simulink model "COMPONENT_MDL_Lag_QUAD_and_PEND_with_Ab"  (R2020b)
(part 10 of 12)

_Psi_D-THE_Phi_D.*sin(THE_Theta))))./2.0+(cg_to_mot_L.*cos(THE_Psi).*cos(THE_Theta).*(THE_Theta_D.*cos(THE_Psi)+THE_Phi_D.*cos(THE_Theta).*sin(THE_Psi)))./2.0)+THE_Psi_D.*cg_to_mot_H.*mprop.*cos(THE_Psi).*cos(THE_Theta).*(THE_Z_D./2.0-(cg_to_mot_H.*sin(THE_Theta).*(THE_Theta_D.*cos(THE_Psi)+THE_Phi_D.*cos(THE_Theta).*sin(THE_Psi)))./2.0+(cos(THE_Theta).*sin(THE_Psi).*(cg_to_mot_L.*(THE_Theta_D.*sin(THE_Psi)-THE_Phi_D.*cos(THE_Psi).*cos(THE_Theta))-cg_to_mot_H.*(THE_Psi_D-THE_Phi_D.*sin(THE_Theta))))./2.0+(cg_to_mot_L.*cos(THE_Psi).*cos(THE_Theta).*(THE_Theta_D.*cos(THE_Psi)+THE_Phi_D.*cos(THE_Theta).*sin(THE_Psi)))./2.0)+(THE_Theta_D.*cg_to_mot_H.*mprop.*sin(THE_Psi).*sin(THE_Theta).*(-THE_Z_D+cg_to_mot_H.*sin(THE_Theta).*(THE_Theta_D.*cos(THE_Psi)+THE_Phi_D.*cos(THE_Theta).*sin(THE_Psi))+cos(THE_Theta).*sin(THE_Psi).*(cg_to_mot_L.*(THE_Theta_D.*sin(THE_Psi)-THE_Phi_D.*cos(THE_Psi).*cos(THE_Theta))+cg_to_mot_H.*(THE_Psi_D-THE_Phi_D.*sin(THE_Theta)))+cg_to_mot_L.*cos(THE_Psi).*cos(THE_Theta).*(THE_Theta_D.*cos(THE_Psi)+THE_Phi_D.*cos(THE_Theta).*sin(THE_Psi))))./2.0+THE_Theta_D.*cg_to_mot_H.*mprop.*sin(THE_Psi).*sin(THE_Theta).*(THE_Z_D.*(-1.0./2.0)+(cg_to_mot_H.*sin(THE_Theta).*(THE_Theta_D.*cos(THE_Psi)+THE_Phi_D.*cos(THE_Theta).*sin(THE_Psi)))./2.0+(cos(THE_Theta).*sin(THE_Psi).*(cg_to_mot_L.*(THE_Theta_D.*sin(THE_Psi)-THE_Phi_D.*cos(THE_Psi).*cos(THE_Theta))+cg_to_mot_H.*(THE_Psi_D-THE_Phi_D.*sin(THE_Theta))))./2.0+(cg_to_mot_L.*cos(THE_Psi).*cos(THE_Theta).*(THE_Theta_D.*cos(THE_Psi)+THE_Phi_D.*cos(THE_Theta).*sin(THE_Psi)))./2.0)-THE_Theta_D.*cg_to_mot_H.*mprop.*sin(THE_Psi).*sin(THE_Theta).*(THE_Z_D./2.0-(cg_to_mot_H.*sin(THE_Theta).*(THE_Theta_D.*cos(THE_Psi)+THE_Phi_D.*cos(THE_Theta).*sin(THE_Psi)))./2.0+(cos(THE_Theta).*sin(THE_Psi).*(cg_to_mot_L.*(THE_Theta_D.*sin(THE_Psi)-THE_Phi_D.*cos(THE_Psi).*cos(THE_Theta))-cg_to_mot_H.*(THE_Psi_D-THE_Phi_D.*sin(THE_Theta))))./2.0+(cg_to_mot_L.*cos(THE_Psi).*cos(THE_Theta).*(THE_Theta_D.*cos(THE_Psi)+THE_Phi_D.*cos(THE_Theta).*sin(THE_Psi)))./2.0);Tbz_1.*(sin(THE_Phi).*sin(THE_Psi)+cos(THE_Phi).*cos(THE_Psi).*sin(THE_Theta))+Tbz_2.*(sin(THE_Phi).*sin(THE_Psi)+cos(THE_Phi).*cos(THE_Psi).*sin(THE_Theta))+Tbz_3.*(sin(THE_Phi).*sin(THE_Psi)+cos(THE_Phi).*cos(THE_Psi).*sin(THE_Theta))+Tbz_4.*(sin(THE_Phi).*sin(THE_Psi)+cos(THE_Phi).*cos(THE_Psi).*sin(THE_Theta))+(mprop.*(cos(THE_Phi).*cos(THE_Theta).*(cg_to_mot_H.*(THE_Psi_D.*THE_Theta_D.*sin(THE_Psi)-THE_Phi_D.*THE_Psi_D.*cos(THE_Psi).*cos(THE_Theta)+THE_Phi_D.*THE_Theta_D.*sin(THE_Psi).*sin(THE_Theta))-cg_to_mot_L.*(THE_Psi_D.*THE_Theta_D.*cos(THE_Psi)+THE_Phi_D.*THE_Psi_D.*cos(THE_Theta).*sin(THE_Psi)+THE_Phi_D.*THE_Theta_D.*cos(THE_Psi).*sin(THE_Theta)))-cg_to_mot_L.*(THE_Psi_D-THE_Phi_D.*sin(THE_Theta)).*(THE_Phi_D.*cos(THE_Phi).*sin(THE_Psi)+THE_Psi_D.*cos(THE_Psi).*sin(THE_Phi)+THE_Theta_D.*cos(THE_Phi).*cos(THE_Psi).*cos(THE_Theta)-THE_Phi_D.*cos(THE_Psi).*sin(THE_Phi).*sin(THE_Theta)-THE_Psi_D.*cos(THE_Phi).*sin(THE_Psi).*sin(THE_Theta))+cg_to_mot_H.*(THE_Psi_D-THE_Phi_D.*sin(THE_Theta)).*(-THE_Phi_D.*cos(THE_Phi).*cos(THE_Psi)+THE_Psi_D.*sin(THE_Phi).*sin(THE_Psi)-THE_Phi_D.*sin(THE_Phi).*sin(THE_Psi).*sin(THE_Theta)+THE_Psi_D.*cos(THE_Phi).*cos(THE_Psi).*sin(THE_Theta)+THE_Theta_D.*cos(THE_Phi).*cos(THE_Theta).*sin(THE_Psi))+THE_Phi_D.*cos(THE_Theta).*sin(THE_Phi).*(cg_to_mot_H.*(THE_Theta_D.*cos(THE_Psi)+THE_Phi_D.*cos(THE_Theta).*sin(THE_Psi))+cg_to_mot_L.*(THE_Theta_D.*sin(THE_Psi)-THE_Phi_D.*cos(THE_Psi).*cos(THE_Theta)))+THE_Theta_D.*cos(THE_Phi).*sin(THE_Theta).*(cg_to_mot_H.*(THE_Theta_D.*cos(THE_Psi)+THE_Phi_D.*cos(THE_Theta).*sin(THE_Psi))+cg_to_mot_L.*(THE_Theta_D.*sin(THE_Psi)-THE_Phi_D.*cos(THE_Psi).*cos(THE_Theta)))+THE_Phi_D.*THE_Theta_D.*cg_to_mot_H.*cos(THE_Theta).*(cos(THE_Psi).*sin(THE_Phi)-cos(THE_Phi).*sin(THE_Psi).*sin(THE_Theta))+THE_Phi_D.*THE_Theta_D.*cg_to_mot_L.*cos(THE_Theta).*(sin(THE_Phi).*sin(THE_Psi)+cos(THE_Phi).*cos(THE_Psi).*sin(THE_Theta))))./2.0+(mprop.*(cos(THE_Phi).*cos(THE_Theta).*(cg_to_mot_H.*(THE_Psi_D.*THE_Theta_D.*sin(THE_Psi)-THE_Phi_D.*THE_Psi_D.*cos(THE_Psi).*cos(THE_Theta)+THE_Phi_D.*THE_Theta_D.*sin(THE_Psi).*sin(THE_Theta))+cg_to_mot_L.*(THE_Psi_D.*THE_Theta_D.*cos(THE_Psi)+THE_Phi_D.*THE_Psi_D.*cos(THE_Theta).*sin(THE_Psi)+THE_Phi_D.*THE_Theta_D.*cos(THE_Psi).*sin(THE_Theta)))+cg_to_mot_L.*(THE_Psi_D-THE_Phi_D.*sin(THE_Theta)).*(THE_Phi_D.*cos(THE_Phi).*sin(THE_Psi)+THE_Psi_D.*cos(THE_Psi).*sin(THE_Phi)+THE_Theta_D.*cos(THE_Phi).*cos(THE_Psi).*cos(THE_Theta)-THE_Phi_D.*cos(THE_Psi).*sin(THE_Phi).*sin(THE_Theta)-THE_Psi_D.*cos(THE_Phi).*sin(THE_Psi).*sin(THE_Theta))+cg_to_mot_H.*(THE_Psi_D-THE_Phi_D.*sin(THE_Theta)).*(-THE_Phi_D.*cos(THE_Phi).*cos(THE_Psi)+THE_Psi_D.*sin(THE_Phi).*sin(THE_Psi)-THE_Phi_D.*sin(THE_Phi).*sin(THE_Psi).*sin(THE_Theta)+THE_Psi_D.*cos(THE_Phi).*cos(THE_Psi).*sin(THE_Theta)+THE_Theta_D.*cos(THE_Phi).*cos(THE_Theta).*sin(THE_Psi))+THE_Phi_D.*cos(THE_Theta).*sin(THE_Phi).*(cg_to_mot_H.*(THE_Theta_D.*cos(THE_Psi)+THE_Phi_D.*cos(THE_Theta).*sin(THE_Psi))-cg_to_mot_L.*(THE_Theta_D.*sin(THE_Psi)-THE_Phi_D.*cos(THE_Psi).*cos(THE_Theta)))+THE_Theta_D.*cos(THE_Phi).*sin(THE_Theta).*(cg_to_mot_H.*(THE_Theta_D.*cos(THE_Psi)+THE_Phi_D.*cos(THE_Theta).*sin(THE_Psi))-cg_to_mot_L.*(THE_Theta_D.*sin(THE_Psi)-THE_Phi_D.*cos(THE_Psi).*cos(THE_Theta)))+THE_Phi_D.*THE_Theta_D.*cg_to_mot_H.*cos(THE_Theta).*(cos(THE_Psi).*sin(THE_Phi)-cos(THE_Phi).*sin(THE_Psi).*sin(THE_Theta))-THE_Phi_D.*THE_Theta_D.*cg_to_mot_L.*cos(THE_Theta).*(sin(THE_Phi).*sin(THE_Psi)+cos(THE_Phi).*cos(THE_Psi).*sin(THE_Theta))))./2.0+mprop.*((cos(THE_Phi).*cos(THE_Theta).*(cg_to_mot_H.*(THE_Psi_D.*THE_Theta_D.*sin(THE_Psi)-THE_Phi_D.*THE_Psi_D.*cos(THE_Psi).*cos(THE_Theta)+THE_Phi_D.*THE_Theta_D.*sin(THE_Psi).*sin(THE_Theta))-cg_to_mot_L.*(THE_Psi_D.*THE_Theta_D.*cos(THE_Psi)+THE_Phi_D.*THE_Psi_D.*cos(THE_Theta).*sin(THE_Psi)+THE_Phi_D.*THE_Theta_D.*cos(THE_Psi).*sin(THE_Theta))))./2.0-(cg_to_mot_L.*(THE_Psi_D-THE_Phi_D.*sin(THE_Theta)).*(THE_Phi_D.*cos(THE_Phi).*sin(THE_Psi)+THE_Psi_D.*cos(THE_Psi).*sin(THE_Phi)+THE_Theta_D.*cos(THE_Phi).*cos(THE_Psi).*cos(THE_Theta)-THE_Phi_D.*cos(THE_Psi).*sin(THE_Phi).*sin(THE_Theta)-THE_Psi_D.*cos(THE_Phi).*sin(THE_Psi).*sin(THE_Theta)))./2.0+(cg_to_mot_H.*(THE_Psi_D-THE_Phi_D.*sin(THE_Theta)).*(-THE_Phi_D.*cos(THE_Phi).*cos(THE_Psi)+THE_Psi_D.*sin(THE_Phi).*sin(THE_Psi)-THE_Phi_D.*sin(THE_Phi).*sin(THE_Psi).*sin(THE_Theta)+THE_Psi_D.*cos(THE_Phi).*cos(THE_Psi).*sin(THE_Theta)+THE_Theta_D.*cos(THE_Phi).*cos(THE_Theta).*sin(THE_Psi)))./2.0+(THE_Phi_D.*cos(THE_Theta).*sin(THE_Phi).*(cg_to_mot_H.*(THE_Theta_D.*cos(THE_Psi)+THE_Phi_D.*cos(THE_Theta).*sin(THE_Psi))+cg_to_mot_L.*(THE_Theta_D.*sin(THE_Psi)-THE_Phi_D.*cos(THE_Psi).*cos(THE_Theta))))./2.0+(THE_Theta_D.*cos(THE_Phi).*sin(THE_Theta).*(cg_to_mot_H.*(THE_Theta_D.*cos(THE_Psi)+THE_Phi_D.*cos(THE_Theta).*sin(THE_Psi))+cg_to_mot_L.*(THE_Theta_D.*sin(THE_Psi)-THE_Phi_D.*cos(THE_Psi).*cos(THE_Theta))))./2.0+(THE_Phi_D.*THE_Theta_D.*cg_to_mot_H.*cos(THE_Theta).*(cos(THE_Psi).*sin(THE_Phi)-cos(THE_Phi).*sin(THE_Psi).*sin(THE_Theta)))./2.0+(THE_Phi_D.*THE_Theta_D.*cg_to_mot_L.*cos(THE_Theta).*(sin(THE_Phi).*sin(THE_Psi)+cos(THE_Phi).*cos(THE_Psi).*sin(THE_Theta)))./2.0)+mprop.*((cos(THE_Phi).*cos(THE_Theta).*(cg_to_mot_H.*(THE_Psi_D.*THE_Theta_D.*sin(THE_Psi)-THE_Phi_D.*THE_Psi_D.*cos(THE_Psi).*cos(THE_Theta)+THE_Phi_D.*THE_Theta_D.*sin(THE_Psi).*sin(THE_Theta))+cg_to_mot_L.*(THE_Psi_D.*THE_Theta_D.*cos(THE_Psi)+THE_Phi_D.*THE_Psi_D.*cos(THE_Theta).*sin(THE_Psi)+THE_Phi_D.*THE_Theta_D.*cos(THE_Psi).*sin(THE_Theta))))./2.0+(cg_to_mot_L.*(THE_Psi_D-THE_Phi_D.*sin(THE_Theta)).*(THE_Phi_D.*cos(THE_Phi).*sin(THE_Psi)+THE_Psi_D.*cos(THE_Psi).*sin(THE_Phi)+THE_Theta_D.*cos(THE_Phi).*cos(THE_Psi).*cos(THE_Theta)-THE_Phi_D.*cos(THE_Psi).*sin(THE_Phi).*sin(THE_Theta)-THE_Psi_D.*cos(THE_Phi).*sin(THE_Psi).*sin(THE_Theta)))./2.0+(cg_to_mot_H.*(THE_Psi_D-THE_Phi_D.*sin(THE_Theta)).*(-THE_Phi_D.*cos(THE_Phi).*cos(THE_Psi)+THE_Psi_D.*sin(THE_Phi).*sin(THE_Psi)-THE_Phi_D.*sin(THE_Phi).*sin(THE_Psi).*sin(THE_Theta)+THE_Psi_D.*cos(THE_Phi).*cos(THE_Psi).*sin(THE_Theta)+THE_Theta_D.*cos(THE_Phi).*cos(THE_Theta).*sin(THE_Psi)))./2.0+(THE_Phi_D.*cos(THE_Theta).*sin(THE_Phi).*(cg_to_mot_H.*(THE_Theta_D.*cos(THE_Psi)+THE_Phi_D.*cos(THE_Theta).*sin(THE_Psi))-cg_to_mot_L.*(THE_Theta_D.*sin(THE_Psi)-THE_Phi_D.*cos(THE_Psi).*cos(THE_Theta))))./2.0+(THE_Theta_D.*cos(THE_Phi).*sin(THE_Theta).*(cg_to_mot_H.*(THE_Theta_D.*cos(THE_Psi)+THE_Phi_D.*cos(THE_Theta).*sin(THE_Psi))-cg_to_mot_L.*(THE_Theta_D.*sin(THE_Psi)-THE_Phi_D.*cos(THE_Psi).*cos(THE_Theta))))./2.0+(THE_Phi_D.*THE_Theta_D.*cg_to_mot_H.*cos(THE_Theta).*(cos(THE_Psi).*sin(THE_Phi)-cos(THE_Phi).*sin(THE_Psi).*sin(THE_Theta)))./2.0-(THE_Phi_D.*THE_Theta_D.*cg_to_mot_L.*cos(THE_Theta).*(sin(THE_Phi).*sin(THE_Psi)+cos(THE_Phi).*cos(THE_Psi).*sin(THE_Theta)))./2.0)+(mprop.*((cg_to_mot_L.*(THE_Theta_D.*sin(THE_Psi)-THE_Phi_D.*cos(THE_Psi).*cos(THE_Theta))+cg_to_mot_H.*(THE_Psi_D-THE_Phi_D.*sin(THE_Theta))).*(-THE_Phi_D.*cos(THE_Phi).*cos(THE_Psi)+THE_Psi_D.*sin(THE_Phi).*sin(THE_Psi)-THE_Phi_D.*sin(THE_Phi).*sin(THE_Psi).*sin(THE_Theta)+THE_Psi_D.*cos(THE_Phi).*cos(THE_Psi).*sin(THE_Theta)+THE_Theta_D.*cos(THE_Phi).*cos(THE_Theta).*sin(THE_Psi))-(cg_to_mot_L.*(THE_Psi_D.*THE_Theta_D.*cos(THE_Psi)+THE_Phi_D.*THE_Psi_D.*cos(THE_Theta).*sin(THE_Psi)+THE_Phi_D.*THE_Theta_D.*cos(THE_Psi).*sin(THE_Theta))-THE_Phi_D.*THE_Theta_D.*cg_to_mot_H.*cos(THE_Theta)).*(cos(THE_Psi).*sin(THE_Phi)-cos(THE_Phi).*sin(THE_Psi).*sin(THE_Theta))+cg_to_mot_L.*(THE_Theta_D.*cos(THE_Psi)+THE_Phi_D.*cos(THE_Theta).*sin(THE_Psi)).*(THE_Phi_D.*cos(THE_Phi).*sin(THE_Psi)+THE_Psi_D.*cos(THE_Psi).*sin(THE_Phi)+THE_Theta_D.*cos(THE_Phi).*cos(THE_Psi).*cos(THE_Theta)-THE_Phi_D.*cos(THE_Psi).*sin(THE_Phi).*sin(THE_Theta)-THE_Psi_D.*cos(THE_Phi).*sin(THE_Psi).*sin(THE_Theta))-cg_to_mot_L.*(sin(THE_Phi).*sin(THE_Psi)+cos(THE_Phi).*cos(THE_Psi).*sin(THE_Theta)).*(THE_Psi_D.*THE_Theta_D.*sin(THE_Psi)-THE_Phi_D.*THE_Psi_D.*cos(THE_Psi).*cos(THE_Theta)+THE_Phi_D.*THE_Theta_D.*sin(THE_Psi).*sin(THE_Theta))+cg_to_mot_H.*cos(THE_Phi).*cos(THE_Theta).*(THE_Psi_D.*THE_Theta_D.*sin(THE_Psi)-THE_Phi_D.*THE_Psi_D.*cos(THE_Psi).*cos(THE_Theta)+THE_Phi_D.*THE_Theta_D.*sin(THE_Psi).*sin(THE_Theta))+THE_Phi_D.*cg_to_mot_H.*cos(THE_Theta).*sin(THE_Phi).*(THE_Theta_D.*cos(THE_Psi)+THE_Phi_D.*cos(THE_Theta).*sin(THE_Psi))+THE_Theta_D.*cg_to_mot_H.*cos(THE_Phi).*sin(THE_Theta).*(THE_Theta_D.*cos(THE_Psi)+THE_Phi_D.*cos(THE_Theta).*sin(THE_Psi))))./2.0+(mprop.*(-(cg_to_mot_L.*(THE_Theta_D.*sin(THE_Psi)-THE_Phi_D.*cos(THE_Psi).*cos(THE_Theta))-cg_to_mot_H.*(THE_Psi_D-THE_Phi_D.*sin(THE_Theta))).*(-THE_Phi_D.*cos(THE_Phi).*cos(THE_Psi)+THE_Psi_D.*sin(THE_Phi).*sin(THE_Psi)-THE_Phi_D.*sin(THE_Phi).*sin(THE_Psi).*sin(THE_Theta)+THE_Psi_D.*cos(THE_Phi).*cos(THE_Psi).*sin(THE_Theta)+THE_Theta_D.*cos(THE_Phi).*cos(THE_Theta).*sin(THE_Psi))+(cg_to_mot_L.*(THE_Psi_D.*THE_Theta_D.*cos(THE_Psi)+THE_Phi_D.*THE_Psi_D.*cos(THE_Theta).*sin(THE_Psi)+THE_Phi_D.*THE_Theta_D.*cos(THE_Psi).*sin(THE_Theta))+THE_Phi_D.*THE_Theta_D.*cg_to_mot_H.*cos(THE_Theta)).*(cos(THE_Psi).*sin(THE_Phi)-cos(THE_Phi).*sin(THE_Psi).*sin(THE_Theta))-cg_to_mot_L.*(THE_Theta_D.*cos(THE_Psi)+THE_Phi_D.*cos(THE_Theta).*sin(THE_Psi)).*(THE_Phi_D.*cos(THE_Phi).*sin(THE_Psi)+THE_Psi_D.*cos(THE_Psi).*sin(THE_Phi)+THE_Theta_D.*cos(THE_Phi).*cos(THE_Psi).*cos(THE_Theta)-THE_Phi_D.*cos(THE_Psi).*sin(THE_Phi).*sin(THE_Theta)-THE_Psi_D.*cos(THE_Phi).*sin(THE_Psi).*sin(THE_Theta))+cg_to_mot_L.*(sin(THE_Phi).*sin(THE_Psi)+cos(THE_Phi).*cos(THE_Psi).*sin(THE_Theta)).*(THE_Psi_D.*THE_Theta_D.*sin(THE_Psi)-THE_Phi_D.*THE_Psi_D.*cos(THE_Psi).*cos(THE_Theta)+THE_Phi_D.*THE_Theta_D.*sin(THE_Psi).*sin(THE_Theta))+cg_to_mot_H.*cos(THE_Phi).*cos(THE_Theta).*(THE_Psi_D.*THE_Theta_D.*sin(THE_Psi)-THE_Phi_D.*THE_Psi_D.*cos(THE_Psi).*cos(THE_Theta)+THE_Phi_D.*THE_Theta_D.*sin(THE_Psi).*sin(THE_Theta))+THE_Phi_D.*cg_to_mot_H.*cos(THE_Theta).*sin(THE_Phi).*(THE_Theta_D.*cos(THE_Psi)+THE_Phi_D.*cos(THE_Theta).*sin(THE_Psi))+THE_Theta_D.*cg_to_mot_H.*cos(THE_Phi).*sin(THE_Theta).*(THE_Theta_D.*cos(THE_Psi)+THE_Phi_D.*cos(THE_Theta).*sin(THE_Psi))))./2.0+mprop.*(((cg_to_mot_L.*(THE_Theta_D.*sin(THE_Psi)-THE_Phi_D.*cos(THE_Psi).*cos(THE_Theta))+cg_to_mot_H.*(THE_Psi_D-THE_Phi_D.*sin(THE_Theta))).*(-THE_Phi_D.*cos(THE_Phi).*cos(THE_Psi)+THE_Psi_D.*sin(THE_Phi).*sin(THE_Psi)-THE_Phi_D.*sin(THE_Phi).*sin(THE_Psi).*sin(THE_Theta)+THE_Psi_D.*cos(THE_Phi).*cos(THE_Psi).*sin(THE_Theta)+THE_Theta_D.*cos(THE_Phi).*cos(THE_Theta).*sin(THE_Psi)))./2.0-((cg_to_mot_L.*(THE_Psi_D.*THE_Theta_D.*cos(THE_Psi)+THE_Phi_D.*THE_Psi_D.*cos(THE_Theta).*sin(THE_Psi)+THE_Phi_D.*THE_Theta_D.*cos(THE_Psi).*sin(THE_Theta))-THE_Phi_D.*THE_Theta_D.*cg_to_mot_H.*cos(THE_Theta)).*(cos(THE_Psi).*sin(THE_Phi)-cos(THE_Phi).*sin(THE_Psi).*sin(THE_Theta)))./2.0+(cg_to_mot_L.*(THE_Theta_D.*cos(THE_Psi)+THE_Phi_D.*cos(THE_Theta).*sin(THE_Psi)).*(THE_Phi_D.*cos(THE_Phi).*sin(THE_Psi)+THE_Psi_D.*cos(THE_Psi).*sin(THE_Phi)+THE_Theta_D.*cos(THE_Phi).*cos(THE_Psi).*cos(THE_Theta)-THE_Phi_D.*cos(THE_Psi).*sin(THE_Phi).*sin(THE_Theta)-THE_Psi_D.*cos(THE_Phi).*sin(THE_Psi).*sin(THE_Theta)))./2.0-(cg_to_mot_L.*(sin(THE_Phi).*sin(THE_Psi)+cos(THE_Phi).*cos(THE_Psi).*sin(THE_Theta)).*(THE_Psi_D.*THE_Theta_D.*sin(THE_Psi)-THE_Phi_D.*THE_Psi_D.*cos(THE_Psi).*cos(THE_Theta)+THE_Phi_D.*THE_Theta_D.*sin(THE_Psi).*sin(THE_Theta)))./2.0+(cg_to_mot_H.*cos(THE_Phi).*cos(THE_Theta).*(THE_Psi_D.*THE_Theta_D.*sin(THE_Psi)-THE_Phi_D.*THE_Psi_D.*cos(THE_Psi).*cos(THE_Theta)+THE_Phi_D.*THE_Theta_D.*sin(THE_Psi).*sin(THE_Theta)))./2.0+(THE_Phi_D.*cg_to_mot_H.*cos(THE_Theta).*sin(THE_Phi).*(THE_Theta_D.*cos(THE_Psi)+THE_Phi_D.*cos(THE_Theta).*sin(THE_Psi)))./2.0+(THE_Theta_D.*cg_to_mot_H.*cos(THE_Phi).*sin(THE_Theta).*(THE_Theta_D.*cos(THE_Psi)+THE_Phi_D.*cos(THE_Theta).*sin(THE_Psi)))./2.0)+mprop.*((cg_to_mot_L.*(THE_Theta_D.*sin(THE_Psi)-THE_Phi_D.*cos(THE_Psi).*cos(THE_Theta))-cg_to_mot_H.*(THE_Psi_D-THE_Phi_D.*sin(THE_Theta))).*(-THE_Phi_D.*cos(THE_Phi).*cos(THE_Psi)+THE_Psi_D.*sin(THE_Phi).*sin(THE_Psi)-THE_Phi_D.*sin(THE_Phi).*sin(THE_Psi).*sin(THE_Theta)+THE_Psi_D.*cos(THE_Phi).*cos(THE_Psi).*sin(THE_Theta)+THE_Theta_D.*cos(THE_Phi).*cos(THE_Theta).*sin(THE_Psi)).*(-1.0./2.0)+((cg_to_mot_L.*(THE_Psi_D.*THE_Theta_D.*cos(THE_Psi)+THE_Phi_D.*THE_Psi_D.*cos(THE_Theta).*sin(THE_Psi)+THE_Phi_D.*THE_Theta_D.*cos(THE_Psi).*sin(THE_Theta))+THE_Phi_D.*THE_Theta_D.*cg_to_mot_H.*cos(THE_Theta)).*(cos(THE_Psi).*sin(THE_Phi)-cos(THE_Phi).*sin(THE_Psi).*sin(THE_Theta)))./2.0-(cg_to_mot_L.*(THE_Theta_D.*cos(THE_Psi)+THE_Phi_D.*cos(THE_Theta).*sin(THE_Psi)).*(THE_Phi_D.*cos(THE_Phi).*sin(THE_Psi)+THE_Psi_D.*cos(THE_Psi).*sin(THE_Phi)+THE_Theta_D.*cos(THE_Phi).*cos(THE_Psi).*cos(THE_Theta)-THE_Phi_D.*cos(THE_Psi).*sin(THE_Phi).*sin(THE_Theta)-THE_Psi_D.*cos(THE_Phi).*sin(THE_Psi).*sin(THE_Theta)))./2.0+(cg_to_mot_L.*(sin(THE_Phi).*sin(THE_Psi)+cos(THE_Phi).*cos(THE_Psi).*sin(THE_Theta)).*(THE_Psi_D.*THE_Theta_D.*sin(THE_Psi)-THE_Phi_D.*THE_Psi_D.*cos(THE_Psi).*cos(THE_Theta)+THE_Phi_D.*THE_Theta_D.*sin(THE_Psi).*sin(THE_Theta)))./2.0+(cg_to_mot_H.*cos(THE_Phi).*cos(THE_Theta).*(THE_Psi_D.*THE_Theta_D.*sin(THE_Psi)-THE_Phi_D.*THE_Psi_D.*cos(THE_Psi).*cos(THE_Theta)+THE_Phi_D.*THE_Theta_D.*sin(THE_Psi).*sin(THE_Theta)))./2.0+(THE_Phi_D.*cg_to_mot_H.*cos(THE_Theta).*sin(THE_Phi).*(THE_Theta_D.*cos(THE_Psi)+THE_Phi_D.*cos(THE_Theta).*sin(THE_Psi)))./2.0+(THE_Theta_D.*cg_to_mot_H.*cos(THE_Phi).*sin(THE_Theta).*(THE_Theta_D.*cos(THE_Psi)+THE_Phi_D.*cos(THE_Theta).*sin(THE_Psi)))./2.0)+(m_pend.*((Tv_Z_pend+(Lz_pend.*cos(THE_Psi_pend).*cos(THE_Theta_pend))./2.0).*(THE_Phi_D.^2.*sin(THE_Phi).*sin(THE_Psi)+THE_Psi_D.^2.*sin(THE_Phi).*sin(THE_Psi)+THE_Phi_D.^2.*cos(THE_Phi).*cos(THE_Psi).*sin(THE_Theta)+THE_Psi_D.^2.*cos(THE_Phi).*cos(THE_Psi).*sin(THE_Theta)+THE_Theta_D.^2.*cos(THE_Phi).*cos(THE_Psi).*sin(THE_Theta)-THE_Phi_D.*THE_Psi_D.*cos(THE_Phi).*cos(THE_Psi).*2.0+THE_Phi_D.*THE_Theta_D.*cos(THE_Psi).*cos(THE_Theta).*sin(THE_Phi).*2.0+THE_Psi_D.*THE_Theta_D.*cos(THE_Phi).*cos(THE_Theta).*sin(THE_Psi).*2.0-THE_Phi_D.*THE_Psi_D.*sin(THE_Phi).*sin(THE_Psi).*sin(THE_Theta).*2.0)+(sin(THE_Phi).*sin(THE_Psi)+cos(THE_Phi).*cos(THE_Psi).*sin(THE_Theta)).*((Lz_pend.*THE_Psi_pend_D.^2.*cos(THE_Psi_pend).*cos(THE_Theta_pend))./2.0+(Lz_pend.*THE_Theta_pend_D.^2.*cos(THE_Psi_pend).*cos(THE_Theta_pend))./2.0-Lz_pend.*THE_Psi_pend_D.*THE_Theta_pend_D.*sin(THE_Psi_pend).*sin(THE_Theta_pend))+((Lz_pend.*THE_Psi_pend_D.*cos(THE_Theta_pend).*sin(THE_Psi_pend))./2.0+(Lz_pend.*THE_Theta_pend_D.*cos(THE_Psi_pend).*sin(THE_Theta_pend))./2.0).*(THE_Phi_D.*cos(THE_Phi).*sin(THE_Psi)+THE_Psi_D.*cos(THE_Psi).*sin(THE_Phi)+THE_Theta_D.*cos(THE_Phi).*cos(THE_Psi).*cos(THE_Theta)-THE_Phi_D.*cos(THE_Psi).*sin(THE_Phi).*sin(THE_Theta)-THE_Psi_D.*cos(THE_Phi).*sin(THE_Psi).*sin(THE_Theta)).*2.0-(Lz_pend.*(cos(THE_Phi_pend).*sin(THE_Psi_pend)-cos(THE_Psi_pend).*sin(THE_Phi_pend).*sin(THE_Theta_pend)).*(-THE_Phi_D.^2.*cos(THE_Psi).*sin(THE_Phi)-THE_Psi_D.^2.*cos(THE_Psi).*sin(THE_Phi)+THE_Phi_D.^2.*cos(THE_Phi).*sin(THE_Psi).*sin(THE_Theta)+THE_Psi_D.^2.*cos(THE_Phi).*sin(THE_Psi).*sin(THE_Theta)+THE_Theta_D.^2.*cos(THE_Phi).*sin(THE_Psi).*sin(THE_Theta)-THE_Phi_D.*THE_Psi_D.*cos(THE_Phi).*sin(THE_Psi).*2.0-THE_Psi_D.*THE_Theta_D.*cos(THE_Phi).*cos(THE_Psi).*cos(THE_Theta).*2.0+THE_Phi_D.*THE_Psi_D.*cos(THE_Psi).*sin(THE_Phi).*sin(THE_Theta).*2.0+THE_Phi_D.*THE_Theta_D.*cos(THE_Theta).*sin(THE_Phi).*sin(THE_Psi).*2.0))./2.0-(Lz_pend.*(cos(THE_Psi).*sin(THE_Phi)-cos(THE_Phi).*sin(THE_Psi).*sin(THE_Theta)).*(-THE_Phi_pend_D.^2.*cos(THE_Phi_pend).*sin(THE_Psi_pend)-THE_Psi_pend_D.^2.*cos(THE_Phi_pend).*sin(THE_Psi_pend)+THE_Phi_pend_D.^2.*cos(THE_Psi_pend).*sin(THE_Phi_pend).*sin(THE_Theta_pend)+THE_Psi_pend_D.^2.*cos(THE_Psi_pend).*sin(THE_Phi_pend).*sin(THE_Theta_pend)+THE_Theta_pend_D.^2.*cos(THE_Psi_pend).*sin(THE_Phi_pend).*sin(THE_Theta_pend)-THE_Phi_pend_D.*THE_Psi_pend_D.*cos(THE_Psi_pend).*sin(THE_Phi_pend).*2.0-THE_Phi_pend_D.*THE_Theta_pend_D.*cos(THE_Phi_pend).*cos(THE_Psi_pend).*cos(THE_Theta_pend).*2.0+THE_Phi_pend_D.*THE_Psi_pend_D.*cos(THE_Phi_pend).*sin(THE_Psi_pend).*sin(THE_Theta_pend).*2.0+THE_Psi_pend_D.*THE_Theta_pend_D.*cos(THE_Theta_pend).*sin(THE_Phi_pend).*sin(THE_Psi_pend).*2.0))./2.0-Lz_pend.*(-THE_Phi_D.*cos(THE_Phi).*cos(THE_Psi)+THE_Psi_D.*sin(THE_Phi).*sin(THE_Psi)-THE_Phi_D.*sin(THE_Phi).*sin(THE_Psi).*sin(THE_Theta)+THE_Psi_D.*cos(THE_Phi).*cos(THE_Psi).*sin(THE_Theta)+THE_Theta_D.*cos(THE_Phi).*cos(THE_Theta).*sin(THE_Psi)).*(-THE_Psi_pend_D.*cos(THE_Phi_pend).*cos(THE_Psi_pend)+THE_Phi_pend_D.*sin(THE_Phi_pend).*sin(THE_Psi_pend)-THE_Psi_pend_D.*sin(THE_Phi_pend).*sin(THE_Psi_pend).*sin(THE_Theta_pend)+THE_Phi_pend_D.*cos(THE_Phi_pend).*cos(THE_Psi_pend).*sin(THE_Theta_pend)+THE_Theta_pend_D.*cos(THE_Psi_pend).*cos(THE_Theta_pend).*sin(THE_Phi_pend))+(Lz_pend.*cos(THE_Phi).*cos(THE_Theta).*(THE_Phi_pend_D.^2.*sin(THE_Phi_pend).*sin(THE_Psi_pend)+THE_Psi_pend_D.^2.*sin(THE_Phi_pend).*sin(THE_Psi_pend)+THE_Phi_pend_D.^2.*cos(THE_Phi_pend).*cos(THE_Psi_pend).*sin(THE_Theta_pend)+THE_Psi_pend_D.^2.*cos(THE_Phi_pend).*cos(THE_Psi_pend).*sin(THE_Theta_pend)+THE_Theta_pend_D.^2.*cos(THE_Phi_pend).*cos(THE_Psi_pend).*sin(THE_Theta_pend)-THE_Phi_pend_D.*THE_Psi_pend_D.*cos(THE_Phi_pend).*cos(THE_Psi_pend).*2.0+THE_Phi_pend_D.*THE_Theta_pend_D.*cos(THE_Psi_pend).*cos(THE_Theta_pend).*sin(THE_Phi_pend).*2.0+THE_Psi_pend_D.*THE_Theta_pend_D.*cos(THE_Phi_pend).*cos(THE_Theta_pend).*sin(THE_Psi_pend).*2.0-THE_Phi_pend_D.*THE_Psi_pend_D.*sin(THE_Phi_pend).*sin(THE_Psi_pend).*sin(THE_Theta_pend).*2.0))./2.0+Lz_pend.*THE_Phi_D.*cos(THE_Theta).*sin(THE_Phi).*(THE_Phi_pend_D.*cos(THE_Phi_pend).*sin(THE_Psi_pend)+THE_Psi_pend_D.*cos(THE_Psi_pend).*sin(THE_Phi_pend)+THE_Theta_pend_D.*cos(THE_Phi_pend).*cos(THE_Psi_pend).*cos(THE_Theta_pend)-THE_Phi_pend_D.*cos(THE_Psi_pend).*sin(THE_Phi_pend).*sin(THE_Theta_pend)-THE_Psi_pend_D.*cos(THE_Phi_pend).*sin(THE_Psi_pend).*sin(THE_Theta_pend))+Lz_pend.*THE_Theta_D.*cos(THE_Phi).*sin(THE_Theta).*(THE_Phi_pend_D.*cos(THE_Phi_pend).*sin(THE_Psi_pend)+THE_Psi_pend_D.*cos(THE_Psi_pend).*sin(THE_Phi_pend)+THE_Theta_pend_D.*cos(THE_Phi_pend).*cos(THE_Psi_pend).*cos(THE_Theta_pend)-THE_Phi_pend_D.*cos(THE_Psi_pend).*sin(THE_Phi_pend).*sin(THE_Theta_pend)-THE_Psi_pend_D.*cos(THE_Phi_pend).*sin(THE_Psi_pend).*sin(THE_Theta_pend))+(Lz_pend.*THE_Phi_D.^2.*cos(THE_Phi).*cos(THE_Theta).*(sin(THE_Phi_pend).*sin(THE_Psi_pend)+cos(THE_Phi_pend).*cos(THE_Psi_pend).*sin(THE_Theta_pend)))./2.0+(Lz_pend.*THE_Theta_D.^2.*cos(THE_Phi).*cos(THE_Theta).*(sin(THE_Phi_pend).*sin(THE_Psi_pend)+cos(THE_Phi_pend).*cos(THE_Psi_pend).*sin(THE_Theta_pend)))./2.0-Lz_pend.*THE_Phi_D.*THE_Theta_D.*sin(THE_Phi).*sin(THE_Theta).*(sin(THE_Phi_pend).*sin(THE_Psi_pend)+cos(THE_Phi_pend).*cos(THE_Psi_pend).*sin(THE_Theta_pend))))./2.0+m_pend.*(((Tv_Z_pend+(Lz_pend.*cos(THE_Psi_pend).*cos(THE_Theta_pend))./2.0).*(THE_Phi_D.^2.*sin(THE_Phi).*sin(THE_Psi)+THE_Psi_D.^2.*sin(THE_Phi).*sin(THE_Psi)+THE_Phi_D.^2.*cos(THE_Phi).*cos(THE_Psi).*sin(THE_Theta)+THE_Psi_D.^2.*cos(THE_Phi).*cos(THE_Psi).*sin(THE_Theta)+THE_Theta_D.^2.*cos(THE_Phi).*cos(THE_Psi).*sin(THE_Theta)-THE_Phi_D.*THE_Psi_D.*cos(THE_Phi).*cos(THE_Psi).*2.0+THE_Phi_D.*THE_Theta_D.*cos(THE_Psi).*cos(THE_Theta).*sin(THE_Phi).*2.0+THE_Psi_D.*THE_Theta_D.*cos(THE_Phi).*cos(THE_Theta).*sin(THE_Psi).*2.0-THE_Phi_D.*THE_Psi_D.*sin(THE_Phi).*sin(THE_Psi).*sin(THE_Theta).*2.0))./2.0+((sin(THE_Phi).*sin(THE_Psi)+cos(THE_Phi).*cos(THE_Psi).*sin(THE_Theta)).*((Lz_pend.*THE_Psi_pend_D.^2.*cos(THE_Psi_pend).*cos(THE_Theta_pend))./2.0+(Lz_pend.*THE_Theta_pend_D.^2.*cos(THE_Psi_pend).*cos(THE_Theta_pend))./2.0-Lz_pend.*THE_Psi_pend_D.*THE_Theta_pend_D.*sin(THE_Psi_pend).*sin(THE_Theta_pend)))./2.0+((Lz_pend.*THE_Psi_pend_D.*cos(THE_Theta_pend).*sin(THE_Psi_pend))./2.0+(Lz_pend.*THE_Theta_pend_D.*cos(THE_Psi_pend).*sin(THE_Theta_pend))./2.0).*(THE_Phi_D.*cos(THE_Phi).*sin(THE_Psi)+THE_Psi_D.*cos(THE_Psi).*sin(THE_Phi)+THE_Theta_D.*cos(THE_Phi).*cos(THE_Psi).*cos(THE_Theta)-THE_Phi_D.*cos(THE_Psi).*sin(THE_Phi).*sin(THE_Theta)-THE_Psi_D.*cos(THE_Phi).*sin(THE_Psi).*sin(THE_Theta))-(Lz_pend.*(cos(THE_Phi_pend).*sin(THE_Psi_pend)-cos(THE_Psi_pend).*sin(THE_Phi_pend).*sin(THE_Theta_pend)).*(-THE_Phi_D.^2.*cos(THE_Psi).*sin(THE_Phi)-THE_Psi_D.^2.*cos(THE_Psi).*sin(THE_Phi)+THE_Phi_D.^2.*cos(THE_Phi).*sin(THE_Psi).*sin(THE_Theta)+THE_Psi_D.^2.*cos(THE_Phi).*sin(THE_Psi).*sin(THE_Theta)+THE_Theta_D.^2.*cos(THE_Phi).*sin(THE_Psi).*sin(THE_Theta)-THE_Phi_D.*THE_Psi_D.*cos(THE_Phi).*sin(THE_Psi).*2.0-THE_Psi_D.*THE_Theta_D.*cos(THE_Phi).*cos(THE_Psi).*cos(THE_Theta).*2.0+THE_Phi_D.*THE_Psi_D.*cos(THE_Psi).*sin(THE_Phi).*sin(THE_Theta).*2.0+THE_Phi_D.*THE_Theta_D.*cos(THE_Theta).*sin(THE_Phi).*sin(THE_Psi).*2.0))./4.0-(Lz_pend.*(cos(THE_Psi).*sin(THE_Phi)-cos(THE_Phi).*sin(THE_Psi).*sin(THE_Theta)).*(-THE_Phi_pend_D.^2.*cos(THE_Phi_pend).*sin(THE_Psi_pend)-THE_Psi_pend_D.^2.*cos(THE_Phi_pend).*sin(THE_Psi_pend)+THE_Phi_pend_D.^2.*cos(THE_Psi_pend).*sin(THE_Phi_pend).*sin(THE_Theta_pend)+THE_Psi_pend_D.^2.*cos(THE_Psi_pend).*sin(THE_Phi_pend).*sin(THE_Theta_pend)+THE_Theta_pend_D.^2.*cos(THE_Psi_pend).*sin(THE_Phi_pend).*sin(THE_Theta_pend)-THE_Phi_pend_D.*THE_Psi_pend_D.*cos(THE_Psi_pend).*sin(THE_Phi_pend).*2.0-THE_Phi_pend_D.*THE_Theta_pend_D.*cos(THE_Phi_pend).*cos(THE_Psi_pend).*cos(THE_Theta_pend).*2.0+THE_Phi_pend_D.*THE_Psi_pend_D.*cos(THE_Phi_pend).*sin(THE_Psi_pend).*sin(THE_Theta_pend).*2.0+THE_Psi_pend_D.*THE_Theta_pend_D.*cos(THE_Theta_pend).*sin(THE_Phi_pend).*sin(THE_Psi_pend).*2.0))./4.0-(Lz_pend.*(-THE_Phi_D.*cos(THE_Phi).*cos(THE_Psi)+THE_Psi_D.*sin(THE_Phi).*sin(THE_Psi)-THE_Phi_D.*sin(THE_Phi).*sin(THE_Psi).*sin(THE_Theta)+THE_Psi_D.*cos(THE_Phi).*cos(THE_Psi).*sin(THE_Theta)+THE_Theta_D.*cos(THE_Phi).*cos(THE_Theta).*sin(THE_Psi)).*(-THE_Psi_pend_D.*cos(THE_Phi_pend).*cos(THE_Psi_pend)+THE_Phi_pend_D.*sin(THE_Phi_pend).*sin(THE_Psi_pend)-THE_Psi_pend_D.*sin(THE_Phi_pend).*sin(THE_Psi_pend).*sin(THE_Theta_pend)+THE_Phi_pend_D.*cos(THE_Phi_pend).*cos(THE_Psi_pend).*sin(THE_Theta_pend)+THE_Theta_pend_D.*cos(THE_Psi_pend).*cos(THE_Theta_pend).*sin(THE_Phi_pend)))./2.0+(Lz_pend.*cos(THE_Phi).*cos(THE_Theta).*(THE_Phi_pend_D.^2.*sin(THE_Phi_pend).*sin(THE_Psi_pend)+THE_Psi_pend_D.^2.*sin(THE_Phi_pend).*sin(THE_Psi_pend)+THE_Phi_pend_D.^2.*cos(THE_Phi_pend).*cos(THE_Psi_pend).*sin(THE_Theta_pend)+THE_Psi_pend_D.^2.*cos(THE_Phi_pend).*cos(THE_Psi_pend).*sin(THE_Theta_pend)+THE_Theta_pend_D.^2.*cos(THE_Phi_pend).*cos(THE_Psi_pend).*sin(THE_Theta_pend)-THE_Phi_pend_D.*THE_Psi_pend_D.*cos(THE_Phi_pend).*cos(THE_Psi_pend).*2.0+THE_Phi_pend_D.*THE_Theta_pend_D.*cos(THE_Psi_pend).*cos(THE_Theta_pend).*sin(THE_Phi_pend).*2.0+THE_Psi_pend_D.*THE_Theta_pend_D.*cos(THE_Phi_pend).*cos(THE_Theta_pend).*sin(THE_Psi_pend).*2.0-THE_Phi_pend_D.*THE_Psi_pend_D.*sin(THE_Phi_pend).*sin(THE_Psi_pend).*sin(THE_Theta_pend).*2.0))./4.0+(Lz_pend.*THE_Phi_D.*cos(THE_Theta).*sin(THE_Phi).*(THE_Phi_pend_D.*cos(THE_Phi_pend).*sin(THE_Psi_pend)+THE_Psi_pend_D.*cos(THE_Psi_pend).*sin(THE_Phi_pend)+THE_Theta_pend_D.*cos(THE_Phi_pend).*cos(THE_Psi_pend).*cos(THE_Theta_pend)-THE_Phi_pend_D.*cos(THE_Psi_pend).*sin(THE_Phi_pend).*sin(THE_Theta_pend)-THE_Psi_pend_D.*cos(THE_Phi_pend).*sin(THE_Psi_pend).*sin(THE_Theta_pend)))./2.0+(Lz_pend.*THE_Theta_D.*cos(THE_Phi).*sin(THE_Theta).*(THE_Phi_pend_D.*cos(THE_Phi_pend).*sin(THE_Psi_pend)+THE_Psi_pend_D.*cos(THE_Psi_pend).*sin(THE_Phi_pend)+THE_Theta_pend_D.*cos(THE_Phi_pend).*cos(THE_Psi_pend).*cos(THE_Theta_pend)-THE_Phi_pend_D.*cos(THE_Psi_pend).*sin(THE_Phi_pend).*sin(THE_Theta_pend)-THE_Psi_pend_D.*cos(THE_Phi_pend).*sin(THE_Psi_pend).*sin(THE_Theta_pend)))./2.0+(Lz_pend.*THE_Phi_D.^2.*cos(THE_Phi).*cos(THE_Theta).*(sin(THE_Phi_pend).*sin(THE_Psi_pend)+cos(THE_Phi_pend).*cos(THE_Psi_pend).*sin(THE_Theta_pend)))./4.0+(Lz_pend.*THE_Theta_D.^2.*cos(THE_Phi).*cos(THE_Theta).*(sin(THE_Phi_pend).*sin(THE_Psi_pend)+cos(THE_Phi_pend).*cos(THE_Psi_pend).*sin(THE_Theta_pend)))./4.0-(Lz_pend.*THE_Phi_D.*THE_Theta_D.*sin(THE_Phi).*sin(THE_Theta).*(sin(THE_Phi_pend).*sin(THE_Psi_pend)+cos(THE_Phi_pend).*cos(THE_Psi_pend).*sin(THE_Theta_pend)))./2.0);(mprop.*((cg_to_mot_L.*(THE_Theta_D.*sin(THE_Psi)-THE_Phi_D.*cos(THE_Psi).*cos(THE_Theta))+cg_to_mot_H.*(THE_Psi_D-THE_Phi_D.*sin(THE_Theta))).*(-THE_Phi_D.*cos(THE_Psi).*sin(THE_Phi)-THE_Psi_D.*cos(THE_Phi).*sin(THE_Psi)+THE_Phi_D.*cos(THE_Phi).*sin(THE_Psi).*sin(THE_Theta)+THE_Psi_D.*cos(THE_Psi).*sin(THE_Phi).*sin(THE_Theta)+THE_Theta_D.*cos(THE_Theta).*sin(THE_Phi).*sin(THE_Psi))+(cg_to_mot_L.*(THE_Psi_D.*THE_Theta_D.*cos(THE_Psi)+THE_Phi_D.*THE_Psi_D.*cos(THE_Theta).*sin(THE_Psi)+THE_Phi_D.*THE_Theta_D.*cos(THE_Psi).*sin(THE_Theta))-THE_Phi_D.*THE_Theta_D.*cg_to_mot_H.*cos(THE_Theta)).*(cos(THE_Phi).*cos(THE_Psi)+sin(THE_Phi).*sin(THE_Psi).*sin(THE_Theta))+cg_to_mot_L.*(THE_Theta_D.*cos(THE_Psi)+THE_Phi_D.*cos(THE_Theta).*sin(THE_Psi)).*(-THE_Psi_D.*cos(THE_Phi).*cos(THE_Psi)+THE_Phi_D.*sin(THE_Phi).*sin(THE_Psi)-THE_Psi_D.*sin(THE_Phi).*sin(THE_Psi).*sin(THE_Theta)+THE_Phi_D.*cos(THE_Phi).*cos(THE_Psi).*sin(THE_Theta)+THE_Theta_D.*cos(THE_Psi).*cos(THE_Theta).*sin(THE_Phi))+cg_to_mot_L.*(cos(THE_Phi).*sin(THE_Psi)-cos(THE_Psi).*sin(THE_Phi).*sin(THE_Theta)).*(THE_Psi_D.*THE_Theta_D.*sin(THE_Psi)-THE_Phi_D.*THE_Psi_D.*cos(THE_Psi).*cos(THE_Theta)+THE_Phi_D.*THE_Theta_D.*sin(THE_Psi).*sin(THE_Theta))+cg_to_mot_H.*cos(THE_Theta).*sin(THE_Phi).*(THE_Psi_D.*THE_Theta_D.*sin(THE_Psi)-THE_Phi_D.*THE_Psi_D.*cos(THE_Psi).*cos(THE_Theta)+THE_Phi_D.*THE_Theta_D.*sin(THE_Psi).*sin(THE_Theta))-THE_Phi_D.*cg_to_mot_H.*cos(THE_Phi).*cos(THE_Theta).*(THE_Theta_D.*cos(THE_Psi)+THE_Phi_D.*cos(THE_Theta).*sin(THE_Psi))+THE_Theta_D.*cg_to_mot_H.*sin(THE_Phi).*sin(THE_Theta).*(THE_Theta_D.*cos(THE_Psi)+THE_Phi_D.*cos(THE_Theta).*sin(THE_Psi))))./2.0-(mprop.*((cg_to_mot_L.*(THE_Theta_D.*sin(THE_Psi)-THE_Phi_D.*cos(THE_Psi).*cos(THE_Theta))-cg_to_mot_H.*(THE_Psi_D-THE_Phi_D.*sin(THE_Theta))).*(-THE_Phi_D.*cos(THE_Psi).*sin(THE_Phi)-THE_Psi_D.*cos(THE_Phi).*sin(THE_Psi)+THE_Phi_D.*cos(THE_Phi).*sin(THE_Psi).*sin(THE_Theta)+THE_Psi_D.*cos(THE_Psi).*sin(THE_Phi).*sin(THE_Theta)+THE_Theta_D.*cos(THE_Theta).*sin(THE_Phi).*sin(THE_Psi))+(cg_to_mot_L.*(THE_Psi_D.*THE_Theta_D.*cos(THE_Psi)+THE_Phi_D.*THE_Psi_D.*cos(THE_Theta).*sin(THE_Psi)+THE_Phi_D.*THE_Theta_D.*cos(THE_Psi).*sin(THE_Theta))+THE_Phi_D.*THE_Theta_D.*cg_to_mot_H.*cos(THE_Theta)).*(cos(THE_Phi).*cos(THE_Psi)+sin(THE_Phi).*sin(THE_Psi).*sin(THE_Theta))+cg_to_mot_L.*(THE_Theta_D.*cos(THE_Psi)+THE_Phi_D.*cos(THE_Theta).*sin(THE_Psi)).*(-THE_Psi_D.*cos(THE_Phi).*cos(THE_Psi)+THE_Phi_D.*sin(THE_Phi).*sin(THE_Psi)-THE_Psi_D.*sin(THE_Phi).*sin(THE_Psi).*sin(THE_Theta)+THE_Phi_D.*cos(THE_Phi).*cos(THE_Psi).*sin(THE_Theta)+THE_Theta_D.*cos(THE_Psi).*cos(THE_Theta).*sin(THE_Phi))+cg_to_mot_L.*(cos(THE_Phi).*sin(THE_Psi)-cos(THE_Psi).*sin(THE_Phi).*sin(THE_Theta)).*(THE_Psi_D.*THE_Theta_D.*sin(THE_Psi)-THE_Phi_D.*THE_Psi_D.*cos(THE_Psi).*cos(THE_Theta)+THE_Phi_D.*THE_Theta_D.*sin(THE_Psi).*sin(THE_Theta))-cg_to_mot_H.*cos(THE_Theta).*sin(THE_Phi).*(THE_Psi_D.*THE_Theta_D.*sin(THE_Psi)-THE_Phi_D.*THE_Psi_D.*cos(THE_Psi).*cos(THE_Theta)+THE_Phi_D.*THE_Theta_D.*sin(THE_Psi).*sin(THE_Theta))+THE_Phi_D.*cg_to_mot_H.*cos(THE_Phi).*cos(THE_Theta).*(THE_Theta_D.*cos(THE_Psi)+THE_Phi_D.*cos(THE_Theta).*sin(THE_Psi))-THE_Theta_D.*cg_to_mot_H.*sin(THE_Phi).*sin(THE_Theta).*(THE_Theta_D.*cos(THE_Psi)+THE_Phi_D.*cos(THE_Theta).*sin(THE_Psi))))./2.0+mprop.*(((cg_to_mot_L.*(THE_Theta_D.*sin(THE_Psi)-THE_Phi_D.*cos(THE_Psi).*cos(THE_Theta))+cg_to_mot_H.*(THE_Psi_D-THE_Phi_D.*sin(THE_Theta))).*(-THE_Phi_D.*cos(THE_Psi).*sin(THE_Phi)-THE_Psi_D.*cos(THE_Phi).*sin(THE_Psi)+THE_Phi_D.*cos(THE_Phi).*sin(THE_Psi).*sin(THE_Theta)+THE_Psi_D.*cos(THE_Psi).*sin(THE_Phi).*sin(THE_Theta)+THE_Theta_D.*cos(THE_Theta).*sin(THE_Phi).*sin(THE_Psi)))./2.0+((cg_to_mot_L.*(THE_Psi_D.*THE_Theta_D.*cos(THE_Psi)+THE_Phi_D.*THE_Psi_D.*cos(THE_Theta).*sin(THE_Psi)+THE_Phi_D.*THE_Theta_D.*cos(THE_Psi).*sin(THE_Theta))-THE_Phi_D.*THE_Theta_D.*cg_to_mot_H.*cos(THE_Theta)).*(cos(THE_Phi).*cos(THE_Psi)+sin(THE_Phi).*sin(THE_Psi).*sin(THE_Theta)))./2.0+(cg_to_mot_L.*(THE_Theta_D.*cos(THE_Psi)+THE_Phi_D.*cos(THE_Theta).*sin(THE_Psi)).*(-THE_Psi_D.*cos(THE_Phi).*cos(THE_Psi)+THE_Phi_D.*sin(THE_Phi).*sin(THE_Psi)-THE_Psi_D.*sin(THE_Phi).*sin(THE_Psi).*sin(THE_Theta)+THE_Phi_D.*cos(THE_Phi).*cos(THE_Psi).*sin(THE_Theta)+THE_Theta_D.*cos(THE_Psi).*cos(THE_Theta).*sin(THE_Phi)))./2.0+(cg_to_mot_L.*(cos(THE_Phi).*sin(THE_Psi)-cos(THE_Psi).*sin(THE_Phi).*sin(THE_Theta)).*(THE_Psi_D.*THE_Theta_D.*sin(THE_Psi)-THE_Phi_D.*THE_Psi_D.*cos(THE_Psi).*cos(THE_Theta)+THE_Phi_D.*THE_Theta_D.*sin(THE_Psi).*sin(THE_Theta)))./2.0+(cg_to_mot_H.*cos(THE_Theta).*sin(THE_Phi).*(THE_Psi_D.*THE_Theta_D.*sin(THE_Psi)-THE_Phi_D.*THE_Psi_D.*cos(THE_Psi).*cos(THE_Theta)+THE_Phi_D.*THE_Theta_D.*sin(THE_Psi).*sin(THE_Theta)))./2.0-(THE_Phi_D.*cg_to_mot_H.*cos(THE_Phi).*cos(THE_Theta).*(THE_Theta_D.*cos(THE_Psi)+THE_Phi_D.*cos(THE_Theta).*sin(THE_Psi)))./2.0+(THE_Theta_D.*cg_to_mot_H.*sin(THE_Phi).*sin(THE_Theta).*(THE_Theta_D.*cos(THE_Psi)+THE_Phi_D.*cos(THE_Theta).*sin(THE_Psi)))./2.0)-mprop.*(((cg_to_mot_L.*(THE_Theta_D.*sin(THE_Psi)-THE_Phi_D.*cos(THE_Psi).*cos(THE_Theta))-cg_to_mot_H.*(THE_Psi_D-THE_Phi_D.*sin(THE_Theta))).*(-THE_Phi_D.*cos(THE_Psi).*sin(THE_Phi)-THE_Psi_D.*cos(THE_Phi).*sin(THE_Psi)+THE_Phi_D.*cos(THE_Phi).*sin(THE_Psi).*sin(THE_Theta)+THE_Psi_D.*cos(THE_Psi).*sin(THE_Phi).*sin(THE_Theta)+THE_Theta_D.*cos(THE_Theta).*sin(THE_Phi).*sin(THE_Psi)))./2.0+((cg_to_mot_L.*(THE_Psi_D.*THE_Theta_D.*cos(THE_Psi)+THE_Phi_D.*THE_Psi_D.*cos(THE_Theta).*sin(THE_Psi)+THE_Phi_D.*THE_Theta_D.*cos(THE_Psi).*sin(THE_Theta))+THE_Phi_D.*THE_Theta_D.*cg_to_mot_H.*cos(THE_Theta)).*(cos(THE_Phi).*cos(THE_Psi)+sin(THE_Phi).*sin(THE_Psi).*sin(THE_Theta)))./2.0+(cg_to_mot_L.*(THE_Theta_D.*cos(THE_Psi)+THE_Phi_D.*cos(THE_Theta).*sin(THE_Psi)).*(-THE_Psi_D.*cos(THE_Phi).*cos(THE_Psi)+THE_Phi_D.*sin(THE_Phi).*sin(THE_Psi)-THE_Psi_D.*sin(THE_Phi).*sin(THE_Psi).*sin(THE_Theta)+THE_Phi_D.*cos(THE_Phi).*cos(THE_Psi).*sin(THE_Theta)+THE_Theta_D.*cos(THE_Psi).*cos(THE_Theta).*sin(THE_Phi)))./2.0+(cg_to_mot_L.*(cos(THE_Phi).*sin(THE_Psi)-cos(THE_Psi).*sin(THE_Phi).*sin(THE_Theta)).*(THE_Psi_D.*THE_Theta_D.*sin(THE_Psi)-THE_Phi_D.*THE_Psi_D.*cos(THE_Psi).*cos(THE_Theta)+THE_Phi_D.*THE_Theta_D.*sin(THE_Psi).*sin(THE_Theta)))./2.0-(cg_to_mot_H.*cos(THE_Theta).*sin(THE_Phi).*(THE_Psi_D.*THE_Theta_D.*sin(THE_Psi)-THE_Phi_D.*THE_Psi_D.*cos(THE_Psi).*cos(THE_Theta)+THE_Phi_D.*THE_Theta_D.*sin(THE_Psi).*sin(THE_Theta)))./2.0+(THE_Phi_D.*cg_to_mot_H.*cos(THE_Phi).*cos(THE_Theta).*(THE_Theta_D.*cos(THE_Psi)+THE_Phi_D.*cos(THE_Theta).*sin(THE_Psi)))./2.0-(THE_Theta_D.*cg_to_mot_H.*sin(THE_Phi).*sin(THE_Theta).*(THE_Theta_D.*cos(THE_Psi)+THE_Phi_D.*cos(THE_Theta).*sin(THE_Psi)))./2.0)+(m_pend.*((Tv_Z_pend+(Lz_pend.*cos(THE_Psi_pend).*cos(THE_Theta_pend))./2.0).*(-THE_Phi_D.^2.*cos(THE_Phi).*sin(THE_Psi)-THE_Psi_D.^2.*cos(THE_Phi).*sin(THE_Psi)+THE_Phi_D.^2.*cos(THE_Psi).*sin(THE_Phi).*sin(THE_Theta)+THE_Psi_D.^2.*cos(THE_Psi).*sin(THE_Phi).*sin(THE_Theta)+THE_Theta_D.^2.*cos(THE_Psi).*sin(THE_Phi).*sin(THE_Theta)-THE_Phi_D.*THE_Psi_D.*cos(THE_Psi).*sin(THE_Phi).*2.0-THE_Phi_D.*THE_Theta_D.*cos(THE_Phi).*cos(THE_Psi).*cos(THE_Theta).*2.0+THE_Phi_D.*THE_Psi_D.*cos(THE_Phi).*sin(THE_Psi).*sin(THE_Theta).*2.0+THE_Psi_D.*THE_Theta_D.*cos(THE_Theta).*sin(THE_Phi).*sin(THE_Psi).*2.0)-(cos(THE_Phi).*sin(THE_Psi)-cos(THE_Psi).*sin(THE_Phi).*sin(THE_Theta)).*((Lz_pend.*THE_Psi_pend_D.^2.*cos(THE_Psi_pend).*cos(THE_Theta_pend))./2.0+(Lz_pend.*THE_Theta_pend_D.^2.*cos(THE_Psi_pend).*cos(THE_Theta_pend))./2.0-Lz_pend.*THE_Psi_pend_D.*THE_Theta_pend_D.*sin(THE_Psi_pend).*sin(THE_Theta_pend))+((Lz_pend.*THE_Psi_pend_D.*cos(THE_Theta_pend).*sin(THE_Psi_pend))./2.0+(Lz_pend.*THE_Theta_pend_D.*cos(THE_Psi_pend).*sin(THE_Theta_pend))./2.0).*(-THE_Psi_D.*cos(THE_Phi).*cos(THE_Psi)+THE_Phi_D.*sin(THE_Phi).*sin(THE_Psi)-THE_Psi_D.*sin(THE_Phi).*sin(THE_Psi).*sin(THE_Theta)+THE_Phi_D.*cos(THE_Phi).*cos(THE_Psi).*sin(THE_Theta)+THE_Theta_D.*cos(THE_Psi).*cos(THE_Theta).*sin(THE_Phi)).*2.0-Lz_pend.*(-THE_Psi_pend_D.*cos(THE_Phi_pend).*cos(THE_Psi_pend)+THE_Phi_pend_D.*sin(THE_Phi_pend).*sin(THE_Psi_pend)-THE_Psi_pend_D.*sin(THE_Phi_pend).*sin(THE_Psi_pend).*sin(THE_Theta_pend)+THE_Phi_pend_D.*cos(THE_Phi_pend).*cos(THE_Psi_pend).*sin(THE_Theta_pend)+THE_Theta_pend_D.*cos(THE_Psi_pend).*cos(THE_Theta_pend).*sin(THE_Phi_pend)).*(-THE_Phi_D.*cos(THE_Psi).*sin(THE_Phi)-THE_Psi_D.*cos(THE_Phi).*sin(THE_Psi)+THE_Phi_D.*cos(THE_Phi).*sin(THE_Psi).*sin(THE_Theta)+THE_Psi_D.*cos(THE_Psi).*sin(THE_Phi).*sin(THE_Theta)+THE_Theta_D.*cos(THE_Theta).*sin(THE_Phi).*sin(THE_Psi))+(Lz_pend.*(cos(THE_Phi).*cos(THE_Psi)+sin(THE_Phi).*sin(THE_Psi).*sin(THE_Theta)).*(-THE_Phi_pend_D.^2.*cos(THE_Phi_pend).*sin(THE_Psi_pend)-THE_Psi_pend_D.^2.*cos(THE_Phi_pend).*sin(THE_Psi_pend)+THE_Phi_pend_D.^2.*cos(THE_Psi_pend).*sin(THE_Phi_pend).*sin(THE_Theta_pend)+THE_Psi_pend_D.^2.*cos(THE_Psi_pend).*sin(THE_Phi_pend).*sin(THE_Theta_pend)+THE_Theta_pend_D.^2.*cos(THE_Psi_pend).*sin(THE_Phi_pend).*sin(THE_Theta_pend)-THE_Phi_pend_D.*THE_Psi_pend_D.*cos(THE_Psi_pend).*sin(THE_Phi_pend).*2.0-THE_Phi_pend_D.*THE_Theta_pend_D.*cos(THE_Phi_pend).*cos(THE_Psi_pend).*cos(THE_Theta_pend).*2.0+THE_Phi_pend_D.*THE_Psi_pend_D.*cos(THE_Phi_pend).*sin(THE_Psi_pend).*sin(THE_Theta_pend).*2.0+THE_Psi_pend_D.*THE_Theta_pend_D.*cos(THE_Theta_pend).*sin(THE_Phi_pend).*sin(THE_Psi_pend).*2.0))./2.0-(Lz_pend.*(cos(THE_Phi_pend).*sin(THE_Psi_pend)-cos(THE_Psi_pend).*sin(THE_Phi_pend).*sin(THE_Theta_pend)).*(THE_Phi_D.^2.*cos(THE_Phi).*cos(THE_Psi)+THE_Psi_D.^2.*cos(THE_Phi).*cos(THE_Psi)+THE_Phi_D.^2.*sin(THE_Phi).*sin(THE_Psi).*sin(THE_Theta)+THE_Psi_D.^2.*sin(THE_Phi).*sin(THE_Psi).*sin(THE_Theta)+THE_Theta_D.^2.*sin(THE_Phi).*sin(THE_Psi).*sin(THE_Theta)-THE_Phi_D.*THE_Psi_D.*sin(THE_Phi).*sin(THE_Psi).*2.0-THE_Phi_D.*THE_Psi_D.*cos(THE_Phi).*cos(THE_Psi).*sin(THE_Theta).*2.0-THE_Phi_D.*THE_Theta_D.*cos(THE_Phi).*cos(THE_Theta).*sin(THE_Psi).*2.0-THE_Psi_D.*THE_Theta_D.*cos(THE_Psi).*cos(THE_Theta).*sin(THE_Phi).*2.0))./2.0+(Lz_pend.*cos(THE_Theta).*sin(THE_Phi).*(THE_Phi_pend_D.^2.*sin(THE_Phi_pend).*sin(THE_Psi_pend)+THE_Psi_pend_D.^2.*sin(THE_Phi_pend).*sin(THE_Psi_pend)+THE_Phi_pend_D.^2.*cos(THE_Phi_pend).*cos(THE_Psi_pend).*sin(THE_Theta_pend)+THE_Psi_pend_D.^2.*cos(THE_Phi_pend).*cos(THE_Psi_pend).*sin(THE_Theta_pend)+THE_Theta_pend_D.^2.*cos(THE_Phi_pend).*cos(THE_Psi_pend).*sin(THE_Theta_pend)-THE_Phi_pend_D.*THE_Psi_pend_D.*cos(THE_Phi_pend).*cos(THE_Psi_pend).*2.0+THE_Phi_pend_D.*THE_Theta_pend_D.*cos(THE_Psi_pend).*cos(THE_Theta_pend).*sin(THE_Phi_pend).*2.0+THE_Psi_pend_D.*THE_Theta_pend_D.*cos(THE_Phi_pend).*cos(THE_Theta_pend).*sin(THE_Psi_pend).*2.0-THE_Phi_pend_D.*THE_Psi_pend_D.*sin(THE_Phi_pend).*sin(THE_Psi_pend).*sin(THE_Theta_pend).*2.0))./2.0-Lz_pend.*THE_Phi_D.*cos(THE_Phi).*cos(THE_Theta).*(THE_Phi_pend_D.*cos(THE_Phi_pend).*sin(THE_Psi_pend)+THE_Psi_pend_D.*cos(THE_Psi_pend).*sin(THE_Phi_pend)+THE_Theta_pend_D.*cos(THE_Phi_pend).*cos(THE_Psi_pend).*cos(THE_Theta_pend)-THE_Phi_pend_D.*cos(THE_Psi_pend).*sin(THE_Phi_pend).*sin(THE_Theta_pend)-THE_Psi_pend_D.*cos(THE_Phi_pend).*sin(THE_Psi_pend).*sin(THE_Theta_pend))+Lz_pend.*THE_Theta_D.*sin(THE_Phi).*sin(THE_Theta).*(THE_Phi_pend_D.*cos(THE_Phi_pend).*sin(THE_Psi_pend)+THE_Psi_pend_D.*cos(THE_Psi_pend).*sin(THE_Phi_pend)+THE_Theta_pend_D.*cos(THE_Phi_pend).*cos(THE_Psi_pend).*cos(THE_Theta_pend)-THE_Phi_pend_D.*cos(THE_Psi_pend).*sin(THE_Phi_pend).*sin(THE_Theta_pend)-THE_Psi_pend_D.*cos(THE_Phi_pend).*sin(THE_Psi_pend).*sin(THE_Theta_pend))+(Lz_pend.*THE_Phi_D.^2.*cos(THE_Theta).*sin(THE_Phi).*(sin(THE_Phi_pend).*sin(THE_Psi_pend)+cos(THE_Phi_pend).*cos(THE_Psi_pend).*sin(THE_Theta_pend)))./2.0+(Lz_pend.*THE_Theta_D.^2.*cos(THE_Theta).*sin(THE_Phi).*(sin(THE_Phi_pend).*sin(THE_Psi_pend)+cos(THE_Phi_pend).*cos(THE_Psi_pend).*sin(THE_Theta_pend)))./2.0+Lz_pend.*THE_Phi_D.*THE_Theta_D.*cos(THE_Phi).*sin(THE_Theta).*(sin(THE_Phi_pend).*sin(THE_Psi_pend)+cos(THE_Phi_pend).*cos(THE_Psi_pend).*sin(THE_Theta_pend))))./2.0+m_pend.*(((Tv_Z_pend+(Lz_pend.*cos(THE_Psi_pend).*cos(THE_Theta_pend))./2.0).*(-THE_Phi_D.^2.*cos(THE_Phi).*sin(THE_Psi)-THE_Psi_D.^2.*cos(THE_Phi).*sin(THE_Psi)+THE_Phi_D.^2.*cos(THE_Psi).*sin(THE_Phi).*sin(THE_Theta)+THE_Psi_D.^2.*cos(THE_Psi).*sin(THE_Phi).*sin(THE_Theta)+THE_Theta_D.^2.*cos(THE_Psi).*sin(THE_Phi).*sin(THE_Theta)-THE_Phi_D.*THE_Psi_D.*cos(THE_Psi).*sin(THE_Phi).*2.0-THE_Phi_D.*THE_Theta_D.*cos(THE_Phi).*cos(THE_Psi).*cos(THE_Theta).*2.0+THE_Phi_D.*THE_Psi_D.*cos(THE_Phi).*sin(THE_Psi).*sin(THE_Theta).*2.0+THE_Psi_D.*THE_Theta_D.*cos(THE_Theta).*sin(THE_Phi).*sin(THE_Psi).*2.0))./2.0-((cos(THE_Phi).*sin(THE_Psi)-cos(THE_Psi).*sin(THE_Phi).*sin(THE_Theta)).*((Lz_pend.*THE_Psi_pend_D.^2.*cos(THE_Psi_pend).*cos(THE_Theta_pend))./2.0+(Lz_pend.*THE_Theta_pend_D.^2.*cos(THE_Psi_pend).*cos(THE_Theta_pend))./2.0-Lz_pend.*THE_Psi_pend_D.*THE_Theta_pend_D.*sin(THE_Psi_pend).*sin(THE_Theta_pend)))./2.0+((Lz_pend.*THE_Psi_pend_D.*cos(THE_Theta_pend).*sin(THE_Psi_pend))./2.0+(Lz_pend.*THE_Theta_pend_D.*cos(THE_Psi_pend).*sin(THE_Theta_pend))./2.0).*(-THE_Psi_D.*cos(THE_Phi).*cos(THE_Psi)+THE_Phi_D.*sin(THE_Phi).*sin(THE_Psi)-THE_Psi_D.*sin(THE_Phi).*sin(THE_Psi).*sin(THE_Theta)+THE_Phi_D.*cos(THE_Phi).*cos(THE_Psi).*sin(THE_Theta)+THE_Theta_D.*cos(THE_Psi).*cos(THE_Theta).*sin(THE_Phi))-(Lz_pend.*(-THE_Psi_pend_D.*cos(THE_Phi_pend).*cos(THE_Psi_pend)+THE_Phi_pend_D.*sin(THE_Phi_pend).*sin(THE_Psi_pend)-THE_Psi_pend_D.*sin(THE_Phi_pend).*sin(THE_Psi_pend).*sin(THE_Theta_pend)+THE_Phi_pend_D.*cos(THE_Phi_pend).*cos(THE_Psi_pend).*sin(THE_Theta_pend)+THE_Theta_pend_D.*cos(THE_Psi_pend).*cos(THE_Theta_pend).*sin(THE_Phi_pend)).*(-THE_Phi_D.*cos(THE_Psi).*sin(THE_Phi)-THE_Psi_D.*cos(THE_Phi).*sin(THE_Psi)+THE_Phi_D.*cos(THE_Phi).*sin(THE_Psi).*sin(THE_Theta)+THE_Psi_D.*cos(THE_Psi).*sin(THE_Phi).*sin(THE_Theta)+THE_Theta_D.*cos(THE_Theta).*sin(THE_Phi).*sin(THE_Psi)))./2.0+(Lz_pend.*(cos(THE_Phi).*cos(THE_Psi)+sin(THE_Phi).*sin(THE_Psi).*sin(THE_Theta)).*(-THE_Phi_pend_D.^2.*cos(THE_Phi_pend).*sin(THE_Psi_pend)-THE_Psi_pend_D.^2.*cos(THE_Phi_pend).*sin(THE_Psi_pend)+THE_Phi_pend_D.^2.*cos(THE_Psi_pend).*sin(THE_Phi_pend).*sin(THE_Theta_pend)+THE_Psi_pend_D.^2.*cos(THE_Psi_pend).*sin(THE_Phi_pend).*sin(THE_Theta_pend)+THE_Theta_pend_D.^2.*cos(THE_Psi_pend).*sin(THE_Phi_pend).*sin(THE_Theta_pend)-THE_Phi_pend_D.*THE_Psi_pend_D.*cos(THE_Psi_pend).*sin(THE_Phi_pend).*2.0-THE_Phi_pend_D.*THE_Theta_pend_D.*cos(THE_Phi_pend).*cos(THE_Psi_pend).*cos(THE_Theta_pend).*2.0+THE_Phi_pend_D.*THE_Psi_pend_D.*cos(THE_Phi_pend).*sin(THE_Psi_pend).*sin(THE_Theta_pend).*2.0+THE_Psi_pend_D.*THE_Theta_pend_D.*cos(THE_Theta_pend).*sin(THE_Phi_pend).*sin(THE_Psi_pend).*2.0))./4.0-(Lz_pend.*(cos(THE_Phi_pend).*sin(THE_Psi_pend)-cos(THE_Psi_pend).*sin(THE_Phi_pend).*sin(THE_Theta_pend)).*(THE_Phi_D.^2.*cos(THE_Phi).*cos(THE_Psi)+THE_Psi_D.^2.*cos(THE_Phi).*cos(THE_Psi)+THE_Phi_D.^2.*sin(THE_Phi).*sin(THE_Psi).*sin(THE_Theta)+THE_Psi_D.^2.*sin(THE_Phi).*sin(THE_Psi).*sin(THE_Theta)+THE_Theta_D.^2.*sin(THE_Phi).*sin(THE_Psi).*sin(THE_Theta)-THE_Phi_D.*THE_Psi_D.*sin(THE_Phi).*sin(THE_Psi).*2.0-THE_Phi_D.*THE_Psi_D.*cos(THE_Phi).*cos(THE_Psi).*sin(THE_Theta).*2.0-THE_Phi_D.*THE_Theta_D.*cos(THE_Phi).*cos(THE_Theta).*sin(THE_Psi).*2.0-THE_Psi_D.*THE_Theta_D.*cos(THE_Psi).*cos(THE_Theta).*sin(THE_Phi).*2.0))./4.0+(Lz_pend.*cos(THE_Theta).*sin(THE_Phi).*(THE_Phi_pend_D.^2.*sin(THE_Phi_pend).*sin(THE_Psi_pend)+THE_Psi_pend_D.^2.*sin(THE_Phi_pend).*sin(THE_Psi_pend)+THE_Phi_pend_D.^2.*cos(THE_Phi_pend).*cos(THE_Psi_pend).*sin(THE_Theta_pend)+THE_Psi_pend_D.^2.*cos(THE_Phi_pend).*cos(THE_Psi_pend).*sin(THE_Theta_pend)+THE_Theta_pend_D.^2.*cos(THE_Phi_pend).*cos(THE_Psi_pend).*sin(THE_Theta_pend)-THE_Phi_pend_D.*THE_Psi_pend_D.*cos(THE_Phi_pend).*cos(THE_Psi_pend).*2.0+THE_Phi_pend_D.*THE_Theta_pend_D.*cos(THE_Psi_pend).*cos(THE_Theta_pend).*sin(THE_Phi_pend).*2.0+THE_Psi_pend_D.*THE_Theta_pend_D.*cos(THE_Phi_pend).*cos(THE_Theta_pend).*sin(THE_Psi_pend).*2.0-THE_Phi_pend_D.*THE_Psi_pend_D.*sin(THE_Phi_pend).*sin(THE_Psi_pend).*sin(THE_Theta_pend).*2.0))./4.0-(Lz_pend.*THE_Phi_D.*cos(THE_Phi).*cos(THE_Theta).*(THE_Phi_pend_D.*cos(THE_Phi_pend).*sin(THE_Psi_pend)+THE_Psi_pend_D.*cos(THE_Psi_pend).*sin(THE_Phi_pend)+THE_Theta_pend_D.*cos(THE_Phi_pend).*cos(THE_Psi_pend).*cos(THE_Theta_pend)-THE_Phi_pend_D.*cos(THE_Psi_pend).*sin(THE_Phi_pend).*sin(THE_Theta_pend)-THE_Psi_pend_D.*cos(THE_Phi_pend).*sin(THE_Psi_pend).*sin(THE_Theta_pend)))./2.0+(Lz_pend.*THE_Theta_D.*sin(THE_Phi).*sin(THE_Theta).*(THE_Phi_pend_D.*cos(THE_Phi_pend).*sin(THE_Psi_pend)+THE_Psi_pend_D.*cos(THE_Psi_pend).*sin(THE_Phi_pend)+THE_Theta_pend_D.*cos(THE_Phi_pend).*cos(THE_Psi_pend).*cos(THE_Theta_pend)-THE_Phi_pend_D.*cos(THE_Psi_pend).*sin(THE_Phi_pend).*sin(THE_Theta_pend)-THE_Psi_pend_D.*cos(THE_Phi_pend).*sin(THE_Psi_pend).*sin(THE_Theta_pend)))./2.0+(Lz_pend.*THE_Phi_D.^2.*cos(THE_Theta).*sin(THE_Phi).*(sin(THE_Phi_pend).*sin(THE_Psi_pend)+cos(THE_Phi_pend).*cos(THE_Psi_pend).*sin(THE_Theta_pend)))./4.0+(Lz_pend.*THE_Theta_D.^2.*cos(THE_Theta).*sin(THE_Phi).*(sin(THE_Phi_pend).*sin(THE_Psi_pend)+cos(THE_Phi_pend).*cos(THE_Psi_pend).*sin(THE_Theta_pend)))./4.0+(Lz_pend.*THE_Phi_D.*THE_Theta_D.*cos(THE_Phi).*sin(THE_Theta).*(sin(THE_Phi_pend).*sin(THE_Psi_pend)+cos(THE_Phi_pend).*cos(THE_Psi_pend).*sin(THE_Theta_pend)))./2.0)-Tbz_1.*(cos(THE_Phi).*sin(THE_Psi)-cos(THE_Psi).*sin(THE_Phi).*sin(THE_Theta))-Tbz_2.*(cos(THE_Phi).*sin(THE_Psi)-cos(THE_Psi).*sin(THE_Phi).*sin(THE_Theta))-Tbz_3.*(cos(THE_Phi).*sin(THE_Psi)-cos(THE_Psi).*sin(THE_Phi).*sin(THE_Theta))-Tbz_4.*(cos(THE_Phi).*sin(THE_Psi)-cos(THE_Psi).*sin(THE_Phi).*sin(THE_Theta))+(mprop.*(cos(THE_Theta).*sin(THE_Phi).*(cg_to_mot_H.*(THE_Psi_D.*THE_Theta_D.*sin(THE_Psi)-THE_Phi_D.*THE_Psi_D.*cos(THE_Psi).*cos(THE_Theta)+THE_Phi_D.*THE_Theta_D.*sin(THE_Psi).*sin(THE_Theta))+cg_to_mot_L.*(THE_Psi_D.*THE_Theta_D.*cos(THE_Psi)+THE_Phi_D.*THE_Psi_D.*cos(THE_Theta).*sin(THE_Psi)+THE_Phi_D.*THE_Theta_D.*cos(THE_Psi).*sin(THE_Theta)))+cg_to_mot_L.*(THE_Psi_D-THE_Phi_D.*sin(THE_Theta)).*(-THE_Psi_D.*cos(THE_Phi).*cos(THE_Psi)+THE_Phi_D.*sin(THE_Phi).*sin(THE_Psi)-THE_Psi_D.*sin(THE_Phi).*sin(THE_Psi).*sin(THE_Theta)+THE_Phi_D.*cos(THE_Phi).*cos(THE_Psi).*sin(THE_Theta)+THE_Theta_D.*cos(THE_Psi).*cos(THE_Theta).*sin(THE_Phi))+cg_to_mot_H.*(THE_Psi_D-THE_Phi_D.*sin(THE_Theta)).*(-THE_Phi_D.*cos(THE_Psi).*sin(THE_Phi)-THE_Psi_D.*cos(THE_Phi).*sin(THE_Psi)+THE_Phi_D.*cos(THE_Phi).*sin(THE_Psi).*sin(THE_Theta)+THE_Psi_D.*cos(THE_Psi).*sin(THE_Phi).*sin(THE_Theta)+THE_Theta_D.*cos(THE_Theta).*sin(THE_Phi).*sin(THE_Psi))-THE_Phi_D.*cos(THE_Phi).*cos(THE_Theta).*(cg_to_mot_H.*(THE_Theta_D.*cos(THE_Psi)+THE_Phi_D.*cos(THE_Theta).*sin(THE_Psi))-cg_to_mot_L.*(THE_Theta_D.*sin(THE_Psi)-THE_Phi_D.*cos(THE_Psi).*cos(THE_Theta)))+THE_Theta_D.*sin(THE_Phi).*sin(THE_Theta).*(cg_to_mot_H.*(THE_Theta_D.*cos(THE_Psi)+THE_Phi_D.*cos(THE_Theta).*sin(THE_Psi))-cg_to_mot_L.*(THE_Theta_D.*sin(THE_Psi)-THE_Phi_D.*cos(THE_Psi).*cos(THE_Theta)))-THE_Phi_D.*THE_Theta_D.*cg_to_mot_H.*cos(THE_Theta).*(cos(THE_Phi).*cos(THE_Psi)+sin(THE_Phi).*sin(THE_Psi).*sin(THE_Theta))+THE_Phi_D.*THE_Theta_D.*cg_to_mot_L.*cos(THE_Theta).*(cos(THE_Phi).*sin(THE_Psi)-cos(THE_Psi).*sin(THE_Phi).*sin(THE_Theta))))./2.0-(mprop.*(-cos(THE_Theta).*sin(THE_Phi).*(cg_to_mot_H.*(THE_Psi_D.*THE_Theta_D.*sin(THE_Psi)-THE_Phi_D.*THE_Psi_D.*cos(THE_Psi).*cos(THE_Theta)+THE_Phi_D.*THE_Theta_D.*sin(THE_Psi).*sin(THE_Theta))-cg_to_mot_L.*(THE_Psi_D.*THE_Theta_D.*cos(THE_Psi)+THE_Phi_D.*THE_Psi_D.*cos(THE_Theta).*sin(THE_Psi)+THE_Phi_D.*THE_Theta_D.*cos(THE_Psi).*sin(THE_Theta)))+cg_to_mot_L.*(THE_Psi_D-THE_Phi_D.*sin(THE_Theta)).*(-THE_Psi_D.*cos(THE_Phi).*cos(THE_Psi)+THE_Phi_D.*sin(THE_Phi).*sin(THE_Psi)-THE_Psi_D.*sin(THE_Phi).*sin(THE_Psi).*sin(THE_Theta)+THE_Phi_D.*cos(THE_Phi).*cos(THE_Psi).*sin(THE_Theta)+THE_Theta_D.*cos(THE_Psi).*cos(THE_Theta).*sin(THE_Phi))-cg_to_mot_H.*(THE_Psi_D-THE_Phi_D.*sin(THE_Theta)).*(-THE_Phi_D.*cos(THE_Psi).*sin(THE_Phi)-THE_Psi_D.*cos(THE_Phi).*sin(THE_Psi)+THE_Phi_D.*cos(THE_Phi).*sin(THE_Psi).*sin(THE_Theta)+THE_Psi_D.*cos(THE_Psi).*sin(THE_Phi).*sin(THE_Theta)+THE_Theta_D.*cos(THE_Theta).*sin(THE_Phi).*sin(THE_Psi))+THE_Phi_D.*cos(THE_Phi).*cos(THE_Theta).*(cg_to_mot_H.*(THE_Theta_D.*cos(THE_Psi)+THE_Phi_D.*cos(THE_Theta).*sin(THE_Psi))+cg_to_mot_L.*(THE_Theta_D.*sin(THE_Psi)-THE_Phi_D.*cos(THE_Psi).*cos(THE_Theta)))-THE_Theta_D.*sin(THE_Phi).*sin(THE_Theta).*(cg_to_mot_H.*(THE_Theta_D.*cos(THE_Psi)+THE_Phi_D.*cos(THE_Theta).*sin(THE_Psi))+cg_to_mot_L.*(THE_Theta_D.*sin(THE_Psi)-THE_Phi_D.*cos(THE_Psi).*cos(THE_Theta)))+THE_Phi_D.*THE_Theta_D.*cg_to_mot_H.*cos(THE_Theta).*(cos(THE_Phi).*cos(THE_Psi)+sin(THE_Phi).*sin(THE_Psi).*sin(THE_Theta))+THE_Phi_D.*THE_Theta_D.*cg_to_mot_L.*cos(THE_Theta).*(cos(THE_Phi).*sin(THE_Psi)-cos(THE_Psi).*sin(THE_Phi).*sin(THE_Theta))))./2.0-mprop.*(cos(THE_Theta).*sin(THE_Phi).*(cg_to_mot_H.*(THE_Psi_D.*THE_Theta_D.*sin(THE_Psi)-THE_Phi_D.*THE_Psi_D.*cos(THE_Psi).*cos(THE_Theta)+THE_Phi_D.*THE_Theta_D.*sin(THE_Psi).*sin(THE_Theta))-cg_to_mot_L.*(THE_Psi_D.*THE_Theta_D.*cos(THE_Psi)+THE_Phi_D.*THE_Psi_D.*cos(THE_Theta).*sin(THE_Psi)+THE_Phi_D.*THE_Theta_D.*cos(THE_Psi).*sin(THE_Theta))).*(-1.0./2.0)+(cg_to_mot_L.*(THE_Psi_D-THE_Phi_D.*sin(THE_Theta)).*(-THE_Psi_D.*cos(THE_Phi).*cos(THE_Psi)+THE_Phi_D.*sin(THE_Phi).*sin(THE_Psi)-THE_Psi_D.*sin(THE_Phi).*sin(THE_Psi).*sin(THE_Theta)+THE_Phi_D.*cos(THE_Phi).*cos(THE_Psi).*sin(THE_Theta)+THE_Theta_D.*cos(THE_Psi).*cos(THE_Theta).*sin(THE_Phi)))./2.0-(cg_to_mot_H.*(THE_Psi_D-THE_Phi_D.*sin(THE_Theta)).*(-THE_Phi_D.*cos(THE_Psi).*sin(THE_Phi)-THE_Psi_D.*cos(THE_Phi).*sin(THE_Psi)+THE_Phi_D.*cos(THE_Phi).*sin(THE_Psi).*sin(THE_Theta)+THE_Psi_D.*cos(THE_Psi).*sin(THE_Phi).*sin(THE_Theta)+THE_Theta_D.*cos(THE_Theta).*sin(THE_Phi).*sin(THE_Psi)))./2.0+(THE_Phi_D.*cos(THE_Phi).*cos(THE_Theta).*(cg_to_mot_H.*(THE_Theta_D.*cos(THE_Psi)+THE_Phi_D.*cos(THE_Theta).*sin(THE_Psi))+cg_to_mot_L.*(THE_Theta_D.*sin(THE_Psi)-THE_Phi_D.*cos(THE_Psi).*cos(THE_Theta))))./2.0-(THE_Theta_D.*sin(THE_Phi).*sin(THE_Theta).*(cg_to_mot_H.*(THE_Theta_D.*cos(THE_Psi)+THE_Phi_D.*cos(THE_Theta).*sin(THE_Psi))+cg_to_mot_L.*(THE_Theta_D.*sin(THE_Psi)-THE_Phi_D.*cos(THE_Psi).*cos(THE_Theta))))./2.0+(THE_Phi_D.*THE_Theta_D.*cg_to_mot_H.*cos(THE_Theta).*(cos(THE_Phi).*cos(THE_Psi)+sin(THE_Phi).*sin(THE_Psi).*sin(THE_Theta)))./2.0+(THE_Phi_D.*THE_Theta_D.*cg_to_mot_L.*cos(THE_Theta).*(cos(THE_Phi).*sin(THE_Psi)-cos(THE_Psi).*sin(THE_Phi).*sin(THE_Theta)))./2.0)+mprop.*((cos(THE_Theta).*sin(THE_Phi).*(cg_to_mot_H.*(THE_Psi_D.*THE_Theta_D.*sin(THE_Psi)-THE_Phi_D.*THE_Psi_D.*cos(THE_Psi).*cos(THE_Theta)+THE_Phi_D.*THE_Theta_D.*sin(THE_Psi).*sin(THE_Theta))+cg_to_mot_L.*(THE_Psi_D.*THE_Theta_D.*cos(THE_Psi)+THE_Phi_D.*THE_Psi_D.*cos(THE_Theta).*sin(THE_Psi)+THE_Phi_D.*THE_Theta_D.*cos(THE_Psi).*sin(THE_Theta))))./2.0+(cg_to_mot_L.*(THE_Psi_D-THE_Phi_D.*sin(THE_Theta)).*(-THE_Psi_D.*cos(THE_Phi).*cos(THE_Psi)+THE_Phi_D.*sin(THE_Phi).*sin(THE_Psi)-THE_Psi_D.*sin(THE_Phi).*sin(THE_Psi).*sin(THE_Theta)+THE_Phi_D.*cos(THE_Phi).*cos(THE_Psi).*sin(THE_Theta)+THE_Theta_D.*cos(THE_Psi).*cos(THE_Theta).*sin(THE_Phi)))./2.0+(cg_to_mot_H.*(THE_Psi_D-THE_Phi_D.*sin(THE_Theta)).*(-THE_Phi_D.*cos(THE_Psi).*sin(THE_Phi)-THE_Psi_D.*cos(THE_Phi).*sin(THE_Psi)+THE_Phi_D.*cos(THE_Phi).*sin(THE_Psi).*sin(THE_Theta)+THE_Psi_D.*cos(THE_Psi).*sin(THE_Phi).*sin(THE_Theta)+THE_Theta_D.*cos(THE_Theta).*sin(THE_Phi).*sin(THE_Psi)))./2.0-(THE_Phi_D.*cos(THE_Phi).*cos(THE_Theta).*(cg_to_mot_H.*(THE_Theta_D.*cos(THE_Psi)+THE_Phi_D.*cos(THE_Theta).*sin(THE_Psi))-cg_to_mot_L.*(THE_Theta_D.*sin(THE_Psi)-THE_Phi_D.*cos(THE_Psi).*cos(THE_Theta))))./2.0+(THE_Theta_D.*sin(THE_Phi).*sin(THE_Theta).*(cg_to_mot_H.*(THE_Theta_D.*cos(THE_Psi)+THE_Phi_D.*cos(THE_Theta).*sin(THE_Psi))-cg_to_mot_L.*(THE_Theta_D.*sin(THE_Psi)-THE_Phi_D.*cos(THE_Psi).*cos(THE_Theta))))./2.0-(THE_Phi_D.*THE_Theta_D.*cg_to_mot_H.*cos(THE_Theta).*(cos(THE_Phi).*cos(THE_Psi)+sin(THE_Phi).*sin(THE_Psi).*sin(THE_Theta)))./2.0+(THE_Phi_D.*THE_Theta_D.*cg_to_mot_L.*cos(THE_Theta).*(cos(THE_Phi).*sin(THE_Psi)-cos(THE_Psi).*sin(THE_Phi).*sin(THE_Theta)))./2.0);-g.*m-g.*m_pend-g.*mprop.*4.0-(mprop.*(-cos(THE_Theta).*sin(THE_Psi).*(cg_to_mot_L.*(THE_Psi_D.*THE_Theta_D.*cos(THE_Psi)+THE_Phi_D.*THE_Psi_D.*cos(THE_Theta).*sin(THE_Psi)+THE_Phi_D.*THE_Theta_D.*cos(THE_Psi).*sin(THE_Theta))-THE_Phi_D.*THE_Theta_D.*cg_to_mot_H.*cos(THE_Theta))+cg_to_mot_H.*sin(THE_Theta).*(THE_Psi_D.*THE_Theta_D.*sin(THE_Psi)-THE_Phi_D.*THE_Psi_D.*cos(THE_Psi).*cos(THE_Theta)+THE_Phi_D.*THE_Theta_D.*sin(THE_Psi).*sin(THE_Theta))-THE_Psi_D.*cos(THE_Psi).*cos(THE_Theta).*(cg_to_mot_L.*(THE_Theta_D.*sin(THE_Psi)-THE_Phi_D.*cos(THE_Psi).*cos(THE_Theta))+cg_to_mot_H.*(THE_Psi_D-THE_Phi_D.*sin(THE_Theta)))+THE_Theta_D.*sin(THE_Psi).*sin(THE_Theta).*(cg_to_mot_L.*(THE_Theta_D.*sin(THE_Psi)-THE_Phi_D.*cos(THE_Psi).*cos(THE_Theta))+cg_to_mot_H.*(THE_Psi_D-THE_Phi_D.*sin(THE_Theta)))+cg_to_mot_L.*cos(THE_Psi).*cos(THE_Theta).*(THE_Psi_D.*THE_Theta_D.*sin(THE_Psi)-THE_Phi_D.*THE_Psi_D.*cos(THE_Psi).*cos(THE_Theta)+THE_Phi_D.*THE_Theta_D.*sin(THE_Psi).*sin(THE_Theta))-THE_Theta_D.*cg_to_mot_H.*cos(THE_Theta).*(THE_Theta_D.*cos(THE_Psi)+THE_Phi_D.*cos(THE_Theta).*sin(THE_Psi))+THE_Psi_D.*cg_to_mot_L.*cos(THE_Theta).*sin(THE_Psi).*(THE_Theta_D.*cos(THE_Psi)+THE_Phi_D.*cos(THE_Theta).*sin(THE_Psi))+THE_Theta_D.*cg_to_mot_L.*cos(THE_Psi).*sin(THE_Theta).*(THE_Theta_D.*cos(THE_Psi)+THE_Phi_D.*cos(THE_Theta).*sin(THE_Psi))))./2.0+(mprop.*(-cos(THE_Theta).*sin(THE_Psi).*(cg_to_mot_L.*(THE_Psi_D.*THE_Theta_D.*cos(THE_Psi)+THE_Phi_D.*THE_Psi_D.*cos(THE_Theta).*sin(THE_Psi)+THE_Phi_D.*THE_Theta_D.*cos(THE_Psi).*sin(THE_Theta))+THE_Phi_D.*THE_Theta_D.*cg_to_mot_H.*cos(THE_Theta))-cg_to_mot_H.*sin(THE_Theta).*(THE_Psi_D.*THE_Theta_D.*sin(THE_Psi)-THE_Phi_D.*THE_Psi_D.*cos(THE_Psi).*cos(THE_Theta)+THE_Phi_D.*THE_Theta_D.*sin(THE_Psi).*sin(THE_Theta))-THE_Psi_D.*cos(THE_Psi).*cos(THE_Theta).*(cg_to_mot_L.*(THE_Theta_D.*sin(THE_Psi)-THE_Phi_D.*cos(THE_Psi).*cos(THE_Theta))-cg_to_mot_H.*(THE_Psi_D-THE_Phi_D.*sin(THE_Theta)))+THE_Theta_D.*sin(THE_Psi).*sin(THE_Theta).*(cg_to_mot_L.*(THE_Theta_D.*sin(THE_Psi)-THE_Phi_D.*cos(THE_Psi).*cos(THE_Theta))-cg_to_mot_H.*(THE_Psi_D-THE_Phi_D.*sin(THE_Theta)))+cg_to_mot_L.*cos(THE_Psi).*cos(THE_Theta).*(THE_Psi_D.*THE_Theta_D.*sin(THE_Psi)-THE_Phi_D.*THE_Psi_D.*cos(THE_Psi).*cos(THE_Theta)+THE_Phi_D.*THE_Theta_D.*sin(THE_Psi).*sin(THE_Theta))+THE_Theta_D.*cg_to_mot_H.*cos(THE_Theta).*(THE_Theta_D.*cos(THE_Psi)+THE_Phi_D.*cos(THE_Theta).*sin(THE_Psi))+THE_Psi_D.*cg_to_mot_L.*cos(THE_Theta).*sin(THE_Psi).*(THE_Theta_D.*cos(THE_Psi)+THE_Phi_D.*cos(THE_Theta).*sin(THE_Psi))+THE_Theta_D.*cg_to_mot_L.*cos(THE_Psi).*sin(THE_Theta).*(THE_Theta_D.*cos(THE_Psi)+THE_Phi_D.*cos(THE_Theta).*sin(THE_Psi))))./2.0-mprop.*(cos(THE_Theta).*sin(THE_Psi).*(cg_to_mot_L.*(THE_Psi_D.*THE_Theta_D.*cos(THE_Psi)+THE_Phi_D.*THE_Psi_D.*cos(THE_Theta).*sin(THE_Psi)+THE_Phi_D.*THE_Theta_D.*cos(THE_Psi).*sin(THE_Theta))-THE_Phi_D.*THE_Theta_D.*cg_to_mot_H.*cos(THE_Theta)).*(-1.0./2.0)+(cg_to_mot_H.*sin(THE_Theta).*(THE_Psi_D.*THE_Theta_D.*sin(THE_Psi)-THE_Phi_D.*THE_Psi_D.*cos(THE_Psi).*cos(THE_Theta)+THE_Phi_D.*THE_Theta_D.*sin(THE_Psi).*sin(THE_Theta)))./2.0-(THE_Psi_D.*cos(THE_Psi).*cos(THE_Theta).*(cg_to_mot_L.*(THE_Theta_D.*sin(THE_Psi)-THE_Phi_D.*cos(THE_Psi).*cos(THE_Theta))+cg_to_mot_H.*(THE_Psi_D-THE_Phi_D.*sin(THE_Theta))))./2.0+(THE_Theta_D.*sin(THE_Psi).*sin(THE_Theta).*(cg_to_mot_L.*(THE_Theta_D.*sin(THE_Psi)-THE_Phi_D.*cos(THE_Psi).*cos(THE_Theta))+cg_to_mot_H.*(THE_Psi_D-THE_Phi_D.*sin(THE_Theta))))./2.0+(cg_to_mot_L.*cos(THE_Psi).*cos(THE_Theta).*(THE_Psi_D.*THE_Theta_D.*sin(THE_Psi)-THE_Phi_D.*THE_Psi_D.*cos(THE_Psi).*cos(THE_Theta)+THE_Phi_D.*THE_Theta_D.*sin(THE_Psi).*sin(THE_Theta)))./2.0-(THE_Theta_D.*cg_to_mot_H.*cos(THE_Theta).*(THE_Theta_D.*cos(THE_Psi)+THE_Phi_D.*cos(THE_Theta).*sin(THE_Psi)))./2.0+(THE_Psi_D.*cg_to_mot_L.*cos(THE_Theta).*sin(THE_Psi).*(THE_Theta_D.*cos(THE_Psi)+THE_Phi_D.*cos(THE_Theta).*sin(THE_Psi)))./2.0+(THE_Theta_D.*cg_to_mot_L.*cos(THE_Psi).*sin(THE_Theta).*(THE_Theta_D.*cos(THE_Psi)+THE_Phi_D.*cos(THE_Theta).*sin(THE_Psi)))./2.0)+mprop.*(cos(THE_Theta).*sin(THE_Psi).*(cg_to_mot_L.*(THE_Psi_D.*THE_Theta_D.*cos(THE_Psi)+THE_Phi_D.*THE_Psi_D.*cos(THE_Theta).*sin(THE_Psi)+THE_Phi_D.*THE_Theta_D.*cos(THE_Psi).*sin(THE_Theta))+THE_Phi_D.*THE_Theta_D.*cg_to_mot_H.*cos(THE_Theta)).*(-1.0./2.0)-(cg_to_mot_H.*sin(THE_Theta).*(THE_Psi_D.*THE_Theta_D.*sin(THE_Psi)-THE_Phi_D.*THE_Psi_D.*cos(THE_Psi).*cos(THE_Theta)+THE_Phi_D.*THE_Theta_D.*sin(THE_Psi).*sin(THE_Theta)))./2.0-(THE_Psi_D.*cos(THE_Psi).*cos(THE_Theta).*(cg_to_mot_L.*(THE_Theta_D.*sin(THE_Psi)-THE_Phi_D.*cos(THE_Psi).*cos(THE_Theta))-cg_to_mot_H.*(THE_Psi_D-THE_Phi_D.*sin(THE_Theta))))./2.0+(THE_Theta_D.*sin(THE_Psi).*sin(THE_Theta).*(cg_to_mot_L.*(THE_Theta_D.*sin(THE_Psi)-THE_Phi_D.*cos(THE_Psi).*cos(THE_Theta))-cg_to_mot_H.*(THE_Psi_D-THE_Phi_D.*sin(THE_Theta))))./2.0+(cg_to_mot_L.*cos(THE_Psi).*cos(THE_Theta).*(THE_Psi_D.*THE_Theta_D.*sin(THE_Psi)-THE_Phi_D.*THE_Psi_D.*cos(THE_Psi).*cos(THE_Theta)+THE_Phi_D.*THE_Theta_D.*sin(THE_Psi).*sin(THE_Theta)))./2.0+(THE_Theta_D.*cg_to_mot_H.*cos(THE_Theta).*(THE_Theta_D.*cos(THE_Psi)+THE_Phi_D.*cos(THE_Theta).*sin(THE_Psi)))./2.0+(THE_Psi_D.*cg_to_mot_L.*cos(THE_Theta).*sin(THE_Psi).*(THE_Theta_D.*cos(THE_Psi)+THE_Phi_D.*cos(THE_Theta).*sin(THE_Psi)))./2.0+(THE_Theta_D.*cg_to_mot_L.*cos(THE_Psi).*sin(THE_Theta).*(THE_Theta_D.*cos(THE_Psi)+THE_Phi_D.*cos(THE_Theta).*sin(THE_Psi)))./2.0)-(m_pend.*((Lz_pend.*sin(THE_Theta).*(THE_Phi_pend_D.^2.*sin(THE_Phi_pend).*sin(THE_Psi_pend)+THE_Psi_pend_D.^2.*sin(THE_Phi_pend).*sin(THE_Psi_pend)+THE_Phi_pend_D.^2.*cos(THE_Phi_pend).*cos(THE_Psi_pend).*sin(THE_Theta_pend)+THE_Psi_pend_D.^2.*cos(THE_Phi_pend).*cos(THE_Psi_pend).*sin(THE_Theta_pend)+THE_Theta_pend_D.^2.*cos(THE_Phi_pend).*cos(THE_Psi_pend).*sin(THE_Theta_pend)-THE_Phi_pend_D.*THE_Psi_pend_D.*cos(THE_Phi_pend).*cos(THE_Psi_pend).*2.0+THE_Phi_pend_D.*THE_Theta_pend_D.*cos(THE_Psi_pend).*cos(THE_Theta_pend).*sin(THE_Phi_pend).*2.0+THE_Psi_pend_D.*THE_Theta_pend_D.*cos(THE_Phi_pend).*cos(THE_Theta_pend).*sin(THE_Psi_pend).*2.0-THE_Phi_pend_D.*THE_Psi_pend_D.*sin(THE_Phi_pend).*sin(THE_Psi_pend).*sin(THE_Theta_pend).*2.0))./2.0-cos(THE_Psi).*cos(THE_Theta).*((Lz_pend.*THE_Psi_pend_D.^2.*cos(THE_Psi_pend).*cos(THE_Theta_pend))./2.0+(Lz_pend.*THE_Theta_pend_D.^2.*cos(THE_Psi_pend).*cos(THE_Theta_pend))./2.0-Lz_pend.*THE_Psi_pend_D.*THE_Theta_pend_D.*sin(THE_Psi_pend).*sin(THE_Theta_pend))+(Lz_pend.*THE_Theta_D.^2.*sin(THE_Theta).*(sin(THE_Phi_pend).*sin(THE_Psi_pend)+cos(THE_Phi_pend).*cos(THE_Psi_pend).*sin(THE_Theta_pend)))./2.0-(Lz_pend.*cos(THE_Theta).*sin(THE_Psi).*(-THE_Phi_pend_D.^2.*cos(THE_Phi_pend).*sin(THE_Psi_pend)-THE_Psi_pend_D.^2.*cos(THE_Phi_pend).*sin(THE_Psi_pend)+THE_Phi_pend_D.^2.*cos(THE_Psi_pend).*sin(THE_Phi_pend).*sin(THE_Theta_pend)+THE_Psi_pend_D.^2.*cos(THE_Psi_pend).*sin(THE_Phi_pend).*sin(THE_Theta_pend)+THE_Theta_pend_D.^2.*cos(THE_Psi_pend).*sin(THE_Phi_pend).*sin(THE_Theta_pend)-THE_Phi_pend_D.*THE_Psi_pend_D.*cos(THE_Psi_pend).*sin(THE_Phi_pend).*2.0-THE_Phi_pend_D.*THE_Theta_pend_D.*cos(THE_Phi_pend).*cos(THE_Psi_pend).*cos(THE_Theta_pend).*2.0+THE_Phi_pend_D.*THE_Psi_pend_D.*cos(THE_Phi_pend).*sin(THE_Psi_pend).*sin(THE_Theta_pend).*2.0+THE_Psi_pend_D.*THE_Theta_pend_D.*cos(THE_Theta_pend).*sin(THE_Phi_pend).*sin(THE_Psi_pend).*2.0))./2.0-Lz_pend.*THE_Theta_D.*cos(THE_Theta).*(THE_Phi_pend_D.*cos(THE_Phi_pend).*sin(THE_Psi_pend)+THE_Psi_pend_D.*cos(THE_Psi_pend).*sin(THE_Phi_pend)+THE_Theta_pend_D.*cos(THE_Phi_pend).*cos(THE_Psi_pend).*cos(THE_Theta_pend)-THE_Phi_pend_D.*cos(THE_Psi_pend).*sin(THE_Phi_pend).*sin(THE_Theta_pend)-THE_Psi_pend_D.*cos(THE_Phi_pend).*sin(THE_Psi_pend).*sin(THE_Theta_pend))-THE_Psi_D.^2.*cos(THE_Psi).*cos(THE_Theta).*(Tv_Z_pend+(Lz_pend.*cos(THE_Psi_pend).*cos(THE_Theta_pend))./2.0)-THE_Theta_D.^2.*cos(THE_Psi).*cos(THE_Theta).*(Tv_Z_pend+(Lz_pend.*cos(THE_Psi_pend).*cos(THE_Theta_pend))./2.0)+THE_Psi_D.*cos(THE_Theta).*sin(THE_Psi).*((Lz_pend.*THE_Psi_pend_D.*cos(THE_Theta_pend).*sin(THE_Psi_pend))./2.0+(Lz_pend.*THE_Theta_pend_D.*cos(THE_Psi_pend).*sin(THE_Theta_pend))./2.0).*2.0+THE_Theta_D.*cos(THE_Psi).*sin(THE_Theta).*((Lz_pend.*THE_Psi_pend_D.*cos(THE_Theta_pend).*sin(THE_Psi_pend))./2.0+(Lz_pend.*THE_Theta_pend_D.*cos(THE_Psi_pend).*sin(THE_Theta_pend))./2.0).*2.0+Lz_pend.*THE_Psi_D.*cos(THE_Psi).*cos(THE_Theta).*(-THE_Psi_pend_D.*cos(THE_Phi_pend).*cos(THE_Psi_pend)+THE_Phi_pend_D.*sin(THE_Phi_pend).*sin(THE_Psi_pend)-THE_Psi_pend_D.*sin(THE_Phi_pend).*sin(THE_Psi_pend).*sin(THE_Theta_pend)+THE_Phi_pend_D.*cos(THE_Phi_pend).*cos(THE_Psi_pend).*sin(THE_Theta_pend)+THE_Theta_pend_D.*cos(THE_Psi_pend).*cos(THE_Theta_pend).*sin(THE_Phi_pend))-Lz_pend.*THE_Theta_D.*sin(THE_Psi).*sin(THE_Theta).*(-THE_Psi_pend_D.*cos(THE_Phi_pend).*cos(THE_Psi_pend)+THE_Phi_pend_D.*sin(THE_Phi_pend).*sin(THE_Psi_pend)-THE_Psi_pend_D.*sin(THE_Phi_pend).*sin(THE_Psi_pend).*sin(THE_Theta_pend)+THE_Phi_pend_D.*cos(THE_Phi_pend).*cos(THE_Psi_pend).*sin(THE_Theta_pend)+THE_Theta_pend_D.*cos(THE_Psi_pend).*cos(THE_Theta_pend).*sin(THE_Phi_pend))+THE_Psi_D.*THE_Theta_D.*sin(THE_Psi).*sin(THE_Theta).*(Tv_Z_pend+(Lz_pend.*cos(THE_Psi_pend).*cos(THE_Theta_pend))./2.0).*2.0+(Lz_pend.*THE_Psi_D.^2.*cos(THE_Theta).*sin(THE_Psi).*(cos(THE_Phi_pend).*sin(THE_Psi_pend)-cos(THE_Psi_pend).*sin(THE_Phi_pend).*sin(THE_Theta_pend)))./2.0+(Lz_pend.*THE_Theta_D.^2.*cos(THE_Theta).*sin(THE_Psi).*(cos(THE_Phi_pend).*sin(THE_Psi_pend)-cos(THE_Psi_pend).*sin(THE_Phi_pend).*sin(THE_Theta_pend)))./2.0+Lz_pend.*THE_Psi_D.*THE_Theta_D.*cos(THE_Psi).*sin(THE_Theta).*(cos(THE_Phi_pend).*sin(THE_Psi_pend)-cos(THE_Psi_pend).*sin(THE_Phi_pend).*sin(THE_Theta_pend))))./2.0-m_pend.*((Lz_pend.*sin(THE_Theta).*(THE_Phi_pend_D.^2.*sin(THE_Phi_pend).*sin(THE_Psi_pend)+THE_Psi_pend_D.^2.*sin(THE_Phi_pend).*sin(THE_Psi_pend)+THE_Phi_pend_D.^2.*cos(THE_Phi_pend).*cos(THE_Psi_pend).*sin(THE_Theta_pend)+THE_Psi_pend_D.^2.*cos(THE_Phi_pend).*cos(THE_Psi_pend).*sin(THE_Theta_pend)+THE_Theta_pend_D.^2.*cos(THE_Phi_pend).*cos(THE_Psi_pend).*sin(THE_Theta_pend)-THE_Phi_pend_D.*THE_Psi_pend_D.*cos(THE_Phi_pend).*cos(THE_Psi_pend).*2.0+THE_Phi_pend_D.*THE_Theta_pend_D.*cos(THE_Psi_pend).*cos(THE_Theta_pend).*sin(THE_Phi_pend).*2.0+THE_Psi_pend_D.*THE_Theta_pend_D.*cos(THE_Phi_pend).*cos(THE_Theta_pend).*sin(THE_Psi_pend).*2.0-THE_Phi_pend_D.*THE_Psi_pend_D.*sin(THE_Phi_pend).*sin(THE_Psi_pend).*sin(THE_Theta_pend).*2.0))./4.0-(cos(THE_Psi).*cos(THE_Theta).*((Lz_pend.*THE_Psi_pend_D.^2.*cos(THE_Psi_pend).*cos(THE_Theta_pend))./2.0+(Lz_pend.*THE_Theta_pend_D.^2.*cos(THE_Psi_pend).*cos(THE_Theta_pend))./2.0-Lz_pend.*THE_Psi_pend_D.*THE_Theta_pend_D.*sin(THE_Psi_pend).*sin(THE_Theta_pend)))./2.0+(Lz_pend.*THE_Theta_D.^2.*sin(THE_Theta).*(sin(THE_Phi_pend).*sin(THE_Psi_pend)+cos(THE_Phi_pend).*cos(THE_Psi_pend).*sin(THE_Theta_pend)))./4.0-(Lz_pend.*cos(THE_Theta).*sin(THE_Psi).*(-THE_Phi_pend_D.^2.*cos(THE_Phi_pend).*sin(THE_Psi_pend)-THE_Psi_pend_D.^2.*cos(THE_Phi_pend).*sin(THE_Psi_pend)+THE_Phi_pend_D.^2.*cos(THE_Psi_pend).*sin(THE_Phi_pend).*sin(THE_Theta_pend)+THE_Psi_pend_D.^2.*cos(THE_Psi_pend).*sin(THE_Phi_pend).*sin(THE_Theta_pend)+THE_Theta_pend_D.^2.*cos(THE_Psi_pend).*sin(THE_Phi_pend).*sin(THE_Theta_pend)-THE_Phi_pend_D.*THE_Psi_pend_D.*cos(THE_Psi_pend).*sin(THE_Phi_pend).*2.0-THE_Phi_pend_D.*THE_Theta_pend_D.*cos(THE_Phi_pend).*cos(THE_Psi_pend).*cos(THE_Theta_pend).*2.0+THE_Phi_pend_D.*THE_Psi_pend_D.*cos(THE_Phi_pend).*sin(THE_Psi_pend).*sin(THE_Theta_pend).*2.0+THE_Psi_pend_D.*THE_Theta_pend_D.*cos(THE_Theta_pend).*sin(THE_Phi_pend).*sin(THE_Psi_pend).*2.0))./4.0-(Lz_pend.*THE_Theta_D.*cos(THE_Theta).*(THE_Phi_pend_D.*cos(THE_Phi_pend).*sin(THE_Psi_pend)+THE_Psi_pend_D.*cos(THE_Psi_pend).*sin(THE_Phi_pend)+THE_Theta_pend_D.*cos(THE_Phi_pend).*cos(THE_Psi_pend).*cos(THE_Theta_pend)-THE_Phi_pend_D.*cos(THE_Psi_pend).*sin(THE_Phi_pend).*sin(THE_Theta_pend)-THE_Psi_pend_D.*cos(THE_Phi_pend).*sin(THE_Psi_pend).*sin(THE_Theta_pend)))./2.0-(THE_Psi_D.^2.*cos(THE_Psi).*cos(THE_Theta).*(Tv_Z_pend+(Lz_pend.*cos(THE_Psi_pend).*cos(THE_Theta_pend))./2.0))./2.0-(THE_Theta_D.^2.*cos(THE_Psi).*cos(THE_Theta).*(Tv_Z_pend+(Lz_pend.*cos(THE_Psi_pend).*cos(THE_Theta_pend))./2.0))./2.0+THE_Psi_D.*cos(THE_Theta).*sin(THE_Psi).*((Lz_pend.*THE_Psi_pend_D.*cos(THE_Theta_pend).*sin(THE_Psi_pend))./2.0+(Lz_pend.*THE_Theta_pend_D.*cos(THE_Psi_pend).*sin(THE_Theta_pend))./2.0)+THE_Theta_D.*cos(THE_Psi).*sin(THE_Theta).*((Lz_pend.*THE_Psi_pend_D.*cos(THE_Theta_pend).*sin(THE_Psi_pend))./2.0+(Lz_pend.*THE_Theta_pend_D.*cos(THE_Psi_pend).*sin(THE_Theta_pend))./2.0)+(Lz_pend.*THE_Psi_D.*cos(THE_Psi).*cos(THE_Theta).*(-THE_Psi_pend_D.*cos(THE_Phi_pend).*cos(THE_Psi_pend)+THE_Phi_pend_D.*sin(THE_Phi_pend).*sin(THE_Psi_pend)-THE_Psi_pend_D.*sin(THE_Phi_pend).*sin(THE_Psi_pend).*sin(THE_Theta_pend)+THE_Phi_pend_D.*cos(THE_Phi_pend).*cos(THE_Psi_pend).*sin(THE_Theta_pend)+THE_Theta_pend_D.*cos(THE_Psi_pend).*cos(THE_Theta_pend).*sin(THE_Phi_pend)))./2.0-(Lz_pend.*THE_Theta_D.*sin(THE_Psi).*sin(THE_Theta).*(-THE_Psi_pend_D.*cos(THE_Phi_pend).*cos(THE_Psi_pend)+THE_Phi_pend_D.*sin(THE_Phi_pend).*sin(THE_Psi_pend)-THE_Psi_pend_D.*sin(THE_Phi_pend).*sin(THE_Psi_pend).*sin(THE_Theta_pend)+THE_Phi_pend_D.*cos(THE_Phi_pend).*cos(THE_Psi_pend).*sin(THE_Theta_pend)+THE_Theta_pend_D.*cos(THE_Psi_pend).*cos(THE_Theta_pend).*sin(THE_Phi_pend)))./2.0+THE_Psi_D.*THE_Theta_D.*sin(THE_Psi).*sin(THE_Theta).*(Tv_Z_pend+(Lz_pend.*cos(THE_Psi_pend).*cos(THE_Theta_pend))./2.0)+(Lz_pend.*THE_Psi_D.^2.*cos(THE_Theta).*sin(THE_Psi).*(cos(THE_Phi_pend).*sin(THE_Psi_pend)-cos(THE_Psi_pend).*sin(THE_Phi_pend).*sin(THE_Theta_pend)))./4.0+(Lz_pend.*THE_Theta_D.^2.*cos(THE_Theta).*sin(THE_Psi).*(cos(THE_Phi_pend).*sin(THE_Psi_pend)-cos(THE_Psi_pend).*sin(THE_Phi_pend).*sin(THE_Theta_pend)))./4.0+(Lz_pend.*THE_Psi_D.*THE_Theta_D.*cos(THE_Psi).*sin(THE_Theta).*(cos(THE_Phi_pend).*sin(THE_Psi_pend)-cos(THE_Psi_pend).*sin(THE_Phi_pend).*sin(THE_Theta_pend)))./2.0)-(mprop.*(sin(THE_Theta).*(cg_to_mot_H.*(THE_Psi_D.*THE_Theta_D.*sin(THE_Psi)-THE_Phi_D.*THE_Psi_D.*cos(THE_Psi).*cos(THE_Theta)+THE_Phi_D.*THE_Theta_D.*sin(THE_Psi).*sin(THE_Theta))+cg_to_mot_L.*(THE_Psi_D.*THE_Theta_D.*cos(THE_Psi)+THE_Phi_D.*THE_Psi_D.*cos(THE_Theta).*sin(THE_Psi)+THE_Phi_D.*THE_Theta_D.*cos(THE_Psi).*sin(THE_Theta)))-THE_Theta_D.*cos(THE_Theta).*(cg_to_mot_H.*(THE_Theta_D.*cos(THE_Psi)+THE_Phi_D.*cos(THE_Theta).*sin(THE_Psi))-cg_to_mot_L.*(THE_Theta_D.*sin(THE_Psi)-THE_Phi_D.*cos(THE_Psi).*cos(THE_Theta)))+THE_Phi_D.*THE_Theta_D.*cg_to_mot_L.*cos(THE_Psi).*cos(THE_Theta).^2+THE_Phi_D.*THE_Theta_D.*cg_to_mot_H.*cos(THE_Theta).^2.*sin(THE_Psi)-THE_Psi_D.*cg_to_mot_H.*cos(THE_Psi).*cos(THE_Theta).*(THE_Psi_D-THE_Phi_D.*sin(THE_Theta))+THE_Psi_D.*cg_to_mot_L.*cos(THE_Theta).*sin(THE_Psi).*(THE_Psi_D-THE_Phi_D.*sin(THE_Theta))+THE_Theta_D.*cg_to_mot_L.*cos(THE_Psi).*sin(THE_Theta).*(THE_Psi_D-THE_Phi_D.*sin(THE_Theta))+THE_Theta_D.*cg_to_mot_H.*sin(THE_Psi).*sin(THE_Theta).*(THE_Psi_D-THE_Phi_D.*sin(THE_Theta))))./2.0+(mprop.*(-sin(THE_Theta).*(cg_to_mot_H.*(THE_Psi_D.*THE_Theta_D.*sin(THE_Psi)-THE_Phi_D.*THE_Psi_D.*cos(THE_Psi).*cos(THE_Theta)+THE_Phi_D.*THE_Theta_D.*sin(THE_Psi).*sin(THE_Theta))-cg_to_mot_L.*(THE_Psi_D.*THE_Theta_D.*cos(THE_Psi)+THE_Phi_D.*THE_Psi_D.*cos(THE_Theta).*sin(THE_Psi)+THE_Phi_D.*THE_Theta_D.*cos(THE_Psi).*sin(THE_Theta)))+THE_Theta_D.*cos(THE_Theta).*(cg_to_mot_H.*(THE_Theta_D.*cos(THE_Psi)+THE_Phi_D.*cos(THE_Theta).*sin(THE_Psi))+cg_to_mot_L.*(THE_Theta_D.*sin(THE_Psi)-THE_Phi_D.*cos(THE_Psi).*cos(THE_Theta)))+THE_Phi_D.*THE_Theta_D.*cg_to_mot_L.*cos(THE_Psi).*cos(THE_Theta).^2-THE_Phi_D.*THE_Theta_D.*cg_to_mot_H.*cos(THE_Theta).^2.*sin(THE_Psi)+THE_Psi_D.*cg_to_mot_H.*cos(THE_Psi).*cos(THE_Theta).*(THE_Psi_D-THE_Phi_D.*sin(THE_Theta))+THE_Psi_D.*cg_to_mot_L.*cos(THE_Theta).*sin(THE_Psi).*(THE_Psi_D-THE_Phi_D.*sin(THE_Theta))+THE_Theta_D.*cg_to_mot_L.*cos(THE_Psi).*sin(THE_Theta).*(THE_Psi_D-THE_Phi_D.*sin(THE_Theta))-THE_Theta_D.*cg_to_mot_H.*sin(THE_Psi).*sin(THE_Theta).*(THE_Psi_D-THE_Phi_D.*sin(THE_Theta))))./2.0-mprop.*((sin(THE_Theta).*(cg_to_mot_H.*(THE_Psi_D.*THE_Theta_D.*sin(THE_Psi)-THE_Phi_D.*THE_Psi_D.*cos(THE_Psi).*cos(THE_Theta)+THE_Phi_D.*THE_Theta_D.*sin(THE_Psi).*sin(THE_Theta))+cg_to_mot_L.*(THE_Psi_D.*THE_Theta_D.*cos(THE_Psi)+THE_Phi_D.*THE_Psi_D.*cos(THE_Theta).*sin(THE_Psi)+THE_Phi_D.*THE_Theta_D.*cos(THE_Psi).*sin(THE_Theta))))./2.0-(THE_Theta_D.*cos(THE_Theta).*(cg_to_mot_H.*(THE_Theta_D.*cos(THE_Psi)+THE_Phi_D.*cos(THE_Theta).*sin(THE_Psi))-cg_to_mot_L.*(THE_Theta_D.*sin(THE_Psi)-THE_Phi_D.*cos(THE_Psi).*cos(THE_Theta))))./2.0+(THE_Phi_D.*THE_Theta_D.*cg_to_mot_L.*cos(THE_Psi).*cos(THE_Theta).^2)./2.0+(THE_Phi_D.*THE_Theta_D.*cg_to_mot_H.*cos(THE_Theta).^2.*sin(THE_Psi))./2.0-(THE_Psi_D.*cg_to_mot_H.*cos(THE_Psi).*cos(THE_Theta).*(THE_Psi_D-THE_Phi_D.*sin(THE_Theta)))./2.0+(THE_Psi_D.*cg_to_mot_L.*cos(THE_Theta).*sin(THE_Psi).*(THE_Psi_D-THE_Phi_D.*sin(THE_Theta)))./2.0+(THE_Theta_D.*cg_to_mot_L.*cos(THE_Psi).*sin(THE_Theta).*(THE_Psi_D-THE_Phi_D.*sin(THE_Theta)))./2.0+(THE_Theta_D.*cg_to_mot_H.*sin(THE_Psi).*sin(THE_Theta).*(THE_Psi_D-THE_Phi_D.*sin(THE_Theta)))./2.0)+mprop.*(sin(THE_Theta).*(cg_to_mot_H.*(THE_Psi_D.*THE_Theta_D.*sin(THE_Psi)-THE_Phi_D.*THE_Psi_D.*cos(THE_Psi).*cos(THE_Theta)+THE_Phi_D.*THE_Theta_D.*sin(THE_Psi).*sin(THE_Theta))-cg_to_mot_L.*(THE_Psi_D.*THE_Theta_D.*cos(THE_Psi)+THE_Phi_D.*THE_Psi_D.*cos(THE_Theta).*sin(THE_Psi)+THE_Phi_D.*THE_Theta_D.*cos(THE_Psi).*sin(THE_Theta))).*(-1.0./2.0)+(THE_Theta_D.*cos(THE_Theta).*(cg_to_mot_H.*(THE_Theta_D.*cos(THE_Psi)+THE_Phi_D.*cos(THE_Theta).*sin(THE_Psi))+cg_to_mot_L.*(THE_Theta_D.*sin(THE_Psi)-THE_Phi_D.*cos(THE_Psi).*cos(THE_Theta))))./2.0+(THE_Phi_D.*THE_Theta_D.*cg_to_mot_L.*cos(THE_Psi).*cos(THE_Theta).^2)./2.0-(THE_Phi_D.*THE_Theta_D.*cg_to_mot_H.*cos(THE_Theta).^2.*sin(THE_Psi))./2.0+(THE_Psi_D.*cg_to_mot_H.*cos(THE_Psi).*cos(THE_Theta).*(THE_Psi_D-THE_Phi_D.*sin(THE_Theta)))./2.0+(THE_Psi_D.*cg_to_mot_L.*cos(THE_Theta).*sin(THE_Psi).*(THE_Psi_D-THE_Phi_D.*sin(THE_Theta)))./2.0+(THE_Theta_D.*cg_to_mot_L.*cos(THE_Psi).*sin(THE_Theta).*(THE_Psi_D-THE_Phi_D.*sin(THE_Theta)))./2.0-(THE_Theta_D.*cg_to_mot_H.*sin(THE_Psi).*sin(THE_Theta).*(THE_Psi_D-THE_Phi_D.*sin(THE_Theta)))./2.0)+Tbz_1.*cos(THE_Psi).*cos(THE_Theta)+Tbz_2.*cos(THE_Psi).*cos(THE_Theta)+Tbz_3.*cos(THE_Psi).*cos(THE_Theta)+Tbz_4.*cos(THE_Psi).*cos(THE_Theta);m_pend.*((Lz_pend.*sin(THE_Theta).*(cos(THE_Phi_pend).*sin(THE_Psi_pend)-cos(THE_Psi_pend).*sin(THE_Phi_pend).*sin(THE_Theta_pend)))./4.0-(Lz_pend.*cos(THE_Theta).*sin(THE_Psi).*(sin(THE_Phi_pend).*sin(THE_Psi_pend)+cos(THE_Phi_pend).*cos(THE_Psi_pend).*sin(THE_Theta_pend)))./4.0).*((Lz_pend.*sin(THE_Theta).*(THE_Phi_pend_D.^2.*sin(THE_Phi_pend).*sin(THE_Psi_pend)+THE_Psi_pend_D.^2.*sin(THE_Phi_pend).*sin(THE_Psi_pend)+THE_Phi_pend_D.^2.*cos(THE_Phi_pend).*cos(THE_Psi_pend).*sin(THE_Theta_pend)+THE_Psi_pend_D.^2.*cos(THE_Phi_pend).*cos(THE_Psi_pend).*sin(THE_Theta_pend)+THE_Theta_pend_D.^2.*cos(THE_Phi_pend).*cos(THE_Psi_pend).*sin(THE_Theta_pend)-THE_Phi_pend_D.*THE_Psi_pend_D.*cos(THE_Phi_pend).*cos(THE_Psi_pend).*2.0+THE_Phi_pend_D.*THE_Theta_pend_D.*cos(THE_Psi_pend).*cos(THE_Theta_pend).*sin(THE_Phi_pend).*2.0+THE_Psi_pend_D.*THE_Theta_pend_D.*cos(THE_Phi_pend).*cos(THE_Theta_pend).*sin(THE_Psi_pend).*2.0-THE_Phi_pend_D.*THE_Psi_pend_D.*sin(THE_Phi_pend).*sin(THE_Psi_pend).*sin(THE_Theta_pend).*2.0))./2.0-cos(THE_Psi).*cos(THE_Theta).*((Lz_pend.*THE_Psi_pend_D.^2.*cos(THE_Psi_pend).*cos(THE_Theta_pend))./2.0+(Lz_pend.*THE_Theta_pend_D.^2.*cos(THE_Psi_pend).*cos(THE_Theta_pend))./2.0-Lz_pend.*THE_Psi_pend_D.*THE_Theta_pend_D.*sin(THE_Psi_pend).*sin(THE_Theta_pend))+(Lz_pend.*THE_Theta_D.^2.*sin(THE_Theta).*(sin(THE_Phi_pend).*sin(THE_Psi_pend)+cos(THE_Phi_pend).*cos(THE_Psi_pend).*sin(THE_Theta_pend)))./2.0-(Lz_pend.*cos(THE_Theta).*sin(THE_Psi).*(-THE_Phi_pend_D.^2.*cos(THE_Phi_pend).*sin(THE_Psi_pend)-THE_Psi_pend_D.^2.*cos(THE_Phi_pend).*sin(THE_Psi_pend)+THE_Phi_pend_D.^2.*cos(THE_Psi_pend).*sin(THE_Phi_pend).*sin(THE_Theta_pend)+THE_Psi_pend_D.^2.*cos(THE_Psi_pend).*sin(THE_Phi_pend).*sin(THE_Theta_pend)+THE_Theta_pend_D.^2.*cos(THE_Psi_pend).*sin(THE_Phi_pend).*sin(THE_Theta_pend)-THE_Phi_pend_D.*THE_Psi_pend_D.*cos(THE_Psi_pend).*sin(THE_Phi_pend).*2.0-THE_Phi_pend_D.*THE_Theta_pend_D.*cos(THE_Phi_pend).*cos(THE_Psi_pend).*cos(THE_Theta_pend).*2.0+THE_Phi_pend_D.*THE_Psi_pend_D.*cos(THE_Phi_pend).*sin(THE_Psi_pend).*sin(THE_Theta_pend).*2.0+THE_Psi_pend_D.*THE_Theta_pend_D.*cos(THE_Theta_pend).*sin(THE_Phi_pend).*sin(THE_Psi_pend).*2.0))./2.0-Lz_pend.*THE_Theta_D.*cos(THE_Theta).*(THE_Phi_pend_D.*cos(THE_Phi_pend).*sin(THE_Psi_pend)+THE_Psi_pend_D.*cos(THE_Psi_pend).*sin(THE_Phi_pend)+THE_Theta_pend_D.*cos(THE_Phi_pend).*cos(THE_Psi_pend).*cos(THE_Theta_pend)-THE_Phi_pend_D.*cos(THE_Psi_pend).*sin(THE_Phi_pend).*sin(THE_Theta_pend)-THE_Psi_pend_D.*cos(THE_Phi_pend).*sin(THE_Psi_pend).*sin(THE_Theta_pend))-THE_Psi_D.^2.*cos(THE_Psi).*cos(THE_Theta).*(Tv_Z_pend+(Lz_pend.*cos(THE_Psi_pend).*cos(THE_Theta_pend))./2.0)-THE_Theta_D.^2.*cos(THE_Psi).*cos(THE_Theta).*(Tv_Z_pend+(Lz_pend.*cos(THE_Psi_pend).*cos(THE_Theta_pend))./2.0)+THE_Psi_D.*cos(THE_Theta).*sin(THE_Psi).*((Lz_pend.*THE_Psi_pend_D.*cos(THE_Theta_pend).*sin(THE_Psi_pend))./2.0+(Lz_pend.*THE_Theta_pend_D.*cos(THE_Psi_pend).*sin(THE_Theta_pend))./2.0).*2.0+THE_Theta_D.*cos(THE_Psi).*sin(THE_Theta).*((Lz_pend.*THE_Psi_pend_D.*cos(THE_Theta_pend).*sin(THE_Psi_pend))./2.0+(Lz_pend.*THE_Theta_pend_D.*cos(THE_Psi_pend).*sin(THE_Theta_pend))./2.0).*2.0+Lz_pend.*THE_Psi_D.*cos(THE_Psi).*cos(THE_Theta).*(-THE_Psi_pend_D.*cos(THE_Phi_pend).*cos(THE_Psi_pend)+THE_Phi_pend_D.*sin(THE_Phi_pend).*sin(THE_Psi_pend)-THE_Psi_pend_D.*sin(THE_Phi_pend).*sin(THE_Psi_pend).*sin(THE_Theta_pend)+THE_Phi_pend_D.*cos(THE_Phi_pend).*cos(THE_Psi_pend).*sin(THE_Theta_pend)+THE_Theta_pend_D.*cos(THE_Psi_pend).*cos(THE_Theta_pend).*sin(THE_Phi_pend))-Lz_pend.*THE_Theta_D.*sin(THE_Psi).*sin(THE_Theta).*(-THE_Psi_pend_D.*cos(THE_Phi_pend).*cos(THE_Psi_pend)+THE_Phi_pend_D.*sin(THE_Phi_pend).*sin(THE_Psi_pend)-THE_Psi_pend_D.*sin(THE_Phi_pend).*sin(THE_Psi_pend).*sin(THE_Theta_pend)+THE_Phi_pend_D.*cos(THE_Phi_pend).*cos(THE_Psi_pend).*sin(THE_Theta_pend)+THE_Theta_pend_D.*cos(THE_Psi_pend).*cos(THE_Theta_pend).*sin(THE_Phi_pend))+THE_Psi_D.*THE_Theta_D.*sin(THE_Psi).*sin(THE_Theta).*(Tv_Z_pend+(Lz_pend.*cos(THE_Psi_pend).*cos(THE_Theta_pend))./2.0).*2.0+(Lz_pend.*THE_Psi_D.^2.*cos(THE_Theta).*sin(THE_Psi).*(cos(THE_Phi_pend).*sin(THE_Psi_pend)-cos(THE_Psi_pend).*sin(THE_Phi_pend).*sin(THE_Theta_pend)))./2.0+(Lz_pend.*THE_Theta_D.^2.*cos(THE_Theta).*sin(THE_Psi).*(cos(THE_Phi_pend).*sin(THE_Psi_pend)-cos(THE_Psi_pend).*sin(THE_Phi_pend).*sin(THE_Theta_pend)))./2.0+Lz_pend.*THE_Psi_D.*THE_Theta_D.*cos(THE_Psi).*sin(THE_Theta).*(cos(THE_Phi_pend).*sin(THE_Psi_pend)-cos(THE_Psi_pend).*sin(THE_Phi_pend).*sin(THE_Theta_pend)))+m_pend.*((Lz_pend.*sin(THE_Theta).*(cos(THE_Phi_pend).*sin(THE_Psi_pend)-cos(THE_Psi_pend).*sin(THE_Phi_pend).*sin(THE_Theta_pend)))./2.0-(Lz_pend.*cos(THE_Theta).*sin(THE_Psi).*(sin(THE_Phi_pend).*sin(THE_Psi_pend)+cos(THE_Phi_pend).*cos(THE_Psi_pend).*sin(THE_Theta_pend)))./2.0).*((Lz_pend.*sin(THE_Theta).*(THE_Phi_pend_D.^2.*sin(THE_Phi_pend).*sin(THE_Psi_pend)+THE_Psi_pend_D.^2.*sin(THE_Phi_pend).*sin(THE_Psi_pend)+THE_Phi_pend_D.^2.*cos(THE_Phi_pend).*cos(THE_Psi_pend).*sin(THE_Theta_pend)+THE_Psi_pend_D.^2.*cos(THE_Phi_pend).*cos(THE_Psi_pend).*sin(THE_Theta_pend)+THE_Theta_pend_D.^2.*cos(THE_Phi_pend).*cos(THE_Psi_pend).*sin(THE_Theta_pend)-THE_Phi_pend_D.*THE_Psi_pend_D.*cos(THE_Phi_pend).*cos(THE_Psi_pend).*2.0+THE_Phi_pend_D.*THE_Theta_pend_D.*cos(THE_Psi_pend).*cos(THE_Theta_pend).*sin(THE_Phi_pend).*2.0+THE_Psi_pend_D.*THE_Theta_pend_D.*cos(THE_Phi_pend).*cos(THE_Theta_pend).*sin(THE_Psi_pend).*2.0-THE_Phi_pend_D.*THE_Psi_pend_D.*sin(THE_Phi_pend).*sin(THE_Psi_pend).*sin(THE_Theta_pend).*2.0))./4.0-(cos(THE_Psi).*cos(THE_Theta).*((Lz_pend.*THE_Psi_pend_D.^2.*cos(THE_Psi_pend).*cos(THE_Theta_pend))./2.0+(Lz_pend.*THE_Theta_pend_D.^2.*cos(THE_Psi_pend).*cos(THE_Theta_pend))./2.0-Lz_pend.*THE_Psi_pend_D.*THE_Theta_pend_D.*sin(THE_Psi_pend).*sin(THE_Theta_pend)))./2.0+(Lz_pend.*THE_Theta_D.^2.*sin(THE_Theta).*(sin(THE_Phi_pend).*sin(THE_Psi_pend)+cos(THE_Phi_pend).*cos(THE_Psi_pend).*sin(THE_Theta_pend)))./4.0-(Lz_pend.*cos(THE_Theta).*sin(THE_Psi).*(-THE_Phi_pend_D.^2.*cos(THE_Phi_pend).*sin(THE_Psi_pend)-THE_Psi_pend_D.^2.*cos(THE_Phi_pend).*sin(THE_Psi_pend)+THE_Phi_pend_D.^2.*cos(THE_Psi_pend).*sin(THE_Phi_pend).*sin(THE_Theta_pend)+THE_Psi_pend_D.^2.*cos(THE_Psi_pend).*sin(THE_Phi_pend).*sin(THE_Theta_pend)+THE_Theta_pend_D.^2.*cos(THE_Psi_pend).*sin(THE_Phi_pend).*sin(THE_Theta_pend)-THE_Phi_pend_D.*THE_Psi_pend_D.*cos(THE_Psi_pend).*sin(THE_Phi_pend).*2.0-THE_Phi_pend_D.*THE_Theta_pend_D.*cos(THE_Phi_pend).*cos(THE_Psi_pend).*cos(THE_Theta_pend).*2.0+THE_Phi_pend_D.*THE_Psi_pend_D.*cos(THE_Phi_pend).*sin(THE_Psi_pend).*sin(THE_Theta_pend).*2.0+THE_Psi_pend_D.*THE_Theta_pend_D.*cos(THE_Theta_pend).*sin(THE_Phi_pend).*sin(THE_Psi_pend).*2.0))./4.0-(Lz_pend.*THE_Theta_D.*cos(THE_Theta).*(THE_Phi_pend_D.*cos(THE_Phi_pend).*sin(THE_Psi_pend)+THE_Psi_pend_D.*cos(THE_Psi_pend).*sin(THE_Phi_pend)+THE_Theta_pend_D.*cos(THE_Phi_pend).*cos(THE_Psi_pend).*cos(THE_Theta_pend)-THE_Phi_pend_D.*cos(THE_Psi_pend).*sin(THE_Phi_pend).*sin(THE_Theta_pend)-THE_Psi_pend_D.*cos(THE_Phi_pend).*sin(THE_Psi_pend).*sin(THE_Theta_pend)))./2.0-(THE_Psi_D.^2.*cos(THE_Psi).*cos(THE_Theta).*(Tv_Z_pend+(Lz_pend.*cos(THE_Psi_pend).*cos(THE_Theta_pend))./2.0))./2.0-(THE_Theta_D.^2.*cos(THE_Psi).*cos(THE_Theta).*(Tv_Z_pend+(Lz_pend.*cos(THE_Psi_pend).*cos(THE_Theta_pend))./2.0))./2.0+THE_Psi_D.*cos(THE_Theta).*sin(THE_Psi).*((Lz_pend.*THE_Psi_pend_D.*cos(THE_Theta_pend).*sin(THE_Psi_pend))./2.0+(Lz_pend.*THE_Theta_pend_D.*cos(THE_Psi_pend).*sin(THE_Theta_pend))./2.0)+THE_Theta_D.*cos(THE_Psi).*sin(THE_Theta).*((Lz_pend.*THE_Psi_pend_D.*cos(THE_Theta_pend).*sin(THE_Psi_pend))./2.0+(Lz_pend.*THE_Theta_pend_D.*cos(THE_Psi_pend).*sin(THE_Theta_pend))./2.0)+(Lz_pend.*THE_Psi_D.*cos(THE_Psi).*cos(THE_Theta).*(-THE_Psi_pend_D.*cos(THE_Phi_pend).*cos(THE_Psi_pend)+THE_Phi_pend_D.*sin(THE_Phi_pend).*sin(THE_Psi_pend)-THE_Psi_pend_D.*sin(THE_Phi_pend).*sin(THE_Psi_pend).*sin(THE_Theta_pend)+THE_Phi_pend_D.*cos(THE_Phi_pend).*cos(THE_Psi_pend).*sin(THE_Theta_pend)+THE_Theta_pend_D.*cos(THE_Psi_pend).*cos(THE_Theta_pend).*sin(THE_Phi_pend)))./2.0-(Lz_pend.*THE_Theta_D.*sin(THE_Psi).*sin(THE_Theta).*(-THE_Psi_pend_D.*cos(THE_Phi_pend).*cos(THE_Psi_pend)+THE_Phi_pend_D.*sin(THE_Phi_pend).*sin(THE_Psi_pend)-THE_Psi_pend_D.*sin(THE_Phi_pend).*sin(THE_Psi_pend).*sin(THE_Theta_pend)+THE_Phi_pend_D.*cos(THE_Phi_pend).*cos(THE_Psi_pend).*sin(THE_Theta_pend)+THE_Theta_pend_D.*cos(THE_Psi_pend).*cos(THE_Theta_pend).*sin(THE_Phi_pend)))./2.0+THE_Psi_D.*THE_Theta_D.*sin(THE_Psi).*sin(THE_Theta).*(Tv_Z_pend+(Lz_pend.*cos(THE_Psi_pend).*cos(THE_Theta_pend))./2.0)+(Lz_pend.*THE_Psi_D.^2.*cos(THE_Theta).*sin(THE_Psi).*(cos(THE_Phi_pend).*sin(THE_Psi_pend)-cos(THE_Psi_pend).*sin(THE_Phi_pend).*sin(THE_Theta_pend)))./4.0+(Lz_pend.*THE_Theta_D.^2.*cos(THE_Theta).*sin(THE_Psi).*(cos(THE_Phi_pend).*sin(THE_Psi_pend)-cos(THE_Psi_pend).*sin(THE_Phi_pend).*sin(THE_Theta_pend)))./4.0+(Lz_pend.*THE_Psi_D.*THE_Theta_D.*cos(THE_Psi).*sin(THE_Theta).*(cos(THE_Phi_pend).*sin(THE_Psi_pend)-cos(THE_Psi_pend).*sin(THE_Phi_pend).*sin(THE_Theta_pend)))./2.0)+m_pend.*((Lz_pend.*(cos(THE_Phi).*cos(THE_Psi)+sin(THE_Phi).*sin(THE_Psi).*sin(THE_Theta)).*(sin(THE_Phi_pend).*sin(THE_Psi_pend)+cos(THE_Phi_pend).*cos(THE_Psi_pend).*sin(THE_Theta_pend)))./4.0+(Lz_pend.*cos(THE_Theta).*sin(THE_Phi).*(cos(THE_Phi_pend).*sin(THE_Psi_pend)-cos(THE_Psi_pend).*sin(THE_Phi_pend).*sin(THE_Theta_pend)))./4.0).*((Tv_Z_pend+(Lz_pend.*cos(THE_Psi_pend).*cos(THE_Theta_pend))./2.0).*(-THE_Phi_D.^2.*cos(THE_Phi).*sin(THE_Psi)-THE_Psi_D.^2.*cos(THE_Phi).*sin(THE_Psi)+THE_Phi_D.^2.*cos(THE_Psi).*sin(THE_Phi).*sin(THE_Theta)+THE_Psi_D.^2.*cos(THE_Psi).*sin(THE_Phi).*sin(THE_Theta)+THE_Theta_D.^2.*cos(THE_Psi).*sin(THE_Phi).*sin(THE_Theta)-THE_Phi_D.*THE_Psi_D.*cos(THE_Psi).*sin(THE_Phi).*2.0-THE_Phi_D.*THE_Theta_D.*cos(THE_Phi).*cos(THE_Psi).*cos(THE_Theta).*2.0+THE_Phi_D.*THE_Psi_D.*cos(THE_Phi).*sin(THE_Psi).*sin(THE_Theta).*2.0+THE_Psi_D.*THE_Theta_D.*cos(THE_Theta).*sin(THE_Phi).*sin(THE_Psi).*2.0)-(cos(THE_Phi).*sin(THE_Psi)-cos(THE_Psi).*sin(THE_Phi).*sin(THE_Theta)).*((Lz_pend.*THE_Psi_pend_D.^2.*cos(THE_Psi_pend).*cos(THE_Theta_pend))./2.0+(Lz_pend.*THE_Theta_pend_D.^2.*cos(THE_Psi_pend).*cos(THE_Theta_pend))./2.0-Lz_pend.*THE_Psi_pend_D.*THE_Theta_pend_D.*sin(THE_Psi_pend).*sin(THE_Theta_pend))+((Lz_pend.*THE_Psi_pend_D.*cos(THE_Theta_pend).*sin(THE_Psi_pend))./2.0+(Lz_pend.*THE_Theta_pend_D.*cos(THE_Psi_pend).*sin(THE_Theta_pend))./2.0).*(-THE_Psi_D.*cos(THE_Phi).*cos(THE_Psi)+THE_Phi_D.*sin(THE_Phi).*sin(THE_Psi)-THE_Psi_D.*sin(THE_Phi).*sin(THE_Psi).*sin(THE_Theta)+THE_Phi_D.*cos(THE_Phi).*cos(THE_Psi).*sin(THE_Theta)+THE_Theta_D.*cos(THE_Psi).*cos(THE_Theta).*sin(THE_Phi)).*2.0-Lz_pend.*(-THE_Psi_pend_D.*cos(THE_Phi_pend).*cos(THE_Psi_pend)+THE_Phi_pend_D.*sin(THE_Phi_pend).*sin(THE_Psi_pend)-THE_Psi_pend_D.*sin(THE_Phi_pend).*sin(THE_Psi_pend).*sin(THE_Theta_pend)+THE_Phi_pend_D.*cos(THE_Phi_pend).*cos(THE_Psi_pend).*sin(THE_Theta_pend)+THE_Theta_pend_D.*cos(THE_Psi_pend).*cos(THE_Theta_pend).*sin(THE_Phi_pend)).*(-THE_Phi_D.*cos(THE_Psi).*sin(THE_Phi)-THE_Psi_D.*cos(THE_Phi).*sin(THE_Psi)+THE_Phi_D.*cos(THE_Phi).*sin(THE_Psi).*sin(THE_Theta)+THE_Psi_D.*cos(THE_Psi).*sin(THE_Phi).*sin(THE_Theta)+THE_Theta_D.*cos(THE_Theta).*sin(THE_Phi).*sin(THE_Psi))+(Lz_pend.*(cos(THE_Phi).*cos(THE_Psi)+sin(THE_Phi).*sin(THE_Psi).*sin(THE_Theta)).*(-THE_Phi_pend_D.^2.*cos(THE_Phi_pend).*sin(THE_Psi_pend)-THE_Psi_pend_D.^2.*cos(THE_Phi_pend).*sin(THE_Psi_pend)+THE_Phi_pend_D.^2.*cos(THE_Psi_pend).*sin(THE_Phi_pend).*sin(THE_Theta_pend)+THE_Psi_pend_D.^2.*cos(THE_Psi_pend).*sin(THE_Phi_pend).*sin(THE_Theta_pend)+THE_Theta_pend_D.^2.*cos(THE_Psi_pend).*sin(THE_Phi_pend).*sin(THE_Theta_pend)-THE_Phi_pend_D.*THE_Psi_pend_D.*cos(THE_Psi_pend).*sin(THE_Phi_pend).*2.0-THE_Phi_pend_D.*THE_Theta_pend_D.*cos(THE_Phi_pend).*cos(THE_Psi_pend).*cos(THE_Theta_pend).*2.0+THE_Phi_pend_D.*THE_Psi_pend_D.*cos(THE_Phi_pend).*sin(THE_Psi_pend).*sin(THE_Theta_pend).*2.0+THE_Psi_pend_D.*THE_Theta_pend_D.*cos(THE_Theta_pend).*sin(THE_Phi_pend).*sin(THE_Psi_pend).*2.0))./2.0-(Lz_pend.*(cos(THE_Phi_pend).*sin(THE_Psi_pend)-cos(THE_Psi_pend).*sin(THE_Phi_pend).*sin(THE_Theta_pend)).*(THE_Phi_D.^2.*cos(THE_Phi).*cos(THE_Psi)+THE_Psi_D.^2.*cos(THE_Phi).*cos(THE_Psi)+THE_Phi_D.^2.*sin(THE_Phi).*sin(THE_Psi).*sin(THE_Theta)+THE_Psi_D.^2.*sin(THE_Phi).*sin(THE_Psi).*sin(THE_Theta)+THE_Theta_D.^2.*sin(THE_Phi).*sin(THE_Psi).*sin(THE_Theta)-THE_Phi_D.*THE_Psi_D.*sin(THE_Phi).*sin(THE_Psi).*2.0-THE_Phi_D.*THE_Psi_D.*cos(THE_Phi).*cos(THE_Psi).*sin(THE_Theta).*2.0-THE_Phi_D.*THE_Theta_D.*cos(THE_Phi).*cos(THE_Theta).*sin(THE_Psi).*2.0-THE_Psi_D.*THE_Theta_D.*cos(THE_Psi).*cos(THE_Theta).*sin(THE_Phi).*2.0))./2.0+(Lz_pend.*cos(THE_Theta).*sin(THE_Phi).*(THE_Phi_pend_D.^2.*sin(THE_Phi_pend).*sin(THE_Psi_pend)+THE_Psi_pend_D.^2.*sin(THE_Phi_pend).*sin(THE_Psi_pend)+THE_Phi_pend_D.^2.*cos(THE_Phi_pend).*cos(THE_Psi_pend).*sin(THE_Theta_pend)+THE_Psi_pend_D.^2.*cos(THE_Phi_pend).*cos(THE_Psi_pend).*sin(THE_Theta_pend)+THE_Theta_pend_D.^2.*cos(THE_Phi_pend).*cos(THE_Psi_pend).*sin(THE_Theta_pend)-THE_Phi_pend_D.*THE_Psi_pend_D.*cos(THE_Phi_pend).*cos(THE_Psi_pend).*2.0+THE_Phi_pend_D.*THE_Theta_pend_D.*cos(THE_Psi_pend).*cos(THE_Theta_pend).*sin(THE_Phi_pend).*2.0+THE_Psi_pend_D.*THE_Theta_pend_D.*cos(THE_Phi_pend).*cos(THE_Theta_pend).*sin(THE_Psi_pend).*2.0-THE_Phi_pend_D.*THE_Psi_pend_D.*sin(THE_Phi_pend).*sin(THE_Psi_pend).*sin(THE_Theta_pend).*2.0))./2.0-Lz_pend.*THE_Phi_D.*cos(THE_Phi).*cos(THE_Theta).*(THE_Phi_pend_D.*cos(THE_Phi_pend).*sin(THE_Psi_pend)+THE_Psi_pend_D.*cos(THE_Psi_pend).*sin(THE_Phi_pend)+THE_Theta_pend_D.*cos(THE_Phi_pend).*cos(THE_Psi_pend).*cos(THE_Theta_pend)-THE_Phi_pend_D.*cos(THE_Psi_pend).*sin(THE_Phi_pend).*sin(THE_Theta_pend)-THE_Psi_pend_D.*cos(THE_Phi_pend).*sin(THE_Psi_pend).*sin(THE_Theta_pend))+Lz_pend.*THE_Theta_D.*sin(THE_Phi).*sin(THE_Theta).*(THE_Phi_pend_D.*cos(THE_Phi_pend).*sin(THE_Psi_pend)+THE_Psi_pend_D.*cos(THE_Psi_pend).*sin(THE_Phi_pend)+THE_Theta_pend_D.*cos(THE_Phi_pend).*cos(THE_Psi_pend).*cos(THE_Theta_pend)-THE_Phi_pend_D.*cos(THE_Psi_pend).*sin(THE_Phi_pend).*sin(THE_Theta_pend)-THE_Psi_pend_D.*cos(THE_Phi_pend).*sin(THE_Psi_pend).*sin(THE_Theta_pend))+(Lz_pend.*THE_Phi_D.^2.*cos(THE_Theta).*sin(THE_Phi).*(sin(THE_Phi_pend).*sin(THE_Psi_pend)+cos(THE_Phi_pend).*cos(THE_Psi_pend).*sin(THE_Theta_pend)))./2.0+(Lz_pend.*THE_Theta_D.^2.*cos(THE_Theta).*sin(THE_Phi).*(sin(THE_Phi_pend).*sin(THE_Psi_pend)+cos(THE_Phi_pend).*cos(THE_Psi_pend).*sin(THE_Theta_pend)))./2.0+Lz_pend.*THE_Phi_D.*THE_Theta_D.*cos(THE_Phi).*sin(THE_Theta).*(sin(THE_Phi_pend).*sin(THE_Psi_pend)+cos(THE_Phi_pend).*cos(THE_Psi_pend).*sin(THE_Theta_pend)))+m_pend.*((Lz_pend.*(cos(THE_Phi).*cos(THE_Psi)+sin(THE_Phi).*sin(THE_Psi).*sin(THE_Theta)).*(sin(THE_Phi_pend).*sin(THE_Psi_pend)+cos(THE_Phi_pend).*cos(THE_Psi_pend).*sin(THE_Theta_pend)))./2.0+(Lz_pend.*cos(THE_Theta).*sin(THE_Phi).*(cos(THE_Phi_pend).*sin(THE_Psi_pend)-cos(THE_Psi_pend).*sin(THE_Phi_pend).*sin(THE_Theta_pend)))./2.0).*(((Tv_Z_pend+(Lz_pend.*cos(THE_Psi_pend).*cos(THE_Theta_pend))./2.0).*(-THE_Phi_D.^2.*cos(THE_Phi).*sin(THE_Psi)-THE_Psi_D.^2.*cos(THE_Phi).*sin(THE_Psi)+THE_Phi_D.^2.*cos(THE_Psi).*sin(THE_Phi).*sin(THE_Theta)+THE_Psi_D.^2.*cos(THE_Psi).*sin(THE_Phi).*sin(THE_Theta)+THE_Theta_D.^2.*cos(THE_Psi).*sin(THE_Phi).*sin(THE_Theta)-THE_Phi_D.*THE_Psi_D.*cos(THE_Psi).*sin(THE_Phi).*2.0-THE_Phi_D.*THE_Theta_D.*cos(THE_Phi).*cos(THE_Psi).*cos(THE_Theta).*2.0+THE_Phi_D.*THE_Psi_D.*cos(THE_Phi).*sin(THE_Psi).*sin(THE_Theta).*2.0+THE_Psi_D.*THE_Theta_D.*cos(THE_Theta).*sin(THE_Phi).*sin(THE_Psi).*2.0))./2.0-((cos(THE_Phi).*sin(THE_Psi)-cos(THE_Psi).*sin(THE_Phi).*sin(THE_Theta)).*((Lz_pend.*THE_Psi_pend_D.^2.*cos(THE_Psi_pend).*cos(THE_Theta_pend))./2.0+(Lz_pend.*THE_Theta_pend_D.^2.*cos(THE_Psi_pend).*cos(THE_Theta_pend))./2.0-Lz_pend.*THE_Psi_pend_D.*THE_Theta_pend_D.*sin(THE_Psi_pend).*sin(THE_Theta_pend)))./2.0+((Lz_pend.*THE_Psi_pend_D.*cos(THE_Theta_pend).*sin(THE_Psi_pend))./2.0+(Lz_pend.*THE_Theta_pend_D.*cos(THE_Psi_pend).*sin(THE_Theta_pend))./2.0).*(-THE_Psi_D.*cos(THE_Phi).*cos(THE_Psi)+THE_Phi_D.*sin(THE_Phi).*sin(THE_Psi)-THE_Psi_D.*sin(THE_Phi).*sin(THE_Psi).*sin(THE_Theta)+THE_Phi_D.*cos(THE_Phi).*cos(THE_Psi).*sin(THE_Theta)+THE_Theta_D.*cos(THE_Psi).*cos(THE_Theta).*sin(THE_Phi))-(Lz_pend.*(-THE_Psi_pend_D.*cos(THE_Phi_pend).*cos(THE_Psi_pend)+THE_Phi_pend_D.*sin(THE_Phi_pend).*sin(THE_Psi_pend)-THE_Psi_pend_D.*sin(THE_Phi_pend).*sin(THE_Psi_pend).*sin(THE_Theta_pend)+THE_Phi_pend_D.*cos(THE_Phi_pend).*cos(THE_Psi_pend).*sin(THE_Theta_pend)+THE_Theta_pend_D.*cos(THE_Psi_pend).*cos(THE_Theta_pend).*sin(THE_Phi_pend)).*(-THE_Phi_D.*cos(THE_Psi).*sin(THE_Phi)-THE_Psi_D.*cos(THE_Phi).*sin(THE_Psi)+THE_Phi_D.*cos(THE_Phi).*sin(THE_Psi).*sin(THE_Theta)+THE_Psi_D.*cos(THE_Psi).*sin(THE_Phi).*sin(THE_Theta)+THE_Theta_D.*cos(THE_Theta).*sin(THE_Phi).*sin(THE_Psi)))./2.0+(Lz_pend.*(cos(THE_Phi).*cos(THE_Psi)+sin(THE_Phi).*sin(THE_Psi).*sin(THE_Theta)).*(-THE_Phi_pend_D.^2.*cos(THE_Phi_pend).*sin(THE_Psi_pend)-THE_Psi_pend_D.^2.*cos(THE_Phi_pend).*sin(THE_Psi_pend)+THE_Phi_pend_D.^2.*cos(THE_Psi_pend).*sin(THE_Phi_pend).*sin(THE_Theta_pend)+THE_Psi_pend_D.^2.*cos(THE_Psi_pend).*sin(THE_Phi_pend).*sin(THE_Theta_pend)+THE_Theta_pend_D.^2.*cos(THE_Psi_pend).*sin(THE_Phi_pend).*sin(THE_Theta_pend)-THE_Phi_pend_D.*THE_Psi_pend_D.*cos(THE_Psi_pend).*sin(THE_Phi_pend).*2.0-THE_Phi_pend_D.*THE_Theta_pend_D.*cos(THE_Phi_pend).*cos(THE_Psi_pend).*cos(THE_Theta_pend).*2.0+THE_Phi_pend_D.*THE_Psi_pend_D.*cos(THE_Phi_pend).*sin(THE_Psi_pend).*sin(THE_Theta_pend).*2.0+THE_Psi_pend_D.*THE_Theta_pend_D.*cos(THE_Theta_pend).*sin(THE_Phi_pend).*sin(THE_Psi_pend).*2.0))./4.0-(Lz_pend.*(cos(THE_Phi_pend).*sin(THE_Psi_pend)-cos(THE_Psi_pend).*sin(THE_Phi_pend).*sin(THE_Theta_pend)).*(THE_Phi_D.^2.*cos(THE_Phi).*cos(THE_Psi)+THE_Psi_D.^2.*cos(THE_Phi).*cos(THE_Psi)+THE_Phi_D.^2.*sin(THE_Phi).*sin(THE_Psi).*sin(THE_Theta)+THE_Psi_D.^2.*sin(THE_Phi).*sin(THE_Psi).*sin(THE_Theta)+THE_Theta_D.^2.*sin(THE_Phi).*sin(THE_Psi).*sin(THE_Theta)-THE_Phi_D.*THE_Psi_D.*sin(THE_Phi).*sin(THE_Psi).*2.0-THE_Phi_D.*THE_Psi_D.*cos(THE_Phi).*cos(THE_Psi).*sin(THE_Theta).*2.0-THE_Phi_D.*THE_Theta_D.*cos(THE_Phi).*cos(THE_Theta).*sin(THE_Psi).*2.0-THE_Psi_D.*THE_Theta_D.*cos(THE_Psi).*cos(THE_Theta).*sin(THE_Phi).*2.0))./4.0+(Lz_pend.*cos(THE_Theta).*sin(THE_Phi).*(THE_Phi_pend_D.^2.*sin(THE_Phi_pend).*sin(THE_Psi_pend)+THE_Psi_pend_D.^2.*sin(THE_Phi_pend).*sin(THE_Psi_pend)+THE_Phi_pend_D.^2.*cos(THE_Phi_pend).*cos(THE_Psi_pend).*sin(THE_Theta_pend)+THE_Psi_pend_D.^2.*cos(THE_Phi_pend).*cos(THE_Psi_pend).*sin(THE_Theta_pend)+THE_Theta_pend_D.^2.*cos(THE_Phi_pend).*cos(THE_Psi_pend).*sin(THE_Theta_pend)-THE_Phi_pend_D.*THE_Psi_pend_D.*cos(THE_Phi_pend).*cos(THE_Psi_pend).*2.0+THE_Phi_pend_D.*THE_Theta_pend_D.*cos(THE_Psi_pend).*cos(THE_Theta_pend).*sin(THE_Phi_pend).*2.0+THE_Psi_pend_D.*THE_Theta_pend_D.*cos(THE_Phi_pend).*cos(THE_Theta_pend).*sin(THE_Psi_pend).*2.0-THE_Phi_pend_D.*THE_Psi_pend_D.*sin(THE_Phi_pend).*sin(THE_Psi_pend).*sin(THE_Theta_pend).*2.0))./4.0-(Lz_pend.*THE_Phi_D.*cos(THE_Phi).*cos(THE_Theta).*(THE_Phi_pend_D.*cos(THE_Phi_pend).*sin(THE_Psi_pend)+THE_Psi_pend_D.*cos(THE_Psi_pend).*sin(THE_Phi_pend)+THE_Theta_pend_D.*cos(THE_Phi_pend).*cos(THE_Psi_pend).*cos(THE_Theta_pend)-THE_Phi_pend_D.*cos(THE_Psi_pend).*sin(THE_Phi_pend).*sin(THE_Theta_pend)-THE_Psi_pend_D.*cos(THE_Phi_pend).*sin(THE_Psi_pend).*sin(THE_Theta_pend)))./2.0+(Lz_pend.*THE_Theta_D.*sin(THE_Phi).*sin(THE_Theta).*(THE_Phi_pend_D.*cos(THE_Phi_pend).*sin(THE_Psi_pend)+THE_Psi_pend_D.*cos(THE_Psi_pend).*sin(THE_Phi_pend)+THE_Theta_pend_D.*cos(THE_Phi_pend).*cos(THE_Psi_pend).*cos(THE_Theta_pend)-THE_Phi_pend_D.*cos(THE_Psi_pend).*sin(THE_Phi_pend).*sin(THE_Theta_pend)-THE_Psi_pend_D.*cos(THE_Phi_pend).*sin(THE_Psi_pend).*sin(THE_Theta_pend)))./2.0+(Lz_pend.*THE_Phi_D.^2.*cos(THE_Theta).*sin(THE_Phi).*(sin(THE_Phi_pend).*sin(THE_Psi_pend)+cos(THE_Phi_pend).*cos(THE_Psi_pend).*sin(THE_Theta_pend)))./4.0+(Lz_pend.*THE_Theta_D.^2.*cos(THE_Theta).*sin(THE_Phi).*(sin(THE_Phi_pend).*sin(THE_Psi_pend)+cos(THE_Phi_pend).*cos(THE_Psi_pend).*sin(THE_Theta_pend)))./4.0+(Lz_pend.*THE_Phi_D.*THE_Theta_D.*cos(THE_Phi).*sin(THE_Theta).*(sin(THE_Phi_pend).*sin(THE_Psi_pend)+cos(THE_Phi_pend).*cos(THE_Psi_pend).*sin(THE_Theta_pend)))./2.0)-m_pend.*((Lz_pend.*(cos(THE_Psi).*sin(THE_Phi)-cos(THE_Phi).*sin(THE_Psi).*sin(THE_Theta)).*(sin(THE_Phi_pend).*sin(THE_Psi_pend)+cos(THE_Phi_pend).*cos(THE_Psi_pend).*sin(THE_Theta_pend)))./4.0-(Lz_pend.*cos(THE_Phi).*cos(THE_Theta).*(cos(THE_Phi_pend).*sin(THE_Psi_pend)-cos(THE_Psi_pend).*sin(THE_Phi_pend).*sin(THE_Theta_pend)))./4.0).*((Tv_Z_pend+(Lz_pend.*cos(THE_Psi_pend).*cos(THE_Theta_pend))./2.0).*(THE_Phi_D.^2.*sin(THE_Phi).*sin(THE_Psi)+THE_Psi_D.^2.*sin(THE_Phi).*sin(THE_Psi)+THE_Phi_D.^2.*cos(THE_Phi).*cos(THE_Psi).*sin(THE_Theta)+THE_Psi_D.^2.*cos(THE_Phi).*cos(THE_Psi).*sin(THE_Theta)+THE_Theta_D.^2.*cos(THE_Phi).*cos(THE_Psi).*sin(THE_Theta)-THE_Phi_D.*THE_Psi_D.*cos(THE_Phi).*cos(THE_Psi).*2.0+THE_Phi_D.*THE_Theta_D.*cos(THE_Psi).*cos(THE_Theta).*sin(THE_Phi).*2.0+THE_Psi_D.*THE_Theta_D.*cos(THE_Phi).*cos(THE_Theta).*sin(THE_Psi).*2.0-THE_Phi_D.*THE_Psi_D.*sin(THE_Phi).*sin(THE_Psi).*sin(THE_Theta).*2.0)+(sin(THE_Phi).*sin(THE_Psi)+cos(THE_Phi).*cos(THE_Psi).*sin(THE_Theta)).*((Lz_pend.*THE_Psi_pend_D.^2.*cos(THE_Psi_pend).*cos(THE_Theta_pend))./2.0+(Lz_pend.*THE_Theta_pend_D.^2.*cos(THE_Psi_pend).*cos(THE_Theta_pend))./2.0-Lz_pend.*THE_Psi_pend_D.*THE_Theta_pend_D.*sin(THE_Psi_pend).*sin(THE_Theta_pend))+((Lz_pend.*THE_Psi_pend_D.*cos(THE_Theta_pend).*sin(THE_Psi_pend))./2.0+(Lz_pend.*THE_Theta_pend_D.*cos(THE_Psi_pend).*sin(THE_Theta_pend))./2.0).*(THE_Phi_D.*cos(THE_Phi).*sin(THE_Psi)+THE_Psi_D.*cos(THE_Psi).*sin(THE_Phi)+THE_Theta_D.*cos(THE_Phi).*cos(THE_Psi).*cos(THE_Theta)-THE_Phi_D.*cos(THE_Psi).*sin(THE_Phi).*sin(THE_Theta)-THE_Psi_D.*cos(THE_Phi).*sin(THE_Psi).*sin(THE_Theta)).*2.0-(Lz_pend.*(cos(THE_Phi_pend).*sin(THE_Psi_pend)-cos(THE_Psi_pend).*sin(THE_Phi_pend).*sin(THE_Theta_pend)).*(-THE_Phi_D.^2.*cos(THE_Psi).*sin(THE_Phi)-THE_Psi_D.^2.*cos(THE_Psi).*sin(THE_Phi)+THE_Phi_D.^2.*cos(THE_Phi).*sin(THE_Psi).*sin(THE_Theta)+THE_Psi_D.^2.*cos(THE_Phi).*sin(THE_Psi).*sin(THE_Theta)+THE_Theta_D.^2.*cos(THE_Phi).*sin(THE_Psi).*sin(THE_Theta)-THE_Phi_D.*THE_Psi_D.*cos(THE_Phi).*sin(THE_Psi).*2.0-THE_Psi_D.*THE_Theta_D.*cos(THE_Phi).*cos(THE_Psi).*cos(THE_Theta).*2.0+THE_Phi_D.*THE_Psi_D.*cos(THE_Psi).*sin(THE_Phi).*sin(THE_Theta).*2.0+THE_Phi_D.*THE_Theta_D.*cos(THE_Theta).*sin(THE_Phi).*sin(THE_Psi).*2.0))./2.0-(Lz_pend.*(cos(THE_Psi).*sin(THE_Phi)-cos(THE_Phi).*sin(THE_Psi).*sin(THE_Theta)).*(-THE_Phi_pend_D.^2.*cos(THE_Phi_pend).*sin(THE_Psi_pend)-THE_Psi_pend_D.^2.*cos(THE_Phi_pend).*sin(THE_Psi_pend)+THE_Phi_pend_D.^2.*cos(THE_Psi_pend).*sin(THE_Phi_pend).*sin(THE_Theta_pend)+THE_Psi_pend_D.^2.*cos(THE_Psi_pend).*sin(THE_Phi_pend).*sin(THE_Theta_pend)+THE_Theta_pend_D.^2.*cos(THE_Psi_pend).*sin(THE_Phi_pend).*sin(THE_Theta_pend)-THE_Phi_pend_D.*THE_Psi_pend_D.*cos(THE_Psi_pend).*sin(THE_Phi_pend).*2.0-THE_Phi_pend_D.*THE_Theta_pend_D.*cos(THE_Phi_pend).*cos(THE_Psi_pend).*cos(THE_Theta_pend).*2.0+THE_Phi_pend_D.*THE_Psi_pend_D.*cos(THE_Phi_pend).*sin(THE_Psi_pend).*sin(THE_Theta_pend).*2.0+THE_Psi_pend_D.*THE_Theta_pend_D.*cos(THE_Theta_pend).*sin(THE_Phi_pend).*sin(THE_Psi_pend).*2.0))./2.0-Lz_pend.*(-THE_Phi_D.*cos(THE_Phi).*cos(THE_Psi)+THE_Psi_D.*sin(THE_Phi).*sin(THE_Psi)-THE_Phi_D.*sin(THE_Phi).*sin(THE_Psi).*sin(THE_Theta)+THE_Psi_D.*cos(THE_Phi).*cos(THE_Psi).*sin(THE_Theta)+THE_Theta_D.*cos(THE_Phi).*cos(THE_Theta).*sin(THE_Psi)).*(-THE_Psi_pend_D.*cos(THE_Phi_pend).*cos(THE_Psi_pend)+THE_Phi_pend_D.*sin(THE_Phi_pend).*sin(THE_Psi_pend)-THE_Psi_pend_D.*sin(THE_Phi_pend).*sin(THE_Psi_pend).*sin(THE_Theta_pend)+THE_Phi_pend_D.*cos(THE_Phi_pend).*cos(THE_Psi_pend).*sin(THE_Theta_pend)+THE_Theta_pend_D.*cos(THE_Psi_pend).*cos(THE_Theta_pend).*sin(THE_Phi_pend))+(Lz_pend.*cos(THE_Phi).*cos(THE_Theta).*(THE_Phi_pend_D.^2.*sin(THE_Phi_pend).*sin(THE_Psi_pend)+THE_Psi_pend_D.^2.*sin(THE_Phi_pend).*sin(THE_Psi_pend)+THE_Phi_pend_D.^2.*cos(THE_Phi_pend).*cos(THE_Psi_pend).*sin(THE_Theta_pend)+THE_Psi_pend_D.^2.*cos(THE_Phi_pend).*cos(THE_Psi_pend).*sin(THE_Theta_pend)+THE_Theta_pend_D.^2.*cos(THE_Phi_pend).*cos(THE_Psi_pend).*sin(THE_Theta_pend)-THE_Phi_pend_D.*THE_Psi_pend_D.*cos(THE_Phi_pend).*cos(THE_Psi_pend).*2.0+THE_Phi_pend_D.*THE_Theta_pend_D.*cos(THE_Psi_pend).*cos(THE_Theta_pend).*sin(THE_Phi_pend).*2.0+THE_Psi_pend_D.*THE_Theta_pend_D.*cos(THE_Phi_pend).*cos(THE_Theta_pend).*sin(THE_Psi_pend).*2.0-THE_Phi_pend_D.*THE_Psi_pend_D.*sin(THE_Phi_pend).*sin(THE_Psi_pend).*sin(THE_Theta_pend).*2.0))./2.0+Lz_pend.*THE_Phi_D.*cos(THE_Theta).*sin(THE_Phi).*(THE_Phi_pend_D.*cos(THE_Phi_pend).*sin(THE_Psi_pend)+THE_Psi_pend_D.*cos(THE_Psi_pend).*sin(THE_Phi_pend)+THE_Theta_pend_D.*cos(THE_Phi_pend).*cos(THE_Psi_pend).*cos(THE_Theta_pend)-THE_Phi_pend_D.*cos(THE_Psi_pend).*sin(THE_Phi_pend).*sin(THE_Theta_pend)-THE_Psi_pend_D.*cos(THE_Phi_pend).*sin(THE_Psi_pend).*sin(THE_Theta_pend))+Lz_pend.*THE_Theta_D.*cos(THE_Phi).*sin(THE_Theta).*(THE_Phi_pend_D.*cos(THE_Phi_pend).*sin(THE_Psi_pend)+THE_Psi_pend_D.*cos(THE_Psi_pend).*sin(THE_Phi_pend)+THE_Theta_pend_D.*cos(THE_Phi_pend).*cos(THE_Psi_pend).*cos(THE_Theta_pend)-THE_Phi_pend_D.*cos(THE_Psi_pend).*sin(THE_Phi_pend).*sin(THE_Theta_pend)-THE_Psi_pend_D.*cos(THE_Phi_pend).*sin(THE_Psi_pend).*sin(THE_Theta_pend))+(Lz_pend.*THE_Phi_D.^2.*cos(THE_Phi).*cos(THE_Theta).*(sin(THE_Phi_pend).*sin(THE_Psi_pend)+cos(THE_Phi_pend).*cos(THE_Psi_pend).*sin(THE_Theta_pend)))./2.0+(Lz_pend.*THE_Theta_D.^2.*cos(THE_Phi).*cos(THE_Theta).*(sin(THE_Phi_pend).*sin(THE_Psi_pend)+cos(THE_Phi_pend).*cos(THE_Psi_pend).*sin(THE_Theta_pend)))./2.0-Lz_pend.*THE_Phi_D.*THE_Theta_D.*sin(THE_Phi).*sin(THE_Theta).*(sin(THE_Phi_pend).*sin(THE_Psi_pend)+cos(THE_Phi_pend).*cos(THE_Psi_pend).*sin(THE_Theta_pend)))-m_pend.*((Lz_pend.*(cos(THE_Psi).*sin(THE_Phi)-cos(THE_Phi).*sin(THE_Psi).*sin(THE_Theta)).*(sin(THE_Phi_pend).*sin(THE_Psi_pend)+cos(THE_Phi_pend).*cos(THE_Psi_pend).*sin(THE_Theta_pend)))./2.0-(Lz_pend.*cos(THE_Phi).*cos(THE_Theta).*(cos(THE_Phi_pend).*sin(THE_Psi_pend)-cos(THE_Psi_pend).*sin(THE_Phi_pend).*sin(THE_Theta_pend)))./2.0).*(((Tv_Z_pend+(Lz_pend.*cos(THE_Psi_pend).*cos(THE_Theta_pend))./2.0).*(THE_Phi_D.^2.*sin(THE_Phi).*sin(THE_Psi)+THE_Psi_D.^2.*sin(THE_Phi).*sin(THE_Psi)+THE_Phi_D.^2.*cos(THE_Phi).*cos(THE_Psi).*sin(THE_Theta)+THE_Psi_D.^2.*cos(THE_Phi).*cos(THE_Psi).*sin(THE_Theta)+THE_Theta_D.^2.*cos(THE_Phi).*cos(THE_Psi).*sin(THE_Theta)-THE_Phi_D.*THE_Psi_D.*cos(THE_Phi).*cos(THE_Psi).*2.0+THE_Phi_D.*THE_Theta_D.*cos(THE_Psi).*cos(THE_Theta).*sin(THE_Phi).*2.0+THE_Psi_D.*THE_Theta_D.*cos(THE_Phi).*cos(THE_Theta).*sin(THE_Psi).*2.0-THE_Phi_D.*THE_Psi_D.*sin(THE_Phi).*sin(THE_Psi).*sin(THE_Theta).*2.0))./2.0+((sin(THE_Phi).*sin(THE_Psi)+cos(THE_Phi).*cos(THE_Psi).*sin(THE_Theta)).*((Lz_pend.*THE_Psi_pend_D.^2.*cos(THE_Psi_pend).*cos(THE_Theta_pend))./2.0+(Lz_pend.*THE_Theta_pend_D.^2.*cos(THE_Psi_pend).*cos(THE_Theta_pend))./2.0-Lz_pend.*THE_Psi_pend_D.*THE_Theta_pend_D.*sin(THE_Psi_pend).*sin(THE_Theta_pend)))./2.0+((Lz_pend.*THE_Psi_pend_D.*cos(THE_Theta_pend).*sin(THE_Psi_pend))./2.0+(Lz_pend.*THE_Theta_pend_D.*cos(THE_Psi_pend).*sin(THE_Theta_pend))./2.0).*(THE_Phi_D.*cos(THE_Phi).*sin(THE_Psi)+THE_Psi_D.*cos(THE_Psi).*sin(THE_Phi)+THE_Theta_D.*cos(THE_Phi).*cos(THE_Psi).*cos(THE_Theta)-THE_Phi_D.*cos(THE_Psi).*sin(THE_Phi).*sin(THE_Theta)-THE_Psi_D.*cos(THE_Phi).*sin(THE_Psi).*sin(THE_Theta))-(Lz_pend.*(cos(THE_Phi_pend).*sin(THE_Psi_pend)-cos(THE_Psi_pend).*sin(THE_Phi_pend).*sin(THE_Theta_pend)).*(-THE_Phi_D.^2.*cos(THE_Psi).*sin(THE_Phi)-THE_Psi_D.^2.*cos(THE_Psi).*sin(THE_Phi)+THE_Phi_D.^2.*cos(THE_Phi).*sin(THE_Psi).*sin(THE_Theta)+THE_Psi_D.^2.*cos(THE_Phi).*sin(THE_Psi).*sin(THE_Theta)+THE_Theta_D.^2.*cos(THE_Phi).*sin(THE_Psi).*sin(THE_Theta)-THE_Phi_D.*THE_Psi_D.*cos(THE_Phi).*sin(THE_Psi).*2.0-THE_Psi_D.*THE_Theta_D.*cos(THE_Phi).*cos(THE_Psi).*cos(THE_Theta).*2.0+THE_Phi_D.*THE_Psi_D.*cos(THE_Psi).*sin(THE_Phi).*sin(THE_Theta).*2.0+THE_Phi_D.*THE_Theta_D.*cos(THE_Theta).*sin(THE_Phi).*sin(THE_Psi).*2.0))./4.0-(Lz_pend.*(cos(THE_Psi).*sin(THE_Phi)-cos(THE_Phi).*sin(THE_Psi).*sin(THE_Theta)).*(-THE_Phi_pend_D.^2.*cos(THE_Phi_pend).*sin(THE_Psi_pend)-THE_Psi_pend_D.^2.*cos(THE_Phi_pend).*sin(THE_Psi_pend)+THE_Phi_pend_D.^2.*cos(THE_Psi_pend).*sin(THE_Phi_pend).*sin(THE_Theta_pend)+THE_Psi_pend_D.^2.*cos(THE_Psi_pend).*sin(THE_Phi_pend).*sin(THE_Theta_pend)+THE_Theta_pend_D.^2.*cos(THE_Psi_pend).*sin(THE_Phi_pend).*sin(THE_Theta_pend)-THE_Phi_pend_D.*THE_Psi_pend_D.*cos(THE_Psi_pend).*sin(THE_Phi_pend).*2.0-THE_Phi_pend_D.*THE_Theta_pend_D.*cos(THE_Phi_pend).*cos(THE_Psi_pend).*cos(THE_Theta_pend).*2.0+THE_Phi_pend_D.*THE_Psi_pend_D.*cos(THE_Phi_pend).*sin(THE_Psi_pend).*sin(THE_Theta_pend).*2.0+THE_Psi_pend_D.*THE_Theta_pend_D.*cos(THE_Theta_pend).*sin(THE_Phi_pend).*sin(THE_Psi_pend).*2.0))./4.0-(Lz_pend.*(-THE_Phi_D.*cos(THE_Phi).*cos(THE_Psi)+THE_Psi_D.*sin(THE_Phi).*sin(THE_Psi)-THE_Phi_D.*sin(THE_Phi).*sin(THE_Psi).*sin(THE_Theta)+THE_Psi_D.*cos(THE_Phi).*cos(THE_Psi).*sin(THE_Theta)+THE_Theta_D.*cos(THE_Phi).*cos(THE_Theta).*sin(THE_Psi)).*(-THE_Psi_pend_D.*cos(THE_Phi_pend).*cos(THE_Psi_pend)+THE_Phi_pend_D.*sin(THE_Phi_pend).*sin(THE_Psi_pend)-THE_Psi_pend_D.*sin(THE_Phi_pend).*sin(THE_Psi_pend).*sin(THE_Theta_pend)+THE_Phi_pend_D.*cos(THE_Phi_pend).*cos(THE_Psi_pend).*sin(THE_Theta_pend)+THE_Theta_pend_D.*cos(THE_Psi_pend).*cos(THE_Theta_pend).*sin(THE_Phi_pend)))./2.0+(Lz_pend.*cos(THE_Phi).*cos(THE_Theta).*(THE_Phi_pend_D.^2.*sin(THE_Phi_pend).*sin(THE_Psi_pend)+THE_Psi_pend_D.^2.*sin(THE_Phi_pend).*sin(THE_Psi_pend)+THE_Phi_pend_D.^2.*cos(THE_Phi_pend).*cos(THE_Psi_pend).*sin(THE_Theta_pend)+THE_Psi_pend_D.^2.*cos(THE_Phi_pend).*cos(THE_Psi_pend).*sin(THE_Theta_pend)+THE_Theta_pend_D.^2.*cos(THE_Phi_pend).*cos(THE_Psi_pend).*sin(THE_Theta_pend)-THE_Phi_pend_D.*THE_Psi_pend_D.*cos(THE_Phi_pend).*cos(THE_Psi_pend).*2.0+THE_Phi_pend_D.*THE_Theta_pend_D.*cos(THE_Psi_pend).*cos(THE_Theta_pend).*sin(THE_Phi_pend).*2.0+THE_Psi_pend_D.*THE_Theta_pend_D.*cos(THE_Phi_pend).*cos(THE_Theta_pend).*sin(THE_Psi_pend).*2.0-THE_Phi_pend_D.*THE_Psi_pend_D.*sin(THE_Phi_pend).*sin(THE_Psi_pend).*sin(THE_Theta_pend).*2.0))./4.0+(Lz_pend.*THE_Phi_D.*cos(THE_Theta).*sin(THE_Phi).*(THE_Phi_pend_D.*cos(THE_Phi_pend).*sin(THE_Psi_pend)+THE_Psi_pend_D.*cos(THE_Psi_pend).*sin(THE_Phi_pend)+THE_Theta_pend_D.*cos(THE_Phi_pend).*cos(THE_Psi_pend).*cos(THE_Theta_pend)-THE_Phi_pend_D.*cos(THE_Psi_pend).*sin(THE_Phi_pend).*sin(THE_Theta_pend)-THE_Psi_pend_D.*cos(THE_Phi_pend).*sin(THE_Psi_pend).*sin(THE_Theta_pend)))./2.0+(Lz_pend.*THE_Theta_D.*cos(THE_Phi).*sin(THE_Theta).*(THE_Phi_pend_D.*cos(THE_Phi_pend).*sin(THE_Psi_pend)+THE_Psi_pend_D.*cos(THE_Psi_pend).*sin(THE_Phi_pend)+THE_Theta_pend_D.*cos(THE_Phi_pend).*cos(THE_Psi_pend).*cos(THE_Theta_pend)-THE_Phi_pend_D.*cos(THE_Psi_pend).*sin(THE_Phi_pend).*sin(THE_Theta_pend)-THE_Psi_pend_D.*cos(THE_Phi_pend).*sin(THE_Psi_pend).*sin(THE_Theta_pend)))./2.0+(Lz_pend.*THE_Phi_D.^2.*cos(THE_Phi).*cos(THE_Theta).*(sin(THE_Phi_pend).*sin(THE_Psi_pend)+cos(THE_Phi_pend).*cos(THE_Psi_pend).*sin(THE_Theta_pend)))./4.0+(Lz_pend.*THE_Theta_D.^2.*cos(THE_Phi).*cos(THE_Theta).*(sin(THE_Phi_pend).*sin(THE_Psi_pend)+cos(THE_Phi_pend).*cos(THE_Psi_pend).*sin(THE_Theta_pend)))./4.0-(Lz_pend.*THE_Phi_D.*THE_Theta_D.*sin(THE_Phi).*sin(THE_Theta).*(sin(THE_Phi_pend).*sin(THE_Psi_pend)+cos(THE_Phi_pend).*cos(THE_Psi_pend).*sin(THE_Theta_pend)))./2.0)+g.*m_pend.*((Lz_pend.*sin(THE_Theta).*(cos(THE_Phi_pend).*sin(THE_Psi_pend)-cos(THE_Psi_pend).*sin(THE_Phi_pend).*sin(THE_Theta_pend)))./2.0-(Lz_pend.*cos(THE_Theta).*sin(THE_Psi).*(sin(THE_Phi_pend).*sin(THE_Psi_pend)+cos(THE_Phi_pend).*cos(THE_Psi_pend).*sin(THE_Theta_pend)))./2.0)-m_pend.*(cos(THE_Theta_pend).*sin(THE_Phi_pend).*(THE_Psi_D-THE_Phi_D.*sin(THE_Theta))-cos(THE_Phi_pend).*cos(THE_Theta_pend).*(THE_Theta_D.*cos(THE_Psi)+THE_Phi_D.*cos(THE_Theta).*sin(THE_Psi))).*(Ly_pend.^2./1.2e+1+Lz_pend.^2./1.2e+1).*(THE_Psi_pend_D./2.0+(sin(THE_Theta_pend).*(THE_Theta_D.*sin(THE_Psi)-THE_Phi_D.*cos(THE_Psi).*cos(THE_Theta)))./2.0-(THE_Phi_pend_D.*sin(THE_Theta_pend))./2.0+(cos(THE_Theta_pend).*sin(THE_Phi_pend).*(THE_Theta_D.*cos(THE_Psi)+THE_Phi_D.*cos(THE_Theta).*sin(THE_Psi)))./2.0+(cos(THE_Phi_pend).*cos(THE_Theta_pend).*(THE_Psi_D-THE_Phi_D.*sin(THE_Theta)))./2.0)-(m_pend.*sin(THE_Theta_pend).*(Ly_pend.^2./1.2e+1+Lz_pend.^2./1.2e+1).*(-sin(THE_Theta_pend).*(THE_Psi_D.*THE_Theta_D.*cos(THE_Psi)+THE_Phi_D.*THE_Psi_D.*cos(THE_Theta).*sin(THE_Psi)+THE_Phi_D.*THE_Theta_D.*cos(THE_Psi).*sin(THE_Theta))+cos(THE_Theta_pend).*sin(THE_Phi_pend).*(THE_Psi_D.*THE_Theta_D.*sin(THE_Psi)-THE_Phi_D.*THE_Psi_D.*cos(THE_Psi).*cos(THE_Theta)+THE_Phi_D.*THE_Theta_D.*sin(THE_Psi).*sin(THE_Theta))-THE_Theta_pend_D.*cos(THE_Theta_pend).*(THE_Theta_D.*sin(THE_Psi)-THE_Phi_D.*cos(THE_Psi).*cos(THE_Theta))+THE_Phi_pend_D.*THE_Theta_pend_D.*cos(THE_Theta_pend)-THE_Phi_pend_D.*cos(THE_Phi_pend).*cos(THE_Theta_pend).*(THE_Theta_D.*cos(THE_Psi)+THE_Phi_D.*cos(THE_Theta).*sin(THE_Psi))+THE_Theta_pend_D.*sin(THE_Phi_pend).*sin(THE_Theta_pend).*(THE_Theta_D.*cos(THE_Psi)+THE_Phi_D.*cos(THE_Theta).*sin(THE_Psi))+THE_Phi_pend_D.*cos(THE_Theta_pend).*sin(THE_Phi_pend).*(THE_Psi_D-THE_Phi_D.*sin(THE_Theta))+THE_Theta_pend_D.*cos(THE_Phi_pend).*sin(THE_Theta_pend).*(THE_Psi_D-THE_Phi_D.*sin(THE_Theta))+THE_Phi_D.*THE_Theta_D.*cos(THE_Theta).*cos(THE_Phi_pend).*cos(THE_Theta_pend)))./2.0-m_pend.*sin(THE_Theta_pend).*(Ly_pend.^2./1.2e+1+Lz_pend.^2./1.2e+1).*(sin(THE_Theta_pend).*(THE_Psi_D.*THE_Theta_D.*cos(THE_Psi)+THE_Phi_D.*THE_Psi_D.*cos(THE_Theta).*sin(THE_Psi)+THE_Phi_D.*THE_Theta_D.*cos(THE_Psi).*sin(THE_Theta)).*(-1.0./2.0)+(cos(THE_Theta_pend).*sin(THE_Phi_pend).*(THE_Psi_D.*THE_Theta_D.*sin(THE_Psi)-THE_Phi_D.*THE_Psi_D.*cos(THE_Psi).*cos(THE_Theta)+THE_Phi_D.*THE_Theta_D.*sin(THE_Psi).*sin(THE_Theta)))./2.0-(THE_Theta_pend_D.*cos(THE_Theta_pend).*(THE_Theta_D.*sin(THE_Psi)-THE_Phi_D.*cos(THE_Psi).*cos(THE_Theta)))./2.0+(THE_Phi_pend_D.*THE_Theta_pend_D.*cos(THE_Theta_pend))./2.0-(THE_Phi_pend_D.*cos(THE_Phi_pend).*cos(THE_Theta_pend).*(THE_Theta_D.*cos(THE_Psi)+THE_Phi_D.*cos(THE_Theta).*sin(THE_Psi)))./2.0+(THE_Theta_pend_D.*sin(THE_Phi_pend).*sin(THE_Theta_pend).*(THE_Theta_D.*cos(THE_Psi)+THE_Phi_D.*cos(THE_Theta).*sin(THE_Psi)))./2.0+(THE_Phi_pend_D.*cos(THE_Theta_pend).*sin(THE_Phi_pend).*(THE_Psi_D-THE_Phi_D.*sin(THE_Theta)))./2.0+(THE_Theta_pend_D.*cos(THE_Phi_pend).*sin(THE_Theta_pend).*(THE_Psi_D-THE_Phi_D.*sin(THE_Theta)))./2.0+(THE_Phi_D.*THE_Theta_D.*cos(THE_Theta).*cos(THE_Phi_pend).*cos(THE_Theta_pend))./2.0)-m_pend.*((cos(THE_Theta_pend).*sin(THE_Phi_pend).*(THE_Psi_D-THE_Phi_D.*sin(THE_Theta)))./2.0-(cos(THE_Phi_pend).*cos(THE_Theta_pend).*(THE_Theta_D.*cos(THE_Psi)+THE_Phi_D.*cos(THE_Theta).*sin(THE_Psi)))./2.0).*(Ly_pend.^2./1.2e+1+Lz_pend.^2./1.2e+1).*(THE_Psi_pend_D+sin(THE_Theta_pend).*(THE_Theta_D.*sin(THE_Psi)-THE_Phi_D.*cos(THE_Psi).*cos(THE_Theta))-THE_Phi_pend_D.*sin(THE_Theta_pend)+cos(THE_Theta_pend).*sin(THE_Phi_pend).*(THE_Theta_D.*cos(THE_Psi)+THE_Phi_D.*cos(THE_Theta).*sin(THE_Psi))+cos(THE_Phi_pend).*cos(THE_Theta_pend).*(THE_Psi_D-THE_Phi_D.*sin(THE_Theta)))-m_pend.*(((sin(THE_Phi_pend).*sin(THE_Psi_pend)+cos(THE_Phi_pend).*cos(THE_Psi_pend).*sin(THE_Theta_pend)).*(THE_Theta_D.*cos(THE_Psi)+THE_Phi_D.*cos(THE_Theta).*sin(THE_Psi)))./2.0+((THE_Psi_D-THE_Phi_D.*sin(THE_Theta)).*(cos(THE_Phi_pend).*sin(THE_Psi_pend)-cos(THE_Psi_pend).*sin(THE_Phi_pend).*sin(THE_Theta_pend)))./2.0).*(Lx_pend.^2./1.2e+1+Ly_pend.^2./1.2e+1).*((cos(THE_Phi_pend).*sin(THE_Psi_pend)-cos(THE_Psi_pend).*sin(THE_Phi_pend).*sin(THE_Theta_pend)).*(THE_Theta_D.*cos(THE_Psi)+THE_Phi_D.*cos(THE_Theta).*sin(THE_Psi))-(THE_Psi_D-THE_Phi_D.*sin(THE_Theta)).*(sin(THE_Phi_pend).*sin(THE_Psi_pend)+cos(THE_Phi_pend).*cos(THE_Psi_pend).*sin(THE_Theta_pend))+THE_Theta_pend_D.*sin(THE_Psi_pend)-THE_Phi_pend_D.*cos(THE_Psi_pend).*cos(THE_Theta_pend)+cos(THE_Psi_pend).*cos(THE_Theta_pend).*(THE_Theta_D.*sin(THE_Psi)-THE_Phi_D.*cos(THE_Psi).*cos(THE_Theta)))-m_pend.*((sin(THE_Phi_pend).*sin(THE_Psi_pend)+cos(THE_Phi_pend).*cos(THE_Psi_pend).*sin(THE_Theta_pend)).*(THE_Theta_D.*cos(THE_Psi)+THE_Phi_D.*cos(THE_Theta).*sin(THE_Psi))+(THE_Psi_D-THE_Phi_D.*sin(THE_Theta)).*(cos(THE_Phi_pend).*sin(THE_Psi_pend)-cos(THE_Psi_pend).*sin(THE_Phi_pend).*sin(THE_Theta_pend))).*(Lx_pend.^2./1.2e+1+Ly_pend.^2./1.2e+1).*(((cos(THE_Phi_pend).*sin(THE_Psi_pend)-cos(THE_Psi_pend).*sin(THE_Phi_pend).*sin(THE_Theta_pend)).*(THE_Theta_D.*cos(THE_Psi)+THE_Phi_D.*cos(THE_Theta).*sin(THE_Psi)))./2.0-((THE_Psi_D-THE_Phi_D.*sin(THE_Theta)).*(sin(THE_Phi_pend).*sin(THE_Psi_pend)+cos(THE_Phi_pend).*cos(THE_Psi_pend).*sin(THE_Theta_pend)))./2.0+(THE_Theta_pend_D.*sin(THE_Psi_pend))./2.0-(THE_Phi_pend_D.*cos(THE_Psi_pend).*cos(THE_Theta_pend))./2.0+(cos(THE_Psi_pend).*cos(THE_Theta_pend).*(THE_Theta_D.*sin(THE_Psi)-THE_Phi_D.*cos(THE_Psi).*cos(THE_Theta)))./2.0)-m_pend.*(((cos(THE_Psi_pend).*sin(THE_Phi_pend)-cos(THE_Phi_pend).*sin(THE_Psi_pend).*sin(THE_Theta_pend)).*(THE_Theta_D.*cos(THE_Psi)+THE_Phi_D.*cos(THE_Theta).*sin(THE_Psi)))./2.0+((THE_Psi_D-THE_Phi_D.*sin(THE_Theta)).*(cos(THE_Phi_pend).*cos(THE_Psi_pend)+sin(THE_Phi_pend).*sin(THE_Psi_pend).*sin(THE_Theta_pend)))./2.0).*(Lx_pend.^2./1.2e+1+Lz_pend.^2./1.2e+1).*((cos(THE_Phi_pend).*cos(THE_Psi_pend)+sin(THE_Phi_pend).*sin(THE_Psi_pend).*sin(THE_Theta_pend)).*(THE_Theta_D.*cos(THE_Psi)+THE_Phi_D.*cos(THE_Theta).*sin(THE_Psi))+THE_Theta_pend_D.*cos(THE_Psi_pend)-(THE_Psi_D-THE_Phi_D.*sin(THE_Theta)).*(cos(THE_Psi_pend).*sin(THE_Phi_pend)-cos(THE_Phi_pend).*sin(THE_Psi_pend).*sin(THE_Theta_pend))+THE_Phi_pend_D.*cos(THE_Theta_pend).*sin(THE_Psi_pend)-cos(THE_Theta_pend).*sin(THE_Psi_pend).*(THE_Theta_D.*sin(THE_Psi)-THE_Phi_D.*cos(THE_Psi).*cos(THE_Theta)))-m_pend.*((cos(THE_Psi_pend).*sin(THE_Phi_pend)-cos(THE_Phi_pend).*sin(THE_Psi_pend).*sin(THE_Theta_pend)).*(THE_Theta_D.*cos(THE_Psi)+THE_Phi_D.*cos(THE_Theta).*sin(THE_Psi))+(THE_Psi_D-THE_Phi_D.*sin(THE_Theta)).*(cos(THE_Phi_pend).*cos(THE_Psi_pend)+sin(THE_Phi_pend).*sin(THE_Psi_pend).*sin(THE_Theta_pend))).*(Lx_pend.^2./1.2e+1+Lz_pend.^2./1.2e+1).*(((cos(THE_Phi_pend).*cos(THE_Psi_pend)+sin(THE_Phi_pend).*sin(THE_Psi_pend).*sin(THE_Theta_pend)).*(THE_Theta_D.*cos(THE_Psi)+THE_Phi_D.*cos(THE_Theta).*sin(THE_Psi)))./2.0+(THE_Theta_pend_D.*cos(THE_Psi_pend))./2.0-((THE_Psi_D-THE_Phi_D.*sin(THE_Theta)).*(cos(THE_Psi_pend).*sin(THE_Phi_pend)-cos(THE_Phi_pend).*sin(THE_Psi_pend).*sin(THE_Theta_pend)))./2.0+(THE_Phi_pend_D.*cos(THE_Theta_pend).*sin(THE_Psi_pend))./2.0-(cos(THE_Theta_pend).*sin(THE_Psi_pend).*(THE_Theta_D.*sin(THE_Psi)-THE_Phi_D.*cos(THE_Psi).*cos(THE_Theta)))./2.0)+(THE_Theta_pend_D.*m_pend.*cos(THE_Theta_pend).*(Ly_pend.^2./1.2e+1+Lz_pend.^2./1.2e+1).*(THE_Psi_pend_D+sin(THE_Theta_pend).*(THE_Theta_D.*sin(THE_Psi)-THE_Phi_D.*cos(THE_Psi).*cos(THE_Theta))-THE_Phi_pend_D.*sin(THE_Theta_pend)+cos(THE_Theta_pend).*sin(THE_Phi_pend).*(THE_Theta_D.*cos(THE_Psi)+THE_Phi_D.*cos(THE_Theta).*sin(THE_Psi))+cos(THE_Phi_pend).*cos(THE_Theta_pend).*(THE_Psi_D-THE_Phi_D.*sin(THE_Theta))))./2.0-(m_pend.*cos(THE_Psi_pend).*cos(THE_Theta_pend).*(Lx_pend.^2./1.2e+1+Ly_pend.^2./1.2e+1).*((THE_Theta_D.*cos(THE_Psi)+THE_Phi_D.*cos(THE_Theta).*sin(THE_Psi)).*(-THE_Psi_pend_D.*cos(THE_Phi_pend).*cos(THE_Psi_pend)+THE_Phi_pend_D.*sin(THE_Phi_pend).*sin(THE_Psi_pend)-THE_Psi_pend_D.*sin(THE_Phi_pend).*sin(THE_Psi_pend).*sin(THE_Theta_pend)+THE_Phi_pend_D.*cos(THE_Phi_pend).*cos(THE_Psi_pend).*sin(THE_Theta_pend)+THE_Theta_pend_D.*cos(THE_Psi_pend).*cos(THE_Theta_pend).*sin(THE_Phi_pend))+(THE_Psi_D-THE_Phi_D.*sin(THE_Theta)).*(THE_Phi_pend_D.*cos(THE_Phi_pend).*sin(THE_Psi_pend)+THE_Psi_pend_D.*cos(THE_Psi_pend).*sin(THE_Phi_pend)+THE_Theta_pend_D.*cos(THE_Phi_pend).*cos(THE_Psi_pend).*cos(THE_Theta_pend)-THE_Phi_pend_D.*cos(THE_Psi_pend).*sin(THE_Phi_pend).*sin(THE_Theta_pend)-THE_Psi_pend_D.*cos(THE_Phi_pend).*sin(THE_Psi_pend).*sin(THE_Theta_pend))+(cos(THE_Phi_pend).*sin(THE_Psi_pend)-cos(THE_Psi_pend).*sin(THE_Phi_pend).*sin(THE_Theta_pend)).*(THE_Psi_D.*THE_Theta_D.*sin(THE_Psi)-THE_Phi_D.*THE_Psi_D.*cos(THE_Psi).*cos(THE_Theta)+THE_Phi_D.*THE_Theta_D.*sin(THE_Psi).*sin(THE_Theta))-THE_Psi_pend_D.*THE_Theta_pend_D.*cos(THE_Psi_pend)-cos(THE_Psi_pend).*cos(THE_Theta_pend).*(THE_Psi_D.*THE_Theta_D.*cos(THE_Psi)+THE_Phi_D.*THE_Psi_D.*cos(THE_Theta).*sin(THE_Psi)+THE_Phi_D.*THE_Theta_D.*cos(THE_Psi).*sin(THE_Theta))+THE_Psi_pend_D.*cos(THE_Theta_pend).*sin(THE_Psi_pend).*(THE_Theta_D.*sin(THE_Psi)-THE_Phi_D.*cos(THE_Psi).*cos(THE_Theta))+THE_Theta_pend_D.*cos(THE_Psi_pend).*sin(THE_Theta_pend).*(THE_Theta_D.*sin(THE_Psi)-THE_Phi_D.*cos(THE_Psi).*cos(THE_Theta))-THE_Phi_pend_D.*THE_Psi_pend_D.*cos(THE_Theta_pend).*sin(THE_Psi_pend)-THE_Phi_pend_D.*THE_Theta_pend_D.*cos(THE_Psi_pend).*sin(THE_Theta_pend)-THE_Phi_D.*THE_Theta_D.*cos(THE_Theta).*(sin(THE_Phi_pend).*sin(THE_Psi_pend)+cos(THE_Phi_pend).*cos(THE_Psi_pend).*sin(THE_Theta_pend))))./2.0-m_pend.*cos(THE_Psi_pend).*cos(THE_Theta_pend).*(Lx_pend.^2./1.2e+1+Ly_pend.^2./1.2e+1).*(((THE_Theta_D.*cos(THE_Psi)+THE_Phi_D.*cos(THE_Theta).*sin(THE_Psi)).*(-THE_Psi_pend_D.*cos(THE_Phi_pend).*cos(THE_Psi_pend)+THE_Phi_pend_D.*sin(THE_Phi_pend).*sin(THE_Psi_pend)-THE_Psi_pend_D.*sin(THE_Phi_pend).*sin(THE_Psi_pend).*sin(THE_Theta_pend)+THE_Phi_pend_D.*cos(THE_Phi_pend).*cos(THE_Psi_pend).*sin(THE_Theta_pend)+THE_Theta_pend_D.*cos(THE_Psi_pend).*cos(THE_Theta_pend).*sin(THE_Phi_pend)))./2.0+((THE_Psi_D-THE_Phi_D.*sin(THE_Theta)).*(THE_Phi_pend_D.*cos(THE_Phi_pend).*sin(THE_Psi_pend)+THE_Psi_pend_D.*cos(THE_Psi_pend).*sin(THE_Phi_pend)+THE_Theta_pend_D.*cos(THE_Phi_pend).*cos(THE_Psi_pend).*cos(THE_Theta_pend)-THE_Phi_pend_D.*cos(THE_Psi_pend).*sin(THE_Phi_pend).*sin(THE_Theta_pend)-THE_Psi_pend_D.*cos(THE_Phi_pend).*sin(THE_Psi_pend).*sin(THE_Theta_pend)))./2.0+((cos(THE_Phi_pend).*sin(THE_Psi_pend)-cos(THE_Psi_pend).*sin(THE_Phi_pend).*sin(THE_Theta_pend)).*(THE_Psi_D.*THE_Theta_D.*sin(THE_Psi)-THE_Phi_D.*THE_Psi_D.*cos(THE_Psi).*cos(THE_Theta)+THE_Phi_D.*THE_Theta_D.*sin(THE_Psi).*sin(THE_Theta)))./2.0-(THE_Psi_pend_D.*THE_Theta_pend_D.*cos(THE_Psi_pend))./2.0-(cos(THE_Psi_pend).*cos(THE_Theta_pend).*(THE_Psi_D.*THE_Theta_D.*cos(THE_Psi)+THE_Phi_D.*THE_Psi_D.*cos(THE_Theta).*sin(THE_Psi)+THE_Phi_D.*THE_Theta_D.*cos(THE_Psi).*sin(THE_Theta)))./2.0+(THE_Psi_pend_D.*cos(THE_Theta_pend).*sin(THE_Psi_pend).*(THE_Theta_D.*sin(THE_Psi)-THE_Phi_D.*cos(THE_Psi).*cos(THE_Theta)))./2.0+(THE_Theta_pend_D.*cos(THE_Psi_pend).*sin(THE_Theta_pend).*(THE_Theta_D.*sin(THE_Psi)-THE_Phi_D.*cos(THE_Psi).*cos(THE_Theta)))./2.0-(THE_Phi_pend_D.*THE_Psi_pend_D.*cos(THE_Theta_pend).*sin(THE_Psi_pend))./2.0-(THE_Phi_pend_D.*THE_Theta_pend_D.*cos(THE_Psi_pend).*sin(THE_Theta_pend))./2.0-(THE_Phi_D.*THE_Theta_D.*cos(THE_Theta).*(sin(THE_Phi_pend).*sin(THE_Psi_pend)+cos(THE_Phi_pend).*cos(THE_Psi_pend).*sin(THE_Theta_pend)))./2.0)+THE_Theta_pend_D.*m_pend.*cos(THE_Theta_pend).*(Ly_pend.^2./1.2e+1+Lz_pend.^2./1.2e+1).*(THE_Psi_pend_D./2.0+(sin(THE_Theta_pend).*(THE_Theta_D.*sin(THE_Psi)-THE_Phi_D.*cos(THE_Psi).*cos(THE_Theta)))./2.0-(THE_Phi_pend_D.*sin(THE_Theta_pend))./2.0+(cos(THE_Theta_pend).*sin(THE_Phi_pend).*(THE_Theta_D.*cos(THE_Psi)+THE_Phi_D.*cos(THE_Theta).*sin(THE_Psi)))./2.0+(cos(THE_Phi_pend).*cos(THE_Theta_pend).*(THE_Psi_D-THE_Phi_D.*sin(THE_Theta)))./2.0)-(m_pend.*cos(THE_Theta_pend).*sin(THE_Psi_pend).*(Lx_pend.^2./1.2e+1+Lz_pend.^2./1.2e+1).*((THE_Theta_D.*cos(THE_Psi)+THE_Phi_D.*cos(THE_Theta).*sin(THE_Psi)).*(-THE_Phi_pend_D.*cos(THE_Psi_pend).*sin(THE_Phi_pend)-THE_Psi_pend_D.*cos(THE_Phi_pend).*sin(THE_Psi_pend)+THE_Phi_pend_D.*cos(THE_Phi_pend).*sin(THE_Psi_pend).*sin(THE_Theta_pend)+THE_Psi_pend_D.*cos(THE_Psi_pend).*sin(THE_Phi_pend).*sin(THE_Theta_pend)+THE_Theta_pend_D.*cos(THE_Theta_pend).*sin(THE_Phi_pend).*sin(THE_Psi_pend))+(THE_Psi_D-THE_Phi_D.*sin(THE_Theta)).*(-THE_Phi_pend_D.*cos(THE_Phi_pend).*cos(THE_Psi_pend)+THE_Psi_pend_D.*sin(THE_Phi_pend).*sin(THE_Psi_pend)-THE_Phi_pend_D.*sin(THE_Phi_pend).*sin(THE_Psi_pend).*sin(THE_Theta_pend)+THE_Psi_pend_D.*cos(THE_Phi_pend).*cos(THE_Psi_pend).*sin(THE_Theta_pend)+THE_Theta_pend_D.*cos(THE_Phi_pend).*cos(THE_Theta_pend).*sin(THE_Psi_pend))-(cos(THE_Phi_pend).*cos(THE_Psi_pend)+sin(THE_Phi_pend).*sin(THE_Psi_pend).*sin(THE_Theta_pend)).*(THE_Psi_D.*THE_Theta_D.*sin(THE_Psi)-THE_Phi_D.*THE_Psi_D.*cos(THE_Psi).*cos(THE_Theta)+THE_Phi_D.*THE_Theta_D.*sin(THE_Psi).*sin(THE_Theta))-cos(THE_Theta_pend).*sin(THE_Psi_pend).*(THE_Psi_D.*THE_Theta_D.*cos(THE_Psi)+THE_Phi_D.*THE_Psi_D.*cos(THE_Theta).*sin(THE_Psi)+THE_Phi_D.*THE_Theta_D.*cos(THE_Psi).*sin(THE_Theta))-THE_Psi_pend_D.*THE_Theta_pend_D.*sin(THE_Psi_pend)-THE_Psi_pend_D.*cos(THE_Psi_pend).*cos(THE_Theta_pend).*(THE_Theta_D.*sin(THE_Psi)-THE_Phi_D.*cos(THE_Psi).*cos(THE_Theta))+THE_Theta_pend_D.*sin(THE_Psi_pend).*sin(THE_Theta_pend).*(THE_Theta_D.*sin(THE_Psi)-THE_Phi_D.*cos(THE_Psi).*cos(THE_Theta))+THE_Phi_pend_D.*THE_Psi_pend_D.*cos(THE_Psi_pend).*cos(THE_Theta_pend)-THE_Phi_pend_D.*THE_Theta_pend_D.*sin(THE_Psi_pend).*sin(THE_Theta_pend)+THE_Phi_D.*THE_Theta_D.*cos(THE_Theta).*(cos(THE_Psi_pend).*sin(THE_Phi_pend)-cos(THE_Phi_pend).*sin(THE_Psi_pend).*sin(THE_Theta_pend))))./2.0-m_pend.*cos(THE_Theta_pend).*sin(THE_Psi_pend).*(Lx_pend.^2./1.2e+1+Lz_pend.^2./1.2e+1).*(((THE_Theta_D.*cos(THE_Psi)+THE_Phi_D.*cos(THE_Theta).*sin(THE_Psi)).*(-THE_Phi_pend_D.*cos(THE_Psi_pend).*sin(THE_Phi_pend)-THE_Psi_pend_D.*cos(THE_Phi_pend).*sin(THE_Psi_pend)+THE_Phi_pend_D.*cos(THE_Phi_pend).*sin(THE_Psi_pend).*sin(THE_Theta_pend)+THE_Psi_pend_D.*cos(THE_Psi_pend).*sin(THE_Phi_pend).*sin(THE_Theta_pend)+THE_Theta_pend_D.*cos(THE_Theta_pend).*sin(THE_Phi_pend).*sin(THE_Psi_pend)))./2.0+((THE_Psi_D-THE_Phi_D.*sin(THE_Theta)).*(-THE_Phi_pend_D.*cos(THE_Phi_pend).*cos(THE_Psi_pend)+THE_Psi_pend_D.*sin(THE_Phi_pend).*sin(THE_Psi_pend)-THE_Phi_pend_D.*sin(THE_Phi_pend).*sin(THE_Psi_pend).*sin(THE_Theta_pend)+THE_Psi_pend_D.*cos(THE_Phi_pend).*cos(THE_Psi_pend).*sin(THE_Theta_pend)+THE_Theta_pend_D.*cos(THE_Phi_pend).*cos(THE_Theta_pend).*sin(THE_Psi_pend)))./2.0-((cos(THE_Phi_pend).*cos(THE_Psi_pend)+sin(THE_Phi_pend).*sin(THE_Psi_pend).*sin(THE_Theta_pend)).*(THE_Psi_D.*THE_Theta_D.*sin(THE_Psi)-THE_Phi_D.*THE_Psi_D.*cos(THE_Psi).*cos(THE_Theta)+THE_Phi_D.*THE_Theta_D.*sin(THE_Psi).*sin(THE_Theta)))./2.0-(cos(THE_Theta_pend).*sin(THE_Psi_pend).*(THE_Psi_D.*THE_Theta_D.*cos(THE_Psi)+THE_Phi_D.*THE_Psi_D.*cos(THE_Theta).*sin(THE_Psi)+THE_Phi_D.*THE_Theta_D.*cos(THE_Psi).*sin(THE_Theta)))./2.0-(THE_Psi_pend_D.*THE_Theta_pend_D.*sin(THE_Psi_pend))./2.0-(THE_Psi_pend_D.*cos(THE_Psi_pend).*cos(THE_Theta_pend).*(THE_Theta_D.*sin(THE_Psi)-THE_Phi_D.*cos(THE_Psi).*cos(THE_Theta)))./2.0+(THE_Theta_pend_D.*sin(THE_Psi_pend).*sin(THE_Theta_pend).*(THE_Theta_D.*sin(THE_Psi)-THE_Phi_D.*cos(THE_Psi).*cos(THE_Theta)))./2.0+(THE_Phi_pend_D.*THE_Psi_pend_D.*cos(THE_Psi_pend).*cos(THE_Theta_pend))./2.0-(THE_Phi_pend_D.*THE_Theta_pend_D.*sin(THE_Psi_pend).*sin(THE_Theta_pend))./2.0+(THE_Phi_D.*THE_Theta_D.*cos(THE_Theta).*(cos(THE_Psi_pend).*sin(THE_Phi_pend)-cos(THE_Phi_pend).*sin(THE_Psi_pend).*sin(THE_Theta_pend)))./2.0)-(THE_Psi_pend_D.*m_pend.*cos(THE_Theta_pend).*sin(THE_Psi_pend).*(Lx_pend.^2./1.2e+1+Ly_pend.^2./1.2e+1).*((cos(THE_Phi_pend).*sin(THE_Psi_pend)-cos(THE_Psi_pend).*sin(THE_Phi_pend).*sin(THE_Theta_pend)).*(THE_Theta_D.*cos(THE_Psi)+THE_Phi_D.*cos(THE_Theta).*sin(THE_Psi))-(THE_Psi_D-THE_Phi_D.*sin(THE_Theta)).*(sin(THE_Phi_pend).*sin(THE_Psi_pend)+cos(THE_Phi_pend).*cos(THE_Psi_pend).*sin(THE_Theta_pend))+THE_Theta_pend_D.*sin(THE_Psi_pend)-THE_Phi_pend_D.*cos(THE_Psi_pend).*cos(THE_Theta_pend)+cos(THE_Psi_pend).*cos(THE_Theta_pend).*(THE_Theta_D.*sin(THE_Psi)-THE_Phi_D.*cos(THE_Psi).*cos(THE_Theta))))./2.0-THE_Psi_pend_D.*m_pend.*cos(THE_Theta_pend).*sin(THE_Psi_pend).*(Lx_pend.^2./1.2e+1+Ly_pend.^2./1.2e+1).*(((cos(THE_Phi_pend).*sin(THE_Psi_pend)-cos(THE_Psi_pend).*sin(THE_Phi_pend).*sin(THE_Theta_pend)).*(THE_Theta_D.*cos(THE_Psi)+THE_Phi_D.*cos(THE_Theta).*sin(THE_Psi)))./2.0-((THE_Psi_D-THE_Phi_D.*sin(THE_Theta)).*(sin(THE_Phi_pend).*sin(THE_Psi_pend)+cos(THE_Phi_pend).*cos(THE_Psi_pend).*sin(THE_Theta_pend)))./2.0+(THE_Theta_pend_D.*sin(THE_Psi_pend))./2.0-(THE_Phi_pend_D.*cos(THE_Psi_pend).*cos(THE_Theta_pend))./2.0+(cos(THE_Psi_pend).*cos(THE_Theta_pend).*(THE_Theta_D.*sin(THE_Psi)-THE_Phi_D.*cos(THE_Psi).*cos(THE_Theta)))./2.0)-(THE_Theta_pend_D.*m_pend.*cos(THE_Psi_pend).*sin(THE_Theta_pend).*(Lx_pend.^2./1.2e+1+Ly_pend.^2./1.2e+1).*((cos(THE_Phi_pend).*sin(THE_Psi_pend)-cos(THE_Psi_pend).*sin(THE_Phi_pend).*sin(THE_Theta_pend)).*(THE_Theta_D.*cos(THE_Psi)+THE_Phi_D.*cos(THE_Theta).*sin(THE_Psi))-(THE_Psi_D-THE_Phi_D.*sin(THE_Theta)).*(sin(THE_Phi_pend).*sin(THE_Psi_pend)+cos(THE_Phi_pend).*cos(THE_Psi_pend).*sin(THE_Theta_pend))+THE_Theta_pend_D.*sin(THE_Psi_pend)-THE_Phi_pend_D.*cos(THE_Psi_pend).*cos(THE_Theta_pend)+cos(THE_Psi_pend).*cos(THE_Theta_pend).*(THE_Theta_D.*sin(THE_Psi)-THE_Phi_D.*cos(THE_Psi).*cos(THE_Theta))))./2.0-THE_Theta_pend_D.*m_pend.*cos(THE_Psi_pend).*sin(THE_Theta_pend).*(Lx_pend.^2./1.2e+1+Ly_pend.^2./1.2e+1).*(((cos(THE_Phi_pend).*sin(THE_Psi_pend)-cos(THE_Psi_pend).*sin(THE_Phi_pend).*sin(THE_Theta_pend)).*(THE_Theta_D.*cos(THE_Psi)+THE_Phi_D.*cos(THE_Theta).*sin(THE_Psi)))./2.0-((THE_Psi_D-THE_Phi_D.*sin(THE_Theta)).*(sin(THE_Phi_pend).*sin(THE_Psi_pend)+cos(THE_Phi_pend).*cos(THE_Psi_pend).*sin(THE_Theta_pend)))./2.0+(THE_Theta_pend_D.*sin(THE_Psi_pend))./2.0-(THE_Phi_pend_D.*cos(THE_Psi_pend).*cos(THE_Theta_pend))./2.0+(cos(THE_Psi_pend).*cos(THE_Theta_pend).*(THE_Theta_D.*sin(THE_Psi)-THE_Phi_D.*cos(THE_Psi).*cos(THE_Theta)))./2.0)-(THE_Psi_pend_D.*m_pend.*cos(THE_Psi_pend).*cos(THE_Theta_pend).*(Lx_pend.^2./1.2e+1+Lz_pend.^2./1.2e+1).*((cos(THE_Phi_pend).*cos(THE_Psi_pend)+sin(THE_Phi_pend).*sin(THE_Psi_pend).*sin(THE_Theta_pend)).*(THE_Theta_D.*cos(THE_Psi)+THE_Phi_D.*cos(THE_Theta).*sin(THE_Psi))+THE_Theta_pend_D.*cos(THE_Psi_pend)-(THE_Psi_D-THE_Phi_D.*sin(THE_Theta)).*(cos(THE_Psi_pend).*sin(THE_Phi_pend)-cos(THE_Phi_pend).*sin(THE_Psi_pend).*sin(THE_Theta_pend))+THE_Phi_pend_D.*cos(THE_Theta_pend).*sin(THE_Psi_pend)-cos(THE_Theta_pend).*sin(THE_Psi_pend).*(THE_Theta_D.*sin(THE_Psi)-THE_Phi_D.*cos(THE_Psi).*cos(THE_Theta))))./2.0-THE_Psi_pend_D.*m_pend.*cos(THE_Psi_pend).*cos(THE_Theta_pend).*(Lx_pend.^2./1.2e+1+Lz_pend.^2./1.2e+1).*(((cos(THE_Phi_pend).*cos(THE_Psi_pend)+sin(THE_Phi_pend).*sin(THE_Psi_pend).*sin(THE_Theta_pend)).*(THE_Theta_D.*cos(THE_Psi)+THE_Phi_D.*cos(THE_Theta).*sin(THE_Psi)))./2.0+(THE_Theta_pend_D.*cos(THE_Psi_pend))./2.0-((THE_Psi_D-THE_Phi_D.*sin(THE_Theta)).*(cos(THE_Psi_pend).*sin(THE_Phi_pend)-cos(THE_Phi_pend).*sin(THE_Psi_pend).*sin(THE_Theta_pend)))./2.0+(THE_Phi_pend_D.*cos(THE_Theta_pend).*sin(THE_Psi_pend))./2.0-(cos(THE_Theta_pend).*sin(THE_Psi_pend).*(THE_Theta_D.*sin(THE_Psi)-THE_Phi_D.*cos(THE_Psi).*cos(THE_Theta)))./2.0)+(THE_Theta_pend_D.*m_pend.*sin(THE_Psi_pend).*sin(THE_Theta_pend).*(Lx_pend.^2./1.2e+1+Lz_pend.^2./1.2e+1).*((cos(THE_Phi_pend).*cos(THE_Psi_pend)+sin(THE_Phi_pend).*sin(THE_Psi_pend).*sin(THE_Theta_pend)).*(THE_Theta_D.*cos(THE_Psi)+THE_Phi_D.*cos(THE_Theta).*sin(THE_Psi))+THE_Theta_pend_D.*cos(THE_Psi_pend)-(THE_Psi_D-THE_Phi_D.*sin(THE_Theta)).*(cos(THE_Psi_pend).*sin(THE_Phi_pend)-cos(THE_Phi_pend).*sin(THE_Psi_pend).*sin(THE_Theta_pend))+THE_Phi_pend_D.*cos(THE_Theta_pend).*sin(THE_Psi_pend)-cos(THE_Theta_pend).*sin(THE_Psi_pend).*(THE_Theta_D.*sin(THE_Psi)-THE_Phi_D.*cos(THE_Psi).*cos(THE_Theta))))./2.0+THE_Theta_pend_D.*m_pend.*sin(THE_Psi_pend).*sin(THE_Theta_pend).*(Lx_pend.^2./1.2e+1+Lz_pend.^2./1.2e+1).*(((cos(THE_Phi_pend).*cos(THE_Psi_pend)+sin(THE_Phi_pend).*sin(THE_Psi_pend).*sin(THE_Theta_pend)).*(THE_Theta_D.*cos(THE_Psi)+THE_Phi_D.*cos(THE_Theta).*sin(THE_Psi)))./2.0+(THE_Theta_pend_D.*cos(THE_Psi_pend))./2.0-((THE_Psi_D-THE_Phi_D.*sin(THE_Theta)).*(cos(THE_Psi_pend).*sin(THE_Phi_pend)-cos(THE_Phi_pend).*sin(THE_Psi_pend).*sin(THE_Theta_pend)))./2.0+(THE_Phi_pend_D.*cos(THE_Theta_pend).*sin(THE_Psi_pend))./2.0-(cos(THE_Theta_pend).*sin(THE_Psi_pend).*(THE_Theta_D.*sin(THE_Psi)-THE_Phi_D.*cos(THE_Psi).*cos(THE_Theta)))./2.0);